simulink model "Sim118Bus_Sg"  (R2020b)
(part 1 of 2)
settings: Solver=FixedStepAuto  StartTime=0  StopTime=5  FixedStep=Ts  RelTol=1e-3
undefined symbols (not defined in the file or in its folder): ApparatusDiscreDamping, ApparatusPara, ApparatusPowerFlow, ApparatusType, Fbase, OtherInputs, Sbase, Ts, Vbase, Wbase, x_e, Ybase, Zbase
libraries: powerlib x486, SimplusGT x172
settings Model: Creator=admin_user  LastModifiedBy=admin_user

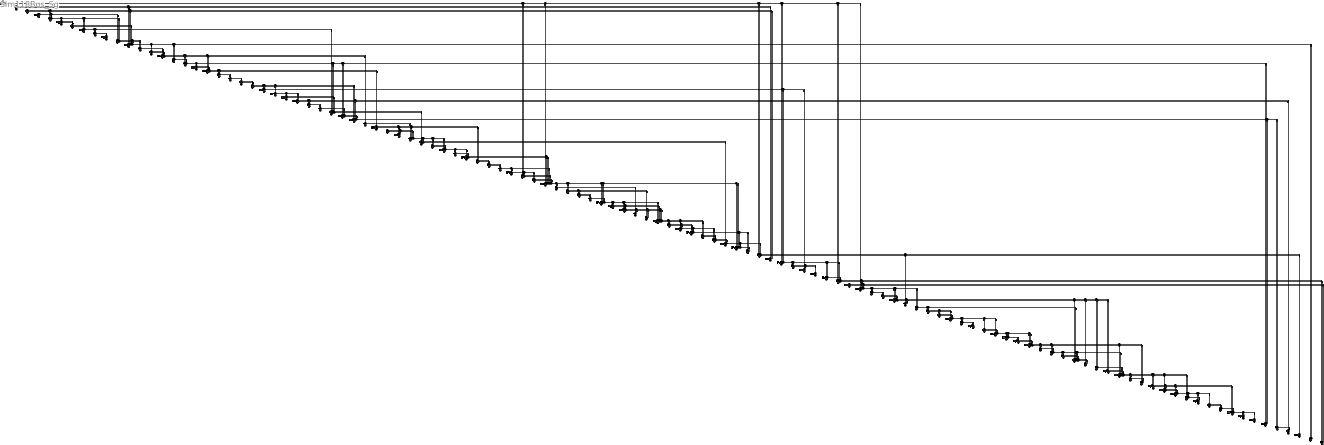
== system Sim118Bus_Sg ==
  B-GND{1,8,11,15,18,22,24,26,29,31..32,35,39,41,43,47,49,54,56,59,61,63,65,69,72,75,77,81,83,85,87,89,92,94,98,101..102,106,108,110,113,115,118,120,122,125,128,130,132,139,141,144,146,148,152,155,160..162,166,169,172,175,177,179,182,184..185,188..189,193,196..198,200,203,206,211,213,215,221..222,225,228,230,234,236..237,239,244,246,248,253,255,259,261,263..264,266,268,273,275..276,280,282,286,288..289,291,293,296..299,301..304} (118 alike) : powerlib/Elements/Ground  LConnTagsString=a
  Branch1-1 : powerlib/Elements/Three-Phase Parallel RLC Branch  LConnTagsString=A|B|C  RConnTagsString=A|B|C  BranchType=C  Resistance=(Inf)*Zbase  Inductance=(Inf)*Zbase/Wbase  Capacitance=(0.25176)*Ybase/Wbase  Measurements=None
      settings: SourceProductBaseCode=PS
  Branch1-47 : powerlib/Elements/Three-Phase Series RLC Branch  LConnTagsString=A|B|C  RConnTagsString=A|B|C  BranchType=RL  Resistance=(0.0844)*Zbase  Inductance=(0.2778)*Zbase/Wbase  Capacitance=1e-6  Measurements=None
  Branch1-49 : powerlib/Elements/Three-Phase Series RLC Branch  LConnTagsString=A|B|C  RConnTagsString=A|B|C  BranchType=RL  Resistance=(0.0985)*Zbase  Inductance=(0.324)*Zbase/Wbase  Capacitance=1e-6  Measurements=None
  Branch1-68 : powerlib/Elements/Three-Phase Series RLC Branch  LConnTagsString=A|B|C  RConnTagsString=A|B|C  BranchType=RL  Resistance=(0.0032346)*Zbase  Inductance=(0.032346)*Zbase/Wbase  Capacitance=1e-6  Measurements=None
  Branch1-70 : powerlib/Elements/Three-Phase Series RLC Branch  LConnTagsString=A|B|C  RConnTagsString=A|B|C  BranchType=RL  Resistance=(0.03)*Zbase  Inductance=(0.127)*Zbase/Wbase  Capacitance=1e-6  Measurements=None
  Branch1-75 : powerlib/Elements/Three-Phase Series RLC Branch  LConnTagsString=A|B|C  RConnTagsString=A|B|C  BranchType=RL  Resistance=(0.0405)*Zbase  Inductance=(0.122)*Zbase/Wbase  Capacitance=1e-6  Measurements=None
  Branch1-77 : powerlib/Elements/Three-Phase Series RLC Branch  LConnTagsString=A|B|C  RConnTagsString=A|B|C  BranchType=RL  Resistance=(0.0309)*Zbase  Inductance=(0.101)*Zbase/Wbase  Capacitance=1e-6  Measurements=None
  Branch10-10 : powerlib/Elements/Three-Phase Parallel RLC Branch  LConnTagsString=A|B|C  RConnTagsString=A|B|C  BranchType=C  Resistance=(Inf)*Zbase  Inductance=(Inf)*Zbase/Wbase  Capacitance=(0.615)*Ybase/Wbase  Measurements=None
      settings: SourceProductBaseCode=PS
  Branch100-100 : powerlib/Elements/Three-Phase Parallel RLC Branch  LConnTagsString=A|B|C  RConnTagsString=A|B|C  BranchType=RLC  Resistance=(2.7954)*Zbase  Inductance=(5.746)*Zbase/Wbase  Capacitance=(0.18965)*Ybase/Wbase  Measurements=None
      settings: SourceProductBaseCode=PS
  Branch100-101 : powerlib/Elements/Three-Phase Series RLC Branch  LConnTagsString=A|B|C  RConnTagsString=A|B|C  BranchType=RL  Resistance=(0.0277)*Zbase  Inductance=(0.1262)*Zbase/Wbase  Capacitance=1e-6  Measurements=None
  Branch100-103 : powerlib/Elements/Three-Phase Series RLC Branch  LConnTagsString=A|B|C  RConnTagsString=A|B|C  BranchType=RL  Resistance=(0.016)*Zbase  Inductance=(0.0525)*Zbase/Wbase  Capacitance=1e-6  Measurements=None
  Branch100-104 : powerlib/Elements/Three-Phase Series RLC Branch  LConnTagsString=A|B|C  RConnTagsString=A|B|C  BranchType=RL  Resistance=(0.0451)*Zbase  Inductance=(0.204)*Zbase/Wbase  Capacitance=1e-6  Measurements=None
  Branch100-106 : powerlib/Elements/Three-Phase Series RLC Branch  LConnTagsString=A|B|C  RConnTagsString=A|B|C  BranchType=RL  Resistance=(0.0605)*Zbase  Inductance=(0.229)*Zbase/Wbase  Capacitance=1e-6  Measurements=None
  Branch101-101 : powerlib/Elements/Three-Phase Parallel RLC Branch  LConnTagsString=A|B|C  RConnTagsString=A|B|C  BranchType=RLC  Resistance=(4.4798)*Zbase  Inductance=(6.5704)*Zbase/Wbase  Capacitance=(0.0311)*Ybase/Wbase  Measurements=None
      settings: SourceProductBaseCode=PS
  Branch101-102 : powerlib/Elements/Three-Phase Series RLC Branch  LConnTagsString=A|B|C  RConnTagsString=A|B|C  BranchType=RL  Resistance=(0.0246)*Zbase  Inductance=(0.112)*Zbase/Wbase  Capacitance=1e-6  Measurements=None
  Branch102-102 : powerlib/Elements/Three-Phase Parallel RLC Branch  LConnTagsString=A|B|C  RConnTagsString=A|B|C  BranchType=RLC  Resistance=(19.6651)*Zbase  Inductance=(32.7751)*Zbase/Wbase  Capacitance=(0.02202)*Ybase/Wbase  Measurements=None
      settings: SourceProductBaseCode=PS
  Branch103-103 : powerlib/Elements/Three-Phase Parallel RLC Branch  LConnTagsString=A|B|C  RConnTagsString=A|B|C  BranchType=RLC  Resistance=(4.2699)*Zbase  Inductance=(6.138)*Zbase/Wbase  Capacitance=(0.0906)*Ybase/Wbase  Measurements=None
      settings: SourceProductBaseCode=PS
  Branch103-104 : powerlib/Elements/Three-Phase Series RLC Branch  LConnTagsString=A|B|C  RConnTagsString=A|B|C  BranchType=RL  Resistance=(0.0466)*Zbase  Inductance=(0.1584)*Zbase/Wbase  Capacitance=1e-6  Measurements=None
  Branch103-105 : powerlib/Elements/Three-Phase Series RLC Branch  LConnTagsString=A|B|C  RConnTagsString=A|B|C  BranchType=RL  Resistance=(0.0535)*Zbase  Inductance=(0.1625)*Zbase/Wbase  Capacitance=1e-6  Measurements=None
  Branch103-110 : powerlib/Elements/Three-Phase Series RLC Branch  LConnTagsString=A|B|C  RConnTagsString=A|B|C  BranchType=RL  Resistance=(0.03906)*Zbase  Inductance=(0.1813)*Zbase/Wbase  Capacitance=1e-6  Measurements=None
  Branch104-104 : powerlib/Elements/Three-Phase Parallel RLC Branch  LConnTagsString=A|B|C  RConnTagsString=A|B|C  BranchType=RLC  Resistance=(2.4812)*Zbase  Inductance=(3.7714)*Zbase/Wbase  Capacitance=(0.05233)*Ybase/Wbase  Measurements=None
      settings: SourceProductBaseCode=PS
  Branch104-105 : powerlib/Elements/Three-Phase Series RLC Branch  LConnTagsString=A|B|C  RConnTagsString=A|B|C  BranchType=RL  Resistance=(0.00994)*Zbase  Inductance=(0.0378)*Zbase/Wbase  Capacitance=1e-6  Measurements=None
  Branch105-105 : powerlib/Elements/Three-Phase Parallel RLC Branch  LConnTagsString=A|B|C  RConnTagsString=A|B|C  BranchType=RLC  Resistance=(3.004)*Zbase  Inductance=(3.5816)*Zbase/Wbase  Capacitance=(0.06532)*Ybase/Wbase  Measurements=None
      settings: SourceProductBaseCode=PS
  Branch105-106 : powerlib/Elements/Three-Phase Series RLC Branch  LConnTagsString=A|B|C  RConnTagsString=A|B|C  BranchType=RL  Resistance=(0.014)*Zbase  Inductance=(0.0547)*Zbase/Wbase  Capacitance=1e-6  Measurements=None
  Branch105-107 : powerlib/Elements/Three-Phase Series RLC Branch  LConnTagsString=A|B|C  RConnTagsString=A|B|C  BranchType=RL  Resistance=(0.053)*Zbase  Inductance=(0.183)*Zbase/Wbase  Capacitance=1e-6  Measurements=None
  Branch105-108 : powerlib/Elements/Three-Phase Series RLC Branch  LConnTagsString=A|B|C  RConnTagsString=A|B|C  BranchType=RL  Resistance=(0.0261)*Zbase  Inductance=(0.0703)*Zbase/Wbase  Capacitance=1e-6  Measurements=None
  Branch106-106 : powerlib/Elements/Three-Phase Parallel RLC Branch  LConnTagsString=A|B|C  RConnTagsString=A|B|C  BranchType=RLC  Resistance=(2.1483)*Zbase  Inductance=(5.7735)*Zbase/Wbase  Capacitance=(0.06177)*Ybase/Wbase  Measurements=None
      settings: SourceProductBaseCode=PS
  Branch106-107 : powerlib/Elements/Three-Phase Series RLC Branch  LConnTagsString=A|B|C  RConnTagsString=A|B|C  BranchType=RL  Resistance=(0.053)*Zbase  Inductance=(0.183)*Zbase/Wbase  Capacitance=1e-6  Measurements=None
  Branch107-107 : powerlib/Elements/Three-Phase Parallel RLC Branch  LConnTagsString=A|B|C  RConnTagsString=A|B|C  BranchType=RLC  Resistance=(3.2368)*Zbase  Inductance=(7.5525)*Zbase/Wbase  Capacitance=(0.0472)*Ybase/Wbase  Measurements=None
      settings: SourceProductBaseCode=PS
  Branch108-108 : powerlib/Elements/Three-Phase Parallel RLC Branch  LConnTagsString=A|B|C  RConnTagsString=A|B|C  BranchType=RLC  Resistance=(46.6783)*Zbase  Inductance=(93.3565)*Zbase/Wbase  Capacitance=(0.01302)*Ybase/Wbase  Measurements=None
      settings: SourceProductBaseCode=PS
  Branch108-109 : powerlib/Elements/Three-Phase Series RLC Branch  LConnTagsString=A|B|C  RConnTagsString=A|B|C  BranchType=RL  Resistance=(0.0105)*Zbase  Inductance=(0.0288)*Zbase/Wbase  Capacitance=1e-6  Measurements=None
  Branch109-109 : powerlib/Elements/Three-Phase Parallel RLC Branch  LConnTagsString=A|B|C  RConnTagsString=A|B|C  BranchType=RLC  Resistance=(11.6892)*Zbase  Inductance=(31.1713)*Zbase/Wbase  Capacitance=(0.0139)*Ybase/Wbase  Measurements=None
      settings: SourceProductBaseCode=PS
  Branch109-110 : powerlib/Elements/Three-Phase Series RLC Branch  LConnTagsString=A|B|C  RConnTagsString=A|B|C  BranchType=RL  Resistance=(0.0278)*Zbase  Inductance=(0.0762)*Zbase/Wbase  Capacitance=1e-6  Measurements=None
  Branch11-11 : powerlib/Elements/Three-Phase Parallel RLC Branch  LConnTagsString=A|B|C  RConnTagsString=A|B|C  BranchType=RLC  Resistance=(1.3865)*Zbase  Inductance=(4.2197)*Zbase/Wbase  Capacitance=(0.02932)*Ybase/Wbase  Measurements=None
      settings: SourceProductBaseCode=PS
  Branch11-12 : powerlib/Elements/Three-Phase Series RLC Branch  LConnTagsString=A|B|C  RConnTagsString=A|B|C  BranchType=RL  Resistance=(0.00595)*Zbase  Inductance=(0.0196)*Zbase/Wbase  Capacitance=1e-6  Measurements=None
  Branch11-13 : powerlib/Elements/Three-Phase Series RLC Branch  LConnTagsString=A|B|C  RConnTagsString=A|B|C  BranchType=RL  Resistance=(0.02225)*Zbase  Inductance=(0.0731)*Zbase/Wbase  Capacitance=1e-6  Measurements=None
  Branch110-110 : powerlib/Elements/Three-Phase Parallel RLC Branch  LConnTagsString=A|B|C  RConnTagsString=A|B|C  BranchType=RLC  Resistance=(2.4275)*Zbase  Inductance=(3.1558)*Zbase/Wbase  Capacitance=(0.07415)*Ybase/Wbase  Measurements=None
      settings: SourceProductBaseCode=PS
  Branch110-111 : powerlib/Elements/Three-Phase Series RLC Branch  LConnTagsString=A|B|C  RConnTagsString=A|B|C  BranchType=RL  Resistance=(0.022)*Zbase  Inductance=(0.0755)*Zbase/Wbase  Capacitance=1e-6  Measurements=None
  Branch110-112 : powerlib/Elements/Three-Phase Series RLC Branch  LConnTagsString=A|B|C  RConnTagsString=A|B|C  BranchType=RL  Resistance=(0.0247)*Zbase  Inductance=(0.064)*Zbase/Wbase  Capacitance=1e-6  Measurements=None
  Branch111-111 : powerlib/Elements/Three-Phase Parallel RLC Branch  LConnTagsString=A|B|C  RConnTagsString=A|B|C  BranchType=C  Resistance=(Inf)*Zbase  Inductance=(Inf)*Zbase/Wbase  Capacitance=(0.01)*Ybase/Wbase  Measurements=None
      settings: SourceProductBaseCode=PS
  Branch112-112 : powerlib/Elements/Three-Phase Parallel RLC Branch  LConnTagsString=A|B|C  RConnTagsString=A|B|C  BranchType=RLC  Resistance=(3.8025)*Zbase  Inductance=(7.3125)*Zbase/Wbase  Capacitance=(0.031)*Ybase/Wbase  Measurements=None
      settings: SourceProductBaseCode=PS
  Branch113-113 : powerlib/Elements/Three-Phase Parallel RLC Branch  LConnTagsString=A|B|C  RConnTagsString=A|B|C  BranchType=C  Resistance=(Inf)*Zbase  Inductance=(Inf)*Zbase/Wbase  Capacitance=(0.02974)*Ybase/Wbase  Measurements=None
      settings: SourceProductBaseCode=PS
  Branch114-114 : powerlib/Elements/Three-Phase Parallel RLC Branch  LConnTagsString=A|B|C  RConnTagsString=A|B|C  BranchType=RLC  Resistance=(11.5362)*Zbase  Inductance=(30.7633)*Zbase/Wbase  Capacitance=(0.00952)*Ybase/Wbase  Measurements=None
      settings: SourceProductBaseCode=PS
  Branch114-115 : powerlib/Elements/Three-Phase Series RLC Branch  LConnTagsString=A|B|C  RConnTagsString=A|B|C  BranchType=RL  Resistance=(0.0023)*Zbase  Inductance=(0.0104)*Zbase/Wbase  Capacitance=1e-6  Measurements=None
  Branch115-115 : powerlib/Elements/Three-Phase Parallel RLC Branch  LConnTagsString=A|B|C  RConnTagsString=A|B|C  BranchType=RLC  Resistance=(4.1938)*Zbase  Inductance=(13.1804)*Zbase/Wbase  Capacitance=(0.01124)*Ybase/Wbase  Measurements=None
      settings: SourceProductBaseCode=PS
  Branch116-116 : powerlib/Elements/Three-Phase Parallel RLC Branch  LConnTagsString=A|B|C  RConnTagsString=A|B|C  BranchType=C  Resistance=(Inf)*Zbase  Inductance=(Inf)*Zbase/Wbase  Capacitance=(0.082)*Ybase/Wbase  Measurements=None
      settings: SourceProductBaseCode=PS
  Branch117-117 : powerlib/Elements/Three-Phase Parallel RLC Branch  LConnTagsString=A|B|C  RConnTagsString=A|B|C  BranchType=RLC  Resistance=(4.7417)*Zbase  Inductance=(11.8542)*Zbase/Wbase  Capacitance=(0.0179)*Ybase/Wbase  Measurements=None
      settings: SourceProductBaseCode=PS
  Branch118-118 : powerlib/Elements/Three-Phase Parallel RLC Branch  LConnTagsString=A|B|C  RConnTagsString=A|B|C  BranchType=RLC  Resistance=(2.7315)*Zbase  Inductance=(6.0093)*Zbase/Wbase  Capacitance=(0.01277)*Ybase/Wbase  Measurements=None
      settings: SourceProductBaseCode=PS
  Branch12-117 : powerlib/Elements/Three-Phase Series RLC Branch  LConnTagsString=A|B|C  RConnTagsString=A|B|C  BranchType=RL  Resistance=(0.0329)*Zbase  Inductance=(0.14)*Zbase/Wbase  Capacitance=1e-6  Measurements=None
  Branch12-12 : powerlib/Elements/Three-Phase Parallel RLC Branch  LConnTagsString=A|B|C  RConnTagsString=A|B|C  BranchType=RLC  Resistance=(2.0853)*Zbase  Inductance=(9.801)*Zbase/Wbase  Capacitance=(0.07272)*Ybase/Wbase  Measurements=None
      settings: SourceProductBaseCode=PS
  Branch12-14 : powerlib/Elements/Three-Phase Series RLC Branch  LConnTagsString=A|B|C  RConnTagsString=A|B|C  BranchType=RL  Resistance=(0.0215)*Zbase  Inductance=(0.0707)*Zbase/Wbase  Capacitance=1e-6  Measurements=None
  Branch12-16 : powerlib/Elements/Three-Phase Series RLC Branch  LConnTagsString=A|B|C  RConnTagsString=A|B|C  BranchType=RL  Resistance=(0.0212)*Zbase  Inductance=(0.0834)*Zbase/Wbase  Capacitance=1e-6  Measurements=None
  Branch13-13 : powerlib/Elements/Three-Phase Parallel RLC Branch  LConnTagsString=A|B|C  RConnTagsString=A|B|C  BranchType=RLC  Resistance=(2.758)*Zbase  Inductance=(5.8608)*Zbase/Wbase  Capacitance=(0.04072)*Ybase/Wbase  Measurements=None
      settings: SourceProductBaseCode=PS
  Branch13-15 : powerlib/Elements/Three-Phase Series RLC Branch  LConnTagsString=A|B|C  RConnTagsString=A|B|C  BranchType=RL  Resistance=(0.0744)*Zbase  Inductance=(0.2444)*Zbase/Wbase  Capacitance=1e-6  Measurements=None
  Branch14-14 : powerlib/Elements/Three-Phase Parallel RLC Branch  LConnTagsString=A|B|C  RConnTagsString=A|B|C  BranchType=RLC  Resistance=(6.9104)*Zbase  Inductance=(96.746)*Zbase/Wbase  Capacitance=(0.03418)*Ybase/Wbase  Measurements=None
      settings: SourceProductBaseCode=PS
  Branch14-15 : powerlib/Elements/Three-Phase Series RLC Branch  LConnTagsString=A|B|C  RConnTagsString=A|B|C  BranchType=RL  Resistance=(0.0595)*Zbase  Inductance=(0.195)*Zbase/Wbase  Capacitance=1e-6  Measurements=None
  Branch15-15 : powerlib/Elements/Three-Phase Parallel RLC Branch  LConnTagsString=A|B|C  RConnTagsString=A|B|C  BranchType=RLC  Resistance=(1.0454)*Zbase  Inductance=(3.1363)*Zbase/Wbase  Capacitance=(0.09966)*Ybase/Wbase  Measurements=None
      settings: SourceProductBaseCode=PS
  Branch15-17 : powerlib/Elements/Three-Phase Series RLC Branch  LConnTagsString=A|B|C  RConnTagsString=A|B|C  BranchType=RL  Resistance=(0.0132)*Zbase  Inductance=(0.0437)*Zbase/Wbase  Capacitance=1e-6  Measurements=None
  Branch15-19 : powerlib/Elements/Three-Phase Series RLC Branch  LConnTagsString=A|B|C  RConnTagsString=A|B|C  BranchType=RL  Resistance=(0.012)*Zbase  Inductance=(0.0394)*Zbase/Wbase  Capacitance=1e-6  Measurements=None
  Branch15-33 : powerlib/Elements/Three-Phase Series RLC Branch  LConnTagsString=A|B|C  RConnTagsString=A|B|C  BranchType=RL  Resistance=(0.038)*Zbase  Inductance=(0.1244)*Zbase/Wbase  Capacitance=1e-6  Measurements=None
  Branch16-16 : powerlib/Elements/Three-Phase Parallel RLC Branch  LConnTagsString=A|B|C  RConnTagsString=A|B|C  BranchType=RLC  Resistance=(3.8697)*Zbase  Inductance=(9.6743)*Zbase/Wbase  Capacitance=(0.034)*Ybase/Wbase  Measurements=None
      settings: SourceProductBaseCode=PS
  Branch16-17 : powerlib/Elements/Three-Phase Series RLC Branch  LConnTagsString=A|B|C  RConnTagsString=A|B|C  BranchType=RL  Resistance=(0.0454)*Zbase  Inductance=(0.1801)*Zbase/Wbase  Capacitance=1e-6  Measurements=None
  Branch17-113 : powerlib/Elements/Three-Phase Series RLC Branch  LConnTagsString=A|B|C  RConnTagsString=A|B|C  BranchType=RL  Resistance=(0.00913)*Zbase  Inductance=(0.0301)*Zbase/Wbase  Capacitance=1e-6  Measurements=None
  Branch17-17 : powerlib/Elements/Three-Phase Parallel RLC Branch  LConnTagsString=A|B|C  RConnTagsString=A|B|C  BranchType=RLC  Resistance=(8.9844)*Zbase  Inductance=(32.9429)*Zbase/Wbase  Capacitance=(0.07578)*Ybase/Wbase  Measurements=None
      settings: SourceProductBaseCode=PS
  Branch17-18 : powerlib/Elements/Three-Phase Series RLC Branch  LConnTagsString=A|B|C  RConnTagsString=A|B|C  BranchType=RL  Resistance=(0.0123)*Zbase  Inductance=(0.0505)*Zbase/Wbase  Capacitance=1e-6  Measurements=None
  Branch17-30 : powerlib/Elements/Three-Phase Series RLC Branch  LConnTagsString=A|B|C  RConnTagsString=A|B|C  BranchType=RL  Resistance=(0.0035758)*Zbase  Inductance=(0.035758)*Zbase/Wbase  Capacitance=1e-6  Measurements=None
  Branch17-31 : powerlib/Elements/Three-Phase Series RLC Branch  LConnTagsString=A|B|C  RConnTagsString=A|B|C  BranchType=RL  Resistance=(0.0474)*Zbase  Inductance=(0.1563)*Zbase/Wbase  Capacitance=1e-6  Measurements=None
  Branch18-18 : powerlib/Elements/Three-Phase Parallel RLC Branch  LConnTagsString=A|B|C  RConnTagsString=A|B|C  BranchType=RLC  Resistance=(1.5779)*Zbase  Inductance=(2.7845)*Zbase/Wbase  Capacitance=(0.0122)*Ybase/Wbase  Measurements=None
      settings: SourceProductBaseCode=PS
  Branch18-19 : powerlib/Elements/Three-Phase Series RLC Branch  LConnTagsString=A|B|C  RConnTagsString=A|B|C  BranchType=RL  Resistance=(0.01119)*Zbase  Inductance=(0.0493)*Zbase/Wbase  Capacitance=1e-6  Measurements=None
  Branch19-19 : powerlib/Elements/Three-Phase Parallel RLC Branch  LConnTagsString=A|B|C  RConnTagsString=A|B|C  BranchType=RLC  Resistance=(2.1038)*Zbase  Inductance=(3.7869)*Zbase/Wbase  Capacitance=(0.05726)*Ybase/Wbase  Measurements=None
      settings: SourceProductBaseCode=PS
  Branch19-20 : powerlib/Elements/Three-Phase Series RLC Branch  LConnTagsString=A|B|C  RConnTagsString=A|B|C  BranchType=RL  Resistance=(0.0252)*Zbase  Inductance=(0.117)*Zbase/Wbase  Capacitance=1e-6  Measurements=None
  Branch19-34 : powerlib/Elements/Three-Phase Series RLC Branch  LConnTagsString=A|B|C  RConnTagsString=A|B|C  BranchType=RL  Resistance=(0.0752)*Zbase  Inductance=(0.247)*Zbase/Wbase  Capacitance=1e-6  Measurements=None
  Branch2-12 : powerlib/Elements/Three-Phase Series RLC Branch  LConnTagsString=A|B|C  RConnTagsString=A|B|C  BranchType=RL  Resistance=(0.0187)*Zbase  Inductance=(0.0616)*Zbase/Wbase  Capacitance=1e-6  Measurements=None
  Branch2-2 : powerlib/Elements/Three-Phase Parallel RLC Branch  LConnTagsString=A|B|C  RConnTagsString=A|B|C  BranchType=RLC  Resistance=(4.718)*Zbase  Inductance=(10.4845)*Zbase/Wbase  Capacitance=(0.02056)*Ybase/Wbase  Measurements=None
      settings: SourceProductBaseCode=PS
  Branch2-69 : powerlib/Elements/Three-Phase Series RLC Branch  LConnTagsString=A|B|C  RConnTagsString=A|B|C  BranchType=RL  Resistance=(0.0303)*Zbase  Inductance=(0.0999)*Zbase/Wbase  Capacitance=1e-6  Measurements=None
  Branch20-20 : powerlib/Elements/Three-Phase Parallel RLC Branch  LConnTagsString=A|B|C  RConnTagsString=A|B|C  BranchType=RLC  Resistance=(5.1775)*Zbase  Inductance=(31.0651)*Zbase/Wbase  Capacitance=(0.0257)*Ybase/Wbase  Measurements=None
      settings: SourceProductBaseCode=PS
  Branch20-21 : powerlib/Elements/Three-Phase Series RLC Branch  LConnTagsString=A|B|C  RConnTagsString=A|B|C  BranchType=RL  Resistance=(0.0183)*Zbase  Inductance=(0.0849)*Zbase/Wbase  Capacitance=1e-6  Measurements=None
  Branch21-21 : powerlib/Elements/Three-Phase Parallel RLC Branch  LConnTagsString=A|B|C  RConnTagsString=A|B|C  BranchType=RLC  Resistance=(6.6415)*Zbase  Inductance=(11.6226)*Zbase/Wbase  Capacitance=(0.0231)*Ybase/Wbase  Measurements=None
      settings: SourceProductBaseCode=PS
  Branch21-22 : powerlib/Elements/Three-Phase Series RLC Branch  LConnTagsString=A|B|C  RConnTagsString=A|B|C  BranchType=RL  Resistance=(0.0209)*Zbase  Inductance=(0.097)*Zbase/Wbase  Capacitance=1e-6  Measurements=None
  Branch22-22 : powerlib/Elements/Three-Phase Parallel RLC Branch  LConnTagsString=A|B|C  RConnTagsString=A|B|C  BranchType=RLC  Resistance=(9.4738)*Zbase  Inductance=(18.9476)*Zbase/Wbase  Capacitance=(0.0325)*Ybase/Wbase  Measurements=None
      settings: SourceProductBaseCode=PS
  Branch22-23 : powerlib/Elements/Three-Phase Series RLC Branch  LConnTagsString=A|B|C  RConnTagsString=A|B|C  BranchType=RL  Resistance=(0.0342)*Zbase  Inductance=(0.159)*Zbase/Wbase  Capacitance=1e-6  Measurements=None
  Branch23-23 : powerlib/Elements/Three-Phase Parallel RLC Branch  LConnTagsString=A|B|C  RConnTagsString=A|B|C  BranchType=RLC  Resistance=(14.2915)*Zbase  Inductance=(33.3469)*Zbase/Wbase  Capacitance=(0.14695)*Ybase/Wbase  Measurements=None
      settings: SourceProductBaseCode=PS
  Branch23-24 : powerlib/Elements/Three-Phase Series RLC Branch  LConnTagsString=A|B|C  RConnTagsString=A|B|C  BranchType=RL  Resistance=(0.0135)*Zbase  Inductance=(0.0492)*Zbase/Wbase  Capacitance=1e-6  Measurements=None
  Branch23-25 : powerlib/Elements/Three-Phase Series RLC Branch  LConnTagsString=A|B|C  RConnTagsString=A|B|C  BranchType=RL  Resistance=(0.0156)*Zbase  Inductance=(0.08)*Zbase/Wbase  Capacitance=1e-6  Measurements=None
  Branch23-32 : powerlib/Elements/Three-Phase Series RLC Branch  LConnTagsString=A|B|C  RConnTagsString=A|B|C  BranchType=RL  Resistance=(0.0317)*Zbase  Inductance=(0.1153)*Zbase/Wbase  Capacitance=1e-6  Measurements=None
  Branch24-24 : powerlib/Elements/Three-Phase Parallel RLC Branch  LConnTagsString=A|B|C  RConnTagsString=A|B|C  BranchType=C  Resistance=(Inf)*Zbase  Inductance=(Inf)*Zbase/Wbase  Capacitance=(0.10029)*Ybase/Wbase  Measurements=None
      settings: SourceProductBaseCode=PS
  Branch24-70 : powerlib/Elements/Three-Phase Series RLC Branch  LConnTagsString=A|B|C  RConnTagsString=A|B|C  BranchType=RL  Resistance=(0.00221)*Zbase  Inductance=(0.4115)*Zbase/Wbase  Capacitance=1e-6  Measurements=None
  Branch24-72 : powerlib/Elements/Three-Phase Series RLC Branch  LConnTagsString=A|B|C  RConnTagsString=A|B|C  BranchType=RL  Resistance=(0.0488)*Zbase  Inductance=(0.196)*Zbase/Wbase  Capacitance=1e-6  Measurements=None
  Branch25-25 : powerlib/Elements/Three-Phase Parallel RLC Branch  LConnTagsString=A|B|C  RConnTagsString=A|B|C  BranchType=C  Resistance=(Inf)*Zbase  Inductance=(Inf)*Zbase/Wbase  Capacitance=(0.1314)*Ybase/Wbase  Measurements=None
      settings: SourceProductBaseCode=PS
  Branch25-26 : powerlib/Elements/Three-Phase Series RLC Branch  LConnTagsString=A|B|C  RConnTagsString=A|B|C  BranchType=RL  Resistance=(0.0035205)*Zbase  Inductance=(0.035205)*Zbase/Wbase  Capacitance=1e-6  Measurements=None
  Branch25-27 : powerlib/Elements/Three-Phase Series RLC Branch  LConnTagsString=A|B|C  RConnTagsString=A|B|C  BranchType=RL  Resistance=(0.0318)*Zbase  Inductance=(0.163)*Zbase/Wbase  Capacitance=1e-6  Measurements=None
  Branch26-26 : powerlib/Elements/Three-Phase Parallel RLC Branch  LConnTagsString=A|B|C  RConnTagsString=A|B|C  BranchType=C  Resistance=(Inf)*Zbase  Inductance=(Inf)*Zbase/Wbase  Capacitance=(0.454)*Ybase/Wbase  Measurements=None
      settings: SourceProductBaseCode=PS
  Branch26-30 : powerlib/Elements/Three-Phase Series RLC Branch  LConnTagsString=A|B|C  RConnTagsString=A|B|C  BranchType=RL  Resistance=(0.00799)*Zbase  Inductance=(0.086)*Zbase/Wbase  Capacitance=1e-6  Measurements=None
  Branch27-115 : powerlib/Elements/Three-Phase Series RLC Branch  LConnTagsString=A|B|C  RConnTagsString=A|B|C  BranchType=RL  Resistance=(0.0164)*Zbase  Inductance=(0.0741)*Zbase/Wbase  Capacitance=1e-6  Measurements=None
  Branch27-27 : powerlib/Elements/Three-Phase Parallel RLC Branch  LConnTagsString=A|B|C  RConnTagsString=A|B|C  BranchType=RLC  Resistance=(1.5113)*Zbase  Inductance=(7.2079)*Zbase/Wbase  Capacitance=(0.11849)*Ybase/Wbase  Measurements=None
      settings: SourceProductBaseCode=PS
  Branch27-28 : powerlib/Elements/Three-Phase Series RLC Branch  LConnTagsString=A|B|C  RConnTagsString=A|B|C  BranchType=RL  Resistance=(0.01913)*Zbase  Inductance=(0.0855)*Zbase/Wbase  Capacitance=1e-6  Measurements=None
  Branch27-32 : powerlib/Elements/Three-Phase Series RLC Branch  LConnTagsString=A|B|C  RConnTagsString=A|B|C  BranchType=RL  Resistance=(0.0229)*Zbase  Inductance=(0.0755)*Zbase/Wbase  Capacitance=1e-6  Measurements=None
  Branch28-28 : powerlib/Elements/Three-Phase Parallel RLC Branch  LConnTagsString=A|B|C  RConnTagsString=A|B|C  BranchType=RLC  Resistance=(5.4389)*Zbase  Inductance=(13.2088)*Zbase/Wbase  Capacitance=(0.0227)*Ybase/Wbase  Measurements=None
      settings: SourceProductBaseCode=PS
  Branch28-29 : powerlib/Elements/Three-Phase Series RLC Branch  LConnTagsString=A|B|C  RConnTagsString=A|B|C  BranchType=RL  Resistance=(0.0237)*Zbase  Inductance=(0.0943)*Zbase/Wbase  Capacitance=1e-6  Measurements=None
  Branch29-29 : powerlib/Elements/Three-Phase Parallel RLC Branch  LConnTagsString=A|B|C  RConnTagsString=A|B|C  BranchType=RLC  Resistance=(3.8658)*Zbase  Inductance=(23.1946)*Zbase/Wbase  Capacitance=(0.01605)*Ybase/Wbase  Measurements=None
      settings: SourceProductBaseCode=PS
  Branch29-31 : powerlib/Elements/Three-Phase Series RLC Branch  LConnTagsString=A|B|C  RConnTagsString=A|B|C  BranchType=RL  Resistance=(0.0108)*Zbase  Inductance=(0.0331)*Zbase/Wbase  Capacitance=1e-6  Measurements=None
  Branch3-12 : powerlib/Elements/Three-Phase Series RLC Branch  LConnTagsString=A|B|C  RConnTagsString=A|B|C  BranchType=RL  Resistance=(0.0484)*Zbase  Inductance=(0.16)*Zbase/Wbase  Capacitance=1e-6  Measurements=None
  Branch3-3 : powerlib/Elements/Three-Phase Parallel RLC Branch  LConnTagsString=A|B|C  RConnTagsString=A|B|C  BranchType=RLC  Resistance=(2.4015)*Zbase  Inductance=(9.3659)*Zbase/Wbase  Capacitance=(0.03991)*Ybase/Wbase  Measurements=None
      settings: SourceProductBaseCode=PS
  Branch3-5 : powerlib/Elements/Three-Phase Series RLC Branch  LConnTagsString=A|B|C  RConnTagsString=A|B|C  BranchType=RL  Resistance=(0.0241)*Zbase  Inductance=(0.108)*Zbase/Wbase  Capacitance=1e-6  Measurements=None
  Branch3-69 : powerlib/Elements/Three-Phase Series RLC Branch  LConnTagsString=A|B|C  RConnTagsString=A|B|C  BranchType=RL  Resistance=(0.0129)*Zbase  Inductance=(0.0424)*Zbase/Wbase  Capacitance=1e-6  Measurements=None
  Branch30-30 : powerlib/Elements/Three-Phase Parallel RLC Branch  LConnTagsString=A|B|C  RConnTagsString=A|B|C  BranchType=C  Resistance=(Inf)*Zbase  Inductance=(Inf)*Zbase/Wbase  Capacitance=(0.922)*Ybase/Wbase  Measurements=None
      settings: SourceProductBaseCode=PS
  Branch30-38 : powerlib/Elements/Three-Phase Series RLC Branch  LConnTagsString=A|B|C  RConnTagsString=A|B|C  BranchType=RL  Resistance=(0.00464)*Zbase  Inductance=(0.054)*Zbase/Wbase  Capacitance=1e-6  Measurements=None
  Branch31-31 : powerlib/Elements/Three-Phase Parallel RLC Branch  LConnTagsString=A|B|C  RConnTagsString=A|B|C  BranchType=RLC  Resistance=(2.1746)*Zbase  Inductance=(3.4633)*Zbase/Wbase  Capacitance=(0.03665)*Ybase/Wbase  Measurements=None
      settings: SourceProductBaseCode=PS
  Branch31-32 : powerlib/Elements/Three-Phase Series RLC Branch  LConnTagsString=A|B|C  RConnTagsString=A|B|C  BranchType=RL  Resistance=(0.0298)*Zbase  Inductance=(0.0985)*Zbase/Wbase  Capacitance=1e-6  Measurements=None
  Branch32-113 : powerlib/Elements/Three-Phase Series RLC Branch  LConnTagsString=A|B|C  RConnTagsString=A|B|C  BranchType=RL  Resistance=(0.0615)*Zbase  Inductance=(0.203)*Zbase/Wbase  Capacitance=1e-6  Measurements=None
  Branch32-114 : powerlib/Elements/Three-Phase Series RLC Branch  LConnTagsString=A|B|C  RConnTagsString=A|B|C  BranchType=RL  Resistance=(0.0135)*Zbase  Inductance=(0.0612)*Zbase/Wbase  Capacitance=1e-6  Measurements=None
  Branch32-32 : powerlib/Elements/Three-Phase Parallel RLC Branch  LConnTagsString=A|B|C  RConnTagsString=A|B|C  BranchType=RLC  Resistance=(1.5751)*Zbase  Inductance=(4.0404)*Zbase/Wbase  Capacitance=(0.11487)*Ybase/Wbase  Measurements=None
      settings: SourceProductBaseCode=PS
  Branch33-33 : powerlib/Elements/Three-Phase Parallel RLC Branch  LConnTagsString=A|B|C  RConnTagsString=A|B|C  BranchType=RLC  Resistance=(4.109)*Zbase  Inductance=(10.5009)*Zbase/Wbase  Capacitance=(0.03427)*Ybase/Wbase  Measurements=None
      settings: SourceProductBaseCode=PS
  Branch33-37 : powerlib/Elements/Three-Phase Series RLC Branch  LConnTagsString=A|B|C  RConnTagsString=A|B|C  BranchType=RL  Resistance=(0.0415)*Zbase  Inductance=(0.142)*Zbase/Wbase  Capacitance=1e-6  Measurements=None
  Branch34-34 : powerlib/Elements/Three-Phase Parallel RLC Branch  LConnTagsString=A|B|C  RConnTagsString=A|B|C  BranchType=RLC  Resistance=(1.6478)*Zbase  Inductance=(3.7392)*Zbase/Wbase  Capacitance=(0.06049)*Ybase/Wbase  Measurements=None
      settings: SourceProductBaseCode=PS
  Branch34-36 : powerlib/Elements/Three-Phase Series RLC Branch  LConnTagsString=A|B|C  RConnTagsString=A|B|C  BranchType=RL  Resistance=(0.00871)*Zbase  Inductance=(0.0268)*Zbase/Wbase  Capacitance=1e-6  Measurements=None
  Branch34-37 : powerlib/Elements/Three-Phase Series RLC Branch  LConnTagsString=A|B|C  RConnTagsString=A|B|C  BranchType=RL  Resistance=(0.00256)*Zbase  Inductance=(0.0094)*Zbase/Wbase  Capacitance=1e-6  Measurements=None
  Branch34-43 : powerlib/Elements/Three-Phase Series RLC Branch  LConnTagsString=A|B|C  RConnTagsString=A|B|C  BranchType=RL  Resistance=(0.0413)*Zbase  Inductance=(0.1681)*Zbase/Wbase  Capacitance=1e-6  Measurements=None
  Branch35-35 : powerlib/Elements/Three-Phase Parallel RLC Branch  LConnTagsString=A|B|C  RConnTagsString=A|B|C  BranchType=RLC  Resistance=(2.9156)*Zbase  Inductance=(10.6905)*Zbase/Wbase  Capacitance=(0.00793)*Ybase/Wbase  Measurements=None
      settings: SourceProductBaseCode=PS
  Branch35-36 : powerlib/Elements/Three-Phase Series RLC Branch  LConnTagsString=A|B|C  RConnTagsString=A|B|C  BranchType=RL  Resistance=(0.00224)*Zbase  Inductance=(0.0102)*Zbase/Wbase  Capacitance=1e-6  Measurements=None
  Branch35-37 : powerlib/Elements/Three-Phase Series RLC Branch  LConnTagsString=A|B|C  RConnTagsString=A|B|C  BranchType=RL  Resistance=(0.011)*Zbase  Inductance=(0.0497)*Zbase/Wbase  Capacitance=1e-6  Measurements=None
  Branch36-36 : powerlib/Elements/Three-Phase Parallel RLC Branch  LConnTagsString=A|B|C  RConnTagsString=A|B|C  BranchType=RLC  Resistance=(3.0981)*Zbase  Inductance=(5.6494)*Zbase/Wbase  Capacitance=(0.00418)*Ybase/Wbase  Measurements=None
      settings: SourceProductBaseCode=PS
  Branch37-37 : powerlib/Elements/Three-Phase Parallel RLC Branch  LConnTagsString=A|B|C  RConnTagsString=A|B|C  BranchType=C  Resistance=(Inf)*Zbase  Inductance=(Inf)*Zbase/Wbase  Capacitance=(0.06431)*Ybase/Wbase  Measurements=None
      settings: SourceProductBaseCode=PS
  Branch37-38 : powerlib/Elements/Three-Phase Series RLC Branch  LConnTagsString=A|B|C  RConnTagsString=A|B|C  BranchType=RL  Resistance=(0.0032783)*Zbase  Inductance=(0.032783)*Zbase/Wbase  Capacitance=1e-6  Measurements=None
  Branch37-39 : powerlib/Elements/Three-Phase Series RLC Branch  LConnTagsString=A|B|C  RConnTagsString=A|B|C  BranchType=RL  Resistance=(0.0321)*Zbase  Inductance=(0.106)*Zbase/Wbase  Capacitance=1e-6  Measurements=None
  Branch37-40 : powerlib/Elements/Three-Phase Series RLC Branch  LConnTagsString=A|B|C  RConnTagsString=A|B|C  BranchType=RL  Resistance=(0.0593)*Zbase  Inductance=(0.168)*Zbase/Wbase  Capacitance=1e-6  Measurements=None
  Branch38-38 : powerlib/Elements/Three-Phase Parallel RLC Branch  LConnTagsString=A|B|C  RConnTagsString=A|B|C  BranchType=C  Resistance=(Inf)*Zbase  Inductance=(Inf)*Zbase/Wbase  Capacitance=(0.734)*Ybase/Wbase  Measurements=None
      settings: SourceProductBaseCode=PS
  Branch38-65 : powerlib/Elements/Three-Phase Series RLC Branch  LConnTagsString=A|B|C  RConnTagsString=A|B|C  BranchType=RL  Resistance=(0.00901)*Zbase  Inductance=(0.0986)*Zbase/Wbase  Capacitance=1e-6  Measurements=None
  Branch39-39 : powerlib/Elements/Three-Phase Parallel RLC Branch  LConnTagsString=A|B|C  RConnTagsString=A|B|C  BranchType=RLC  Resistance=(3.4915)*Zbase  Inductance=(8.5701)*Zbase/Wbase  Capacitance=(0.02126)*Ybase/Wbase  Measurements=None
      settings: SourceProductBaseCode=PS
  Branch39-40 : powerlib/Elements/Three-Phase Series RLC Branch  LConnTagsString=A|B|C  RConnTagsString=A|B|C  BranchType=RL  Resistance=(0.0184)*Zbase  Inductance=(0.0605)*Zbase/Wbase  Capacitance=1e-6  Measurements=None
  Branch4-11 : powerlib/Elements/Three-Phase Series RLC Branch  LConnTagsString=A|B|C  RConnTagsString=A|B|C  BranchType=RL  Resistance=(0.0209)*Zbase  Inductance=(0.0688)*Zbase/Wbase  Capacitance=1e-6  Measurements=None
  Branch4-4 : powerlib/Elements/Three-Phase Parallel RLC Branch  LConnTagsString=A|B|C  RConnTagsString=A|B|C  BranchType=RLC  Resistance=(3.32)*Zbase  Inductance=(8.3)*Zbase/Wbase  Capacitance=(0.00979)*Ybase/Wbase  Measurements=None
      settings: SourceProductBaseCode=PS
  Branch4-5 : powerlib/Elements/Three-Phase Series RLC Branch  LConnTagsString=A|B|C  RConnTagsString=A|B|C  BranchType=RL  Resistance=(0.00176)*Zbase  Inductance=(0.00798)*Zbase/Wbase  Capacitance=1e-6  Measurements=None
  Branch40-40 : powerlib/Elements/Three-Phase Parallel RLC Branch  LConnTagsString=A|B|C  RConnTagsString=A|B|C  BranchType=RLC  Resistance=(4.7045)*Zbase  Inductance=(4.0909)*Zbase/Wbase  Capacitance=(0.05817)*Ybase/Wbase  Measurements=None
      settings: SourceProductBaseCode=PS
  Branch40-41 : powerlib/Elements/Three-Phase Series RLC Branch  LConnTagsString=A|B|C  RConnTagsString=A|B|C  BranchType=RL  Resistance=(0.0145)*Zbase  Inductance=(0.0487)*Zbase/Wbase  Capacitance=1e-6  Measurements=None
  Branch40-42 : powerlib/Elements/Three-Phase Series RLC Branch  LConnTagsString=A|B|C  RConnTagsString=A|B|C  BranchType=RL  Resistance=(0.0555)*Zbase  Inductance=(0.183)*Zbase/Wbase  Capacitance=1e-6  Measurements=None
  Branch41-41 : powerlib/Elements/Three-Phase Parallel RLC Branch  LConnTagsString=A|B|C  RConnTagsString=A|B|C  BranchType=RLC  Resistance=(2.5264)*Zbase  Inductance=(9.3476)*Zbase/Wbase  Capacitance=(0.02331)*Ybase/Wbase  Measurements=None
      settings: SourceProductBaseCode=PS
  Branch41-42 : powerlib/Elements/Three-Phase Series RLC Branch  LConnTagsString=A|B|C  RConnTagsString=A|B|C  BranchType=RL  Resistance=(0.041)*Zbase  Inductance=(0.135)*Zbase/Wbase  Capacitance=1e-6  Measurements=None
  Branch42-42 : powerlib/Elements/Three-Phase Parallel RLC Branch  LConnTagsString=A|B|C  RConnTagsString=A|B|C  BranchType=RLC  Resistance=(2.6222)*Zbase  Inductance=(4.2184)*Zbase/Wbase  Capacitance=(0.1265)*Ybase/Wbase  Measurements=None
      settings: SourceProductBaseCode=PS
  Branch42-49 : powerlib/Elements/Three-Phase Series RLC Branch  LConnTagsString=A|B|C  RConnTagsString=A|B|C  BranchType=RL  Resistance=(0.0715)*Zbase  Inductance=(0.323)*Zbase/Wbase  Capacitance=1e-6  Measurements=None
  Branch42-49_ : powerlib/Elements/Three-Phase Series RLC Branch  LConnTagsString=A|B|C  RConnTagsString=A|B|C  BranchType=RL  Resistance=(0.0715)*Zbase  Inductance=(0.323)*Zbase/Wbase  Capacitance=1e-6  Measurements=None
  Branch43-43 : powerlib/Elements/Three-Phase Parallel RLC Branch  LConnTagsString=A|B|C  RConnTagsString=A|B|C  BranchType=RLC  Resistance=(5.2386)*Zbase  Inductance=(13.4707)*Zbase/Wbase  Capacitance=(0.05147)*Ybase/Wbase  Measurements=None
      settings: SourceProductBaseCode=PS
  Branch43-44 : powerlib/Elements/Three-Phase Series RLC Branch  LConnTagsString=A|B|C  RConnTagsString=A|B|C  BranchType=RL  Resistance=(0.0608)*Zbase  Inductance=(0.2454)*Zbase/Wbase  Capacitance=1e-6  Measurements=None
  Branch44-44 : powerlib/Elements/Three-Phase Parallel RLC Branch  LConnTagsString=A|B|C  RConnTagsString=A|B|C  BranchType=RLC  Resistance=(5.8446)*Zbase  Inductance=(11.6892)*Zbase/Wbase  Capacitance=(0.04154)*Ybase/Wbase  Measurements=None
      settings: SourceProductBaseCode=PS
  Branch44-45 : powerlib/Elements/Three-Phase Series RLC Branch  LConnTagsString=A|B|C  RConnTagsString=A|B|C  BranchType=RL  Resistance=(0.0224)*Zbase  Inductance=(0.0901)*Zbase/Wbase  Capacitance=1e-6  Measurements=None
  Branch45-45 : powerlib/Elements/Three-Phase Parallel RLC Branch  LConnTagsString=A|B|C  RConnTagsString=A|B|C  BranchType=RLC  Resistance=(1.7899)*Zbase  Inductance=(4.3121)*Zbase/Wbase  Capacitance=(0.05)*Ybase/Wbase  Measurements=None
      settings: SourceProductBaseCode=PS
  Branch45-46 : powerlib/Elements/Three-Phase Series RLC Branch  LConnTagsString=A|B|C  RConnTagsString=A|B|C  BranchType=RL  Resistance=(0.04)*Zbase  Inductance=(0.1356)*Zbase/Wbase  Capacitance=1e-6  Measurements=None
  Branch45-49 : powerlib/Elements/Three-Phase Series RLC Branch  LConnTagsString=A|B|C  RConnTagsString=A|B|C  BranchType=RL  Resistance=(0.0684)*Zbase  Inductance=(0.186)*Zbase/Wbase  Capacitance=1e-6  Measurements=None
  Branch46-46 : powerlib/Elements/Three-Phase Parallel RLC Branch  LConnTagsString=A|B|C  RConnTagsString=A|B|C  BranchType=RLC  Resistance=(3.6072)*Zbase  Inductance=(10.1002)*Zbase/Wbase  Capacitance=(0.056)*Ybase/Wbase  Measurements=None
      settings: SourceProductBaseCode=PS
  Branch46-47 : powerlib/Elements/Three-Phase Series RLC Branch  LConnTagsString=A|B|C  RConnTagsString=A|B|C  BranchType=RL  Resistance=(0.038)*Zbase  Inductance=(0.127)*Zbase/Wbase  Capacitance=1e-6  Measurements=None
  Branch46-48 : powerlib/Elements/Three-Phase Series RLC Branch  LConnTagsString=A|B|C  RConnTagsString=A|B|C  BranchType=RL  Resistance=(0.0601)*Zbase  Inductance=(0.189)*Zbase/Wbase  Capacitance=1e-6  Measurements=None
  Branch47-47 : powerlib/Elements/Three-Phase Parallel RLC Branch  LConnTagsString=A|B|C  RConnTagsString=A|B|C  BranchType=RC  Resistance=(3.0419)*Zbase  Inductance=(Inf)*Zbase/Wbase  Capacitance=(0.05928)*Ybase/Wbase  Measurements=None
      settings: SourceProductBaseCode=PS
  Branch47-49 : powerlib/Elements/Three-Phase Series RLC Branch  LConnTagsString=A|B|C  RConnTagsString=A|B|C  BranchType=RL  Resistance=(0.0191)*Zbase  Inductance=(0.0625)*Zbase/Wbase  Capacitance=1e-6  Measurements=None
  Branch48-48 : powerlib/Elements/Three-Phase Parallel RLC Branch  LConnTagsString=A|B|C  RConnTagsString=A|B|C  BranchType=RLC  Resistance=(5.146)*Zbase  Inductance=(9.3565)*Zbase/Wbase  Capacitance=(0.02989)*Ybase/Wbase  Measurements=None
      settings: SourceProductBaseCode=PS
  Branch48-49 : powerlib/Elements/Three-Phase Series RLC Branch  LConnTagsString=A|B|C  RConnTagsString=A|B|C  BranchType=RL  Resistance=(0.0179)*Zbase  Inductance=(0.0505)*Zbase/Wbase  Capacitance=1e-6  Measurements=None
  Branch49-49 : powerlib/Elements/Three-Phase Parallel RLC Branch  LConnTagsString=A|B|C  RConnTagsString=A|B|C  BranchType=RLC  Resistance=(1.2076)*Zbase  Inductance=(3.5021)*Zbase/Wbase  Capacitance=(0.28858)*Ybase/Wbase  Measurements=None
      settings: SourceProductBaseCode=PS
  Branch49-50 : powerlib/Elements/Three-Phase Series RLC Branch  LConnTagsString=A|B|C  RConnTagsString=A|B|C  BranchType=RL  Resistance=(0.0267)*Zbase  Inductance=(0.0752)*Zbase/Wbase  Capacitance=1e-6  Measurements=None
  Branch49-51 : powerlib/Elements/Three-Phase Series RLC Branch  LConnTagsString=A|B|C  RConnTagsString=A|B|C  BranchType=RL  Resistance=(0.0486)*Zbase  Inductance=(0.137)*Zbase/Wbase  Capacitance=1e-6  Measurements=None
  Branch49-54 : powerlib/Elements/Three-Phase Series RLC Branch  LConnTagsString=A|B|C  RConnTagsString=A|B|C  BranchType=RL  Resistance=(0.073)*Zbase  Inductance=(0.289)*Zbase/Wbase  Capacitance=1e-6  Measurements=None
  Branch49-54_ : powerlib/Elements/Three-Phase Series RLC Branch  LConnTagsString=A|B|C  RConnTagsString=A|B|C  BranchType=RL  Resistance=(0.0869)*Zbase  Inductance=(0.291)*Zbase/Wbase  Capacitance=1e-6  Measurements=None
  Branch49-66 : powerlib/Elements/Three-Phase Series RLC Branch  LConnTagsString=A|B|C  RConnTagsString=A|B|C  BranchType=RL  Resistance=(0.018)*Zbase  Inductance=(0.0919)*Zbase/Wbase  Capacitance=1e-6  Measurements=None
  Branch49-66_ : powerlib/Elements/Three-Phase Series RLC Branch  LConnTagsString=A|B|C  RConnTagsString=A|B|C  BranchType=RL  Resistance=(0.018)*Zbase  Inductance=(0.0919)*Zbase/Wbase  Capacitance=1e-6  Measurements=None
  Branch5-11 : powerlib/Elements/Three-Phase Series RLC Branch  LConnTagsString=A|B|C  RConnTagsString=A|B|C  BranchType=RL  Resistance=(0.0203)*Zbase  Inductance=(0.0682)*Zbase/Wbase  Capacitance=1e-6  Measurements=None
  Branch5-5 : powerlib/Elements/Three-Phase Parallel RLC Branch  LConnTagsString=A|B|C  RConnTagsString=A|B|C  BranchType=C  Resistance=(Inf)*Zbase  Inductance=(Inf)*Zbase/Wbase  Capacitance=(0.03107)*Ybase/Wbase  Measurements=None
      settings: SourceProductBaseCode=PS
  Branch5-6 : powerlib/Elements/Three-Phase Series RLC Branch  LConnTagsString=A|B|C  RConnTagsString=A|B|C  BranchType=RL  Resistance=(0.0119)*Zbase  Inductance=(0.054)*Zbase/Wbase  Capacitance=1e-6  Measurements=None
  Branch5-8 : powerlib/Elements/Three-Phase Series RLC Branch  LConnTagsString=A|B|C  RConnTagsString=A|B|C  BranchType=RL  Resistance=(0.0025905)*Zbase  Inductance=(0.025905)*Zbase/Wbase  Capacitance=1e-6  Measurements=None
  Branch50-50 : powerlib/Elements/Three-Phase Parallel RLC Branch  LConnTagsString=A|B|C  RConnTagsString=A|B|C  BranchType=RLC  Resistance=(5.895)*Zbase  Inductance=(25.0538)*Zbase/Wbase  Capacitance=(0.02597)*Ybase/Wbase  Measurements=None
      settings: SourceProductBaseCode=PS
  Branch50-57 : powerlib/Elements/Three-Phase Series RLC Branch  LConnTagsString=A|B|C  RConnTagsString=A|B|C  BranchType=RL  Resistance=(0.0474)*Zbase  Inductance=(0.134)*Zbase/Wbase  Capacitance=1e-6  Measurements=None
  Branch51-51 : powerlib/Elements/Three-Phase Parallel RLC Branch  LConnTagsString=A|B|C  RConnTagsString=A|B|C  BranchType=RLC  Resistance=(5.499)*Zbase  Inductance=(11.6853)*Zbase/Wbase  Capacitance=(0.03302)*Ybase/Wbase  Measurements=None
      settings: SourceProductBaseCode=PS
  Branch51-52 : powerlib/Elements/Three-Phase Series RLC Branch  LConnTagsString=A|B|C  RConnTagsString=A|B|C  BranchType=RL  Resistance=(0.0203)*Zbase  Inductance=(0.0588)*Zbase/Wbase  Capacitance=1e-6  Measurements=None
  Branch51-58 : powerlib/Elements/Three-Phase Series RLC Branch  LConnTagsString=A|B|C  RConnTagsString=A|B|C  BranchType=RL  Resistance=(0.0255)*Zbase  Inductance=(0.0719)*Zbase/Wbase  Capacitance=1e-6  Measurements=None
  Branch52-52 : powerlib/Elements/Three-Phase Parallel RLC Branch  LConnTagsString=A|B|C  RConnTagsString=A|B|C  BranchType=RLC  Resistance=(5.086)*Zbase  Inductance=(18.3094)*Zbase/Wbase  Capacitance=(0.02727)*Ybase/Wbase  Measurements=None
      settings: SourceProductBaseCode=PS
  Branch52-53 : powerlib/Elements/Three-Phase Series RLC Branch  LConnTagsString=A|B|C  RConnTagsString=A|B|C  BranchType=RL  Resistance=(0.0405)*Zbase  Inductance=(0.1635)*Zbase/Wbase  Capacitance=1e-6  Measurements=None
  Branch53-53 : powerlib/Elements/Three-Phase Parallel RLC Branch  LConnTagsString=A|B|C  RConnTagsString=A|B|C  BranchType=RLC  Resistance=(3.8907)*Zbase  Inductance=(8.1352)*Zbase/Wbase  Capacitance=(0.03579)*Ybase/Wbase  Measurements=None
      settings: SourceProductBaseCode=PS
  Branch53-54 : powerlib/Elements/Three-Phase Series RLC Branch  LConnTagsString=A|B|C  RConnTagsString=A|B|C  BranchType=RL  Resistance=(0.0263)*Zbase  Inductance=(0.122)*Zbase/Wbase  Capacitance=1e-6  Measurements=None
  Branch54-54 : powerlib/Elements/Three-Phase Parallel RLC Branch  LConnTagsString=A|B|C  RConnTagsString=A|B|C  BranchType=RLC  Resistance=(0.8071)*Zbase  Inductance=(2.8501)*Zbase/Wbase  Capacitance=(0.13256)*Ybase/Wbase  Measurements=None
      settings: SourceProductBaseCode=PS
  Branch54-55 : powerlib/Elements/Three-Phase Series RLC Branch  LConnTagsString=A|B|C  RConnTagsString=A|B|C  BranchType=RL  Resistance=(0.0169)*Zbase  Inductance=(0.0707)*Zbase/Wbase  Capacitance=1e-6  Measurements=None
  Branch54-56 : powerlib/Elements/Three-Phase Series RLC Branch  LConnTagsString=A|B|C  RConnTagsString=A|B|C  BranchType=RL  Resistance=(0.00275)*Zbase  Inductance=(0.00955)*Zbase/Wbase  Capacitance=1e-6  Measurements=None
  Branch54-59 : powerlib/Elements/Three-Phase Series RLC Branch  LConnTagsString=A|B|C  RConnTagsString=A|B|C  BranchType=RL  Resistance=(0.0503)*Zbase  Inductance=(0.2293)*Zbase/Wbase  Capacitance=1e-6  Measurements=None
  Branch55-55 : powerlib/Elements/Three-Phase Parallel RLC Branch  LConnTagsString=A|B|C  RConnTagsString=A|B|C  BranchType=RLC  Resistance=(1.4386)*Zbase  Inductance=(4.1196)*Zbase/Wbase  Capacitance=(0.0402)*Ybase/Wbase  Measurements=None
      settings: SourceProductBaseCode=PS
  Branch55-56 : powerlib/Elements/Three-Phase Series RLC Branch  LConnTagsString=A|B|C  RConnTagsString=A|B|C  BranchType=RL  Resistance=(0.00488)*Zbase  Inductance=(0.0151)*Zbase/Wbase  Capacitance=1e-6  Measurements=None
  Branch55-59 : powerlib/Elements/Three-Phase Series RLC Branch  LConnTagsString=A|B|C  RConnTagsString=A|B|C  BranchType=RL  Resistance=(0.04739)*Zbase  Inductance=(0.2158)*Zbase/Wbase  Capacitance=1e-6  Measurements=None
  Branch56-56 : powerlib/Elements/Three-Phase Parallel RLC Branch  LConnTagsString=A|B|C  RConnTagsString=A|B|C  BranchType=RLC  Resistance=(1.0835)*Zbase  Inductance=(5.0562)*Zbase/Wbase  Capacitance=(0.08498)*Ybase/Wbase  Measurements=None
      settings: SourceProductBaseCode=PS
  Branch56-57 : powerlib/Elements/Three-Phase Series RLC Branch  LConnTagsString=A|B|C  RConnTagsString=A|B|C  BranchType=RL  Resistance=(0.0343)*Zbase  Inductance=(0.0966)*Zbase/Wbase  Capacitance=1e-6  Measurements=None
  Branch56-58 : powerlib/Elements/Three-Phase Series RLC Branch  LConnTagsString=A|B|C  RConnTagsString=A|B|C  BranchType=RL  Resistance=(0.0343)*Zbase  Inductance=(0.0966)*Zbase/Wbase  Capacitance=1e-6  Measurements=None
  Branch56-59 : powerlib/Elements/Three-Phase Series RLC Branch  LConnTagsString=A|B|C  RConnTagsString=A|B|C  BranchType=RL  Resistance=(0.0825)*Zbase  Inductance=(0.251)*Zbase/Wbase  Capacitance=1e-6  Measurements=None
  Branch56-59_ : powerlib/Elements/Three-Phase Series RLC Branch  LConnTagsString=A|B|C  RConnTagsString=A|B|C  BranchType=RL  Resistance=(0.0803)*Zbase  Inductance=(0.239)*Zbase/Wbase  Capacitance=1e-6  Measurements=None
  Branch57-57 : powerlib/Elements/Three-Phase Parallel RLC Branch  LConnTagsString=A|B|C  RConnTagsString=A|B|C  BranchType=RLC  Resistance=(7.8501)*Zbase  Inductance=(31.4005)*Zbase/Wbase  Capacitance=(0.0287)*Ybase/Wbase  Measurements=None
      settings: SourceProductBaseCode=PS
  Branch58-58 : powerlib/Elements/Three-Phase Parallel RLC Branch  LConnTagsString=A|B|C  RConnTagsString=A|B|C  BranchType=RLC  Resistance=(7.6645)*Zbase  Inductance=(30.6579)*Zbase/Wbase  Capacitance=(0.02104)*Ybase/Wbase  Measurements=None
      settings: SourceProductBaseCode=PS
  Branch59-59 : powerlib/Elements/Three-Phase Parallel RLC Branch  LConnTagsString=A|B|C  RConnTagsString=A|B|C  BranchType=RLC  Resistance=(0.35026)*Zbase  Inductance=(0.85861)*Zbase/Wbase  Capacitance=(0.15158)*Ybase/Wbase  Measurements=None
      settings: SourceProductBaseCode=PS
  Branch59-60 : powerlib/Elements/Three-Phase Series RLC Branch  LConnTagsString=A|B|C  RConnTagsString=A|B|C  BranchType=RL  Resistance=(0.0317)*Zbase  Inductance=(0.145)*Zbase/Wbase  Capacitance=1e-6  Measurements=None
  Branch59-61 : powerlib/Elements/Three-Phase Series RLC Branch  LConnTagsString=A|B|C  RConnTagsString=A|B|C  BranchType=RL  Resistance=(0.0328)*Zbase  Inductance=(0.15)*Zbase/Wbase  Capacitance=1e-6  Measurements=None
  Branch59-63 : powerlib/Elements/Three-Phase Series RLC Branch  LConnTagsString=A|B|C  RConnTagsString=A|B|C  BranchType=RL  Resistance=(0.0035574)*Zbase  Inductance=(0.035574)*Zbase/Wbase  Capacitance=1e-6  Measurements=None
  Branch6-6 : powerlib/Elements/Three-Phase Parallel RLC Branch  LConnTagsString=A|B|C  RConnTagsString=A|B|C  BranchType=RLC  Resistance=(1.8848)*Zbase  Inductance=(4.455)*Zbase/Wbase  Capacitance=(0.00988)*Ybase/Wbase  Measurements=None
      settings: SourceProductBaseCode=PS
  Branch6-7 : powerlib/Elements/Three-Phase Series RLC Branch  LConnTagsString=A|B|C  RConnTagsString=A|B|C  BranchType=RL  Resistance=(0.00459)*Zbase  Inductance=(0.0208)*Zbase/Wbase  Capacitance=1e-6  Measurements=None
  Branch60-60 : powerlib/Elements/Three-Phase Parallel RLC Branch  LConnTagsString=A|B|C  RConnTagsString=A|B|C  BranchType=RLC  Resistance=(1.2646)*Zbase  Inductance=(32.8788)*Zbase/Wbase  Capacitance=(0.03342)*Ybase/Wbase  Measurements=None
      settings: SourceProductBaseCode=PS
  Branch60-61 : powerlib/Elements/Three-Phase Series RLC Branch  LConnTagsString=A|B|C  RConnTagsString=A|B|C  BranchType=RL  Resistance=(0.00264)*Zbase  Inductance=(0.0135)*Zbase/Wbase  Capacitance=1e-6  Measurements=None
  Branch60-62 : powerlib/Elements/Three-Phase Series RLC Branch  LConnTagsString=A|B|C  RConnTagsString=A|B|C  BranchType=RL  Resistance=(0.0123)*Zbase  Inductance=(0.0561)*Zbase/Wbase  Capacitance=1e-6  Measurements=None
  Branch61-61 : powerlib/Elements/Three-Phase Parallel RLC Branch  LConnTagsString=A|B|C  RConnTagsString=A|B|C  BranchType=C  Resistance=(Inf)*Zbase  Inductance=(Inf)*Zbase/Wbase  Capacitance=(0.03158)*Ybase/Wbase  Measurements=None
      settings: SourceProductBaseCode=PS
  Branch61-62 : powerlib/Elements/Three-Phase Series RLC Branch  LConnTagsString=A|B|C  RConnTagsString=A|B|C  BranchType=RL  Resistance=(0.00824)*Zbase  Inductance=(0.0376)*Zbase/Wbase  Capacitance=1e-6  Measurements=None
  Branch61-64 : powerlib/Elements/Three-Phase Series RLC Branch  LConnTagsString=A|B|C  RConnTagsString=A|B|C  BranchType=RL  Resistance=(0.0026002)*Zbase  Inductance=(0.026002)*Zbase/Wbase  Capacitance=1e-6  Measurements=None
  Branch62-62 : powerlib/Elements/Three-Phase Parallel RLC Branch  LConnTagsString=A|B|C  RConnTagsString=A|B|C  BranchType=RLC  Resistance=(1.2935)*Zbase  Inductance=(7.1143)*Zbase/Wbase  Capacitance=(0.05664)*Ybase/Wbase  Measurements=None
      settings: SourceProductBaseCode=PS
  Branch62-66 : powerlib/Elements/Three-Phase Series RLC Branch  LConnTagsString=A|B|C  RConnTagsString=A|B|C  BranchType=RL  Resistance=(0.0482)*Zbase  Inductance=(0.218)*Zbase/Wbase  Capacitance=1e-6  Measurements=None
  Branch62-67 : powerlib/Elements/Three-Phase Series RLC Branch  LConnTagsString=A|B|C  RConnTagsString=A|B|C  BranchType=RL  Resistance=(0.0258)*Zbase  Inductance=(0.117)*Zbase/Wbase  Capacitance=1e-6  Measurements=None
  Branch63-63 : powerlib/Elements/Three-Phase Parallel RLC Branch  LConnTagsString=A|B|C  RConnTagsString=A|B|C  BranchType=C  Resistance=(Inf)*Zbase  Inductance=(Inf)*Zbase/Wbase  Capacitance=(0.108)*Ybase/Wbase  Measurements=None
      settings: SourceProductBaseCode=PS
  Branch63-64 : powerlib/Elements/Three-Phase Series RLC Branch  LConnTagsString=A|B|C  RConnTagsString=A|B|C  BranchType=RL  Resistance=(0.00172)*Zbase  Inductance=(0.02)*Zbase/Wbase  Capacitance=1e-6  Measurements=None
  Branch64-64 : powerlib/Elements/Three-Phase Parallel RLC Branch  LConnTagsString=A|B|C  RConnTagsString=A|B|C  BranchType=C  Resistance=(Inf)*Zbase  Inductance=(Inf)*Zbase/Wbase  Capacitance=(0.298)*Ybase/Wbase  Measurements=None
      settings: SourceProductBaseCode=PS
  Branch64-65 : powerlib/Elements/Three-Phase Series RLC Branch  LConnTagsString=A|B|C  RConnTagsString=A|B|C  BranchType=RL  Resistance=(0.00269)*Zbase  Inductance=(0.0302)*Zbase/Wbase  Capacitance=1e-6  Measurements=None
  Branch65-65 : powerlib/Elements/Three-Phase Parallel RLC Branch  LConnTagsString=A|B|C  RConnTagsString=A|B|C  BranchType=C  Resistance=(Inf)*Zbase  Inductance=(Inf)*Zbase/Wbase  Capacitance=(1.032)*Ybase/Wbase  Measurements=None
      settings: SourceProductBaseCode=PS
  Branch65-66 : powerlib/Elements/Three-Phase Series RLC Branch  LConnTagsString=A|B|C  RConnTagsString=A|B|C  BranchType=RL  Resistance=(0.0037)*Zbase  Inductance=(0.037)*Zbase/Wbase  Capacitance=1e-6  Measurements=None
  Branch65-68 : powerlib/Elements/Three-Phase Series RLC Branch  LConnTagsString=A|B|C  RConnTagsString=A|B|C  BranchType=RL  Resistance=(0.00138)*Zbase  Inductance=(0.016)*Zbase/Wbase  Capacitance=1e-6  Measurements=None
  Branch66-66 : powerlib/Elements/Three-Phase Parallel RLC Branch  LConnTagsString=A|B|C  RConnTagsString=A|B|C  BranchType=RLC  Resistance=(2.8269)*Zbase  Inductance=(6.125)*Zbase/Wbase  Capacitance=(0.06711)*Ybase/Wbase  Measurements=None
      settings: SourceProductBaseCode=PS
  Branch66-67 : powerlib/Elements/Three-Phase Series RLC Branch  LConnTagsString=A|B|C  RConnTagsString=A|B|C  BranchType=RL  Resistance=(0.0224)*Zbase  Inductance=(0.1015)*Zbase/Wbase  Capacitance=1e-6  Measurements=None
  Branch67-67 : powerlib/Elements/Three-Phase Parallel RLC Branch  LConnTagsString=A|B|C  RConnTagsString=A|B|C  BranchType=RLC  Resistance=(3.7133)*Zbase  Inductance=(14.8531)*Zbase/Wbase  Capacitance=(0.02891)*Ybase/Wbase  Measurements=None
      settings: SourceProductBaseCode=PS
  Branch68-116 : powerlib/Elements/Three-Phase Series RLC Branch  LConnTagsString=A|B|C  RConnTagsString=A|B|C  BranchType=RL  Resistance=(0.00034)*Zbase  Inductance=(0.00405)*Zbase/Wbase  Capacitance=1e-6  Measurements=None
  Branch68-68 : powerlib/Elements/Three-Phase Parallel RLC Branch  LConnTagsString=A|B|C  RConnTagsString=A|B|C  BranchType=C  Resistance=(Inf)*Zbase  Inductance=(Inf)*Zbase/Wbase  Capacitance=(0.805)*Ybase/Wbase  Measurements=None
      settings: SourceProductBaseCode=PS
  Branch68-81 : powerlib/Elements/Three-Phase Series RLC Branch  LConnTagsString=A|B|C  RConnTagsString=A|B|C  BranchType=RL  Resistance=(0.00175)*Zbase  Inductance=(0.0202)*Zbase/Wbase  Capacitance=1e-6  Measurements=None
  Branch69-69 : powerlib/Elements/Three-Phase Parallel RLC Branch  LConnTagsString=A|B|C  RConnTagsString=A|B|C  BranchType=RLC  Resistance=(1.7883)*Zbase  Inductance=(3.3779)*Zbase/Wbase  Capacitance=(0.01811)*Ybase/Wbase  Measurements=None
      settings: SourceProductBaseCode=PS
  Branch7-12 : powerlib/Elements/Three-Phase Series RLC Branch  LConnTagsString=A|B|C  RConnTagsString=A|B|C  BranchType=RL  Resistance=(0.00862)*Zbase  Inductance=(0.034)*Zbase/Wbase  Capacitance=1e-6  Measurements=None
  Branch7-7 : powerlib/Elements/Three-Phase Parallel RLC Branch  LConnTagsString=A|B|C  RConnTagsString=A|B|C  BranchType=RLC  Resistance=(5.1514)*Zbase  Inductance=(48.9384)*Zbase/Wbase  Capacitance=(0.00712)*Ybase/Wbase  Measurements=None
      settings: SourceProductBaseCode=PS
  Branch70-70 : powerlib/Elements/Three-Phase Parallel RLC Branch  LConnTagsString=A|B|C  RConnTagsString=A|B|C  BranchType=RLC  Resistance=(1.4671)*Zbase  Inductance=(4.8413)*Zbase/Wbase  Capacitance=(0.15122)*Ybase/Wbase  Measurements=None
      settings: SourceProductBaseCode=PS
  Branch70-71 : powerlib/Elements/Three-Phase Series RLC Branch  LConnTagsString=A|B|C  RConnTagsString=A|B|C  BranchType=RL  Resistance=(0.00882)*Zbase  Inductance=(0.0355)*Zbase/Wbase  Capacitance=1e-6  Measurements=None
  Branch70-74 : powerlib/Elements/Three-Phase Series RLC Branch  LConnTagsString=A|B|C  RConnTagsString=A|B|C  BranchType=RL  Resistance=(0.0401)*Zbase  Inductance=(0.1323)*Zbase/Wbase  Capacitance=1e-6  Measurements=None
  Branch70-75 : powerlib/Elements/Three-Phase Series RLC Branch  LConnTagsString=A|B|C  RConnTagsString=A|B|C  BranchType=RL  Resistance=(0.0428)*Zbase  Inductance=(0.141)*Zbase/Wbase  Capacitance=1e-6  Measurements=None
  Branch71-71 : powerlib/Elements/Three-Phase Parallel RLC Branch  LConnTagsString=A|B|C  RConnTagsString=A|B|C  BranchType=C  Resistance=(Inf)*Zbase  Inductance=(Inf)*Zbase/Wbase  Capacitance=(0.0325)*Ybase/Wbase  Measurements=None
      settings: SourceProductBaseCode=PS
  Branch71-72 : powerlib/Elements/Three-Phase Series RLC Branch  LConnTagsString=A|B|C  RConnTagsString=A|B|C  BranchType=RL  Resistance=(0.0446)*Zbase  Inductance=(0.18)*Zbase/Wbase  Capacitance=1e-6  Measurements=None
  Branch71-73 : powerlib/Elements/Three-Phase Series RLC Branch  LConnTagsString=A|B|C  RConnTagsString=A|B|C  BranchType=RL  Resistance=(0.00866)*Zbase  Inductance=(0.0454)*Zbase/Wbase  Capacitance=1e-6  Measurements=None
  Branch72-72 : powerlib/Elements/Three-Phase Parallel RLC Branch  LConnTagsString=A|B|C  RConnTagsString=A|B|C  BranchType=C  Resistance=(Inf)*Zbase  Inductance=(Inf)*Zbase/Wbase  Capacitance=(0.04662)*Ybase/Wbase  Measurements=None
      settings: SourceProductBaseCode=PS
  Branch73-73 : powerlib/Elements/Three-Phase Parallel RLC Branch  LConnTagsString=A|B|C  RConnTagsString=A|B|C  BranchType=C  Resistance=(Inf)*Zbase  Inductance=(Inf)*Zbase/Wbase  Capacitance=(0.00589)*Ybase/Wbase  Measurements=None
      settings: SourceProductBaseCode=PS
  Branch74-74 : powerlib/Elements/Three-Phase Parallel RLC Branch  LConnTagsString=A|B|C  RConnTagsString=A|B|C  BranchType=RLC  Resistance=(1.3497)*Zbase  Inductance=(3.3991)*Zbase/Wbase  Capacitance=(0.02201)*Ybase/Wbase  Measurements=None
      settings: SourceProductBaseCode=PS
  Branch74-75 : powerlib/Elements/Three-Phase Series RLC Branch  LConnTagsString=A|B|C  RConnTagsString=A|B|C  BranchType=RL  Resistance=(0.0123)*Zbase  Inductance=(0.0406)*Zbase/Wbase  Capacitance=1e-6  Measurements=None
  Branch75-118 : powerlib/Elements/Three-Phase Series RLC Branch  LConnTagsString=A|B|C  RConnTagsString=A|B|C  BranchType=RL  Resistance=(0.0145)*Zbase  Inductance=(0.0481)*Zbase/Wbase  Capacitance=1e-6  Measurements=None
  Branch75-75 : powerlib/Elements/Three-Phase Parallel RLC Branch  LConnTagsString=A|B|C  RConnTagsString=A|B|C  BranchType=RLC  Resistance=(1.9908)*Zbase  Inductance=(8.5061)*Zbase/Wbase  Capacitance=(0.11605)*Ybase/Wbase  Measurements=None
      settings: SourceProductBaseCode=PS
  Branch75-77 : powerlib/Elements/Three-Phase Series RLC Branch  LConnTagsString=A|B|C  RConnTagsString=A|B|C  BranchType=RL  Resistance=(0.0601)*Zbase  Inductance=(0.1999)*Zbase/Wbase  Capacitance=1e-6  Measurements=None
  Branch76-118 : powerlib/Elements/Three-Phase Series RLC Branch  LConnTagsString=A|B|C  RConnTagsString=A|B|C  BranchType=RL  Resistance=(0.0164)*Zbase  Inductance=(0.0544)*Zbase/Wbase  Capacitance=1e-6  Measurements=None
  Branch76-76 : powerlib/Elements/Three-Phase Parallel RLC Branch  LConnTagsString=A|B|C  RConnTagsString=A|B|C  BranchType=RLC  Resistance=(1.3077)*Zbase  Inductance=(2.4701)*Zbase/Wbase  Capacitance=(0.02518)*Ybase/Wbase  Measurements=None
      settings: SourceProductBaseCode=PS
  Branch76-77 : powerlib/Elements/Three-Phase Series RLC Branch  LConnTagsString=A|B|C  RConnTagsString=A|B|C  BranchType=RL  Resistance=(0.0444)*Zbase  Inductance=(0.148)*Zbase/Wbase  Capacitance=1e-6  Measurements=None
  Branch77-77 : powerlib/Elements/Three-Phase Parallel RLC Branch  LConnTagsString=A|B|C  RConnTagsString=A|B|C  BranchType=RLC  Resistance=(1.6591)*Zbase  Inductance=(3.6144)*Zbase/Wbase  Capacitance=(0.17738)*Ybase/Wbase  Measurements=None
      settings: SourceProductBaseCode=PS
  Branch77-78 : powerlib/Elements/Three-Phase Series RLC Branch  LConnTagsString=A|B|C  RConnTagsString=A|B|C  BranchType=RL  Resistance=(0.00376)*Zbase  Inductance=(0.0124)*Zbase/Wbase  Capacitance=1e-6  Measurements=None
  Branch77-80 : powerlib/Elements/Three-Phase Series RLC Branch  LConnTagsString=A|B|C  RConnTagsString=A|B|C  BranchType=RL  Resistance=(0.017)*Zbase  Inductance=(0.0485)*Zbase/Wbase  Capacitance=1e-6  Measurements=None
  Branch77-80_ : powerlib/Elements/Three-Phase Series RLC Branch  LConnTagsString=A|B|C  RConnTagsString=A|B|C  BranchType=RL  Resistance=(0.0294)*Zbase  Inductance=(0.105)*Zbase/Wbase  Capacitance=1e-6  Measurements=None
  Branch77-82 : powerlib/Elements/Three-Phase Series RLC Branch  LConnTagsString=A|B|C  RConnTagsString=A|B|C  BranchType=RL  Resistance=(0.0298)*Zbase  Inductance=(0.0853)*Zbase/Wbase  Capacitance=1e-6  Measurements=None
  Branch78-78 : powerlib/Elements/Three-Phase Parallel RLC Branch  LConnTagsString=A|B|C  RConnTagsString=A|B|C  BranchType=RLC  Resistance=(1.4134)*Zbase  Inductance=(3.8597)*Zbase/Wbase  Capacitance=(0.00956)*Ybase/Wbase  Measurements=None
      settings: SourceProductBaseCode=PS
  Branch78-79 : powerlib/Elements/Three-Phase Series RLC Branch  LConnTagsString=A|B|C  RConnTagsString=A|B|C  BranchType=RL  Resistance=(0.00546)*Zbase  Inductance=(0.0244)*Zbase/Wbase  Capacitance=1e-6  Measurements=None
  Branch79-79 : powerlib/Elements/Three-Phase Parallel RLC Branch  LConnTagsString=A|B|C  RConnTagsString=A|B|C  BranchType=RLC  Resistance=(2.5862)*Zbase  Inductance=(3.1519)*Zbase/Wbase  Capacitance=(0.01259)*Ybase/Wbase  Measurements=None
      settings: SourceProductBaseCode=PS
  Branch79-80 : powerlib/Elements/Three-Phase Series RLC Branch  LConnTagsString=A|B|C  RConnTagsString=A|B|C  BranchType=RL  Resistance=(0.0156)*Zbase  Inductance=(0.0704)*Zbase/Wbase  Capacitance=1e-6  Measurements=None
  Branch8-30 : powerlib/Elements/Three-Phase Series RLC Branch  LConnTagsString=A|B|C  RConnTagsString=A|B|C  BranchType=RL  Resistance=(0.00431)*Zbase  Inductance=(0.0504)*Zbase/Wbase  Capacitance=1e-6  Measurements=None
  Branch8-8 : powerlib/Elements/Three-Phase Parallel RLC Branch  LConnTagsString=A|B|C  RConnTagsString=A|B|C  BranchType=C  Resistance=(Inf)*Zbase  Inductance=(Inf)*Zbase/Wbase  Capacitance=(0.838)*Ybase/Wbase  Measurements=None
      settings: SourceProductBaseCode=PS
  Branch8-9 : powerlib/Elements/Three-Phase Series RLC Branch  LConnTagsString=A|B|C  RConnTagsString=A|B|C  BranchType=RL  Resistance=(0.00244)*Zbase  Inductance=(0.0305)*Zbase/Wbase  Capacitance=1e-6  Measurements=None
  Branch80-80 : powerlib/Elements/Three-Phase Parallel RLC Branch  LConnTagsString=A|B|C  RConnTagsString=A|B|C  BranchType=RLC  Resistance=(0.832)*Zbase  Inductance=(4.16)*Zbase/Wbase  Capacitance=(0.12335)*Ybase/Wbase  Measurements=None
      settings: SourceProductBaseCode=PS
  Branch80-81 : powerlib/Elements/Three-Phase Series RLC Branch  LConnTagsString=A|B|C  RConnTagsString=A|B|C  BranchType=RL  Resistance=(0.0032346)*Zbase  Inductance=(0.032346)*Zbase/Wbase  Capacitance=1e-6  Measurements=None
  Branch80-96 : powerlib/Elements/Three-Phase Series RLC Branch  LConnTagsString=A|B|C  RConnTagsString=A|B|C  BranchType=RL  Resistance=(0.0356)*Zbase  Inductance=(0.182)*Zbase/Wbase  Capacitance=1e-6  Measurements=None
  Branch80-97 : powerlib/Elements/Three-Phase Series RLC Branch  LConnTagsString=A|B|C  RConnTagsString=A|B|C  BranchType=RL  Resistance=(0.0183)*Zbase  Inductance=(0.0934)*Zbase/Wbase  Capacitance=1e-6  Measurements=None
  Branch80-98 : powerlib/Elements/Three-Phase Series RLC Branch  LConnTagsString=A|B|C  RConnTagsString=A|B|C  BranchType=RL  Resistance=(0.0238)*Zbase  Inductance=(0.108)*Zbase/Wbase  Capacitance=1e-6  Measurements=None
  Branch80-99 : powerlib/Elements/Three-Phase Series RLC Branch  LConnTagsString=A|B|C  RConnTagsString=A|B|C  BranchType=RL  Resistance=(0.0454)*Zbase  Inductance=(0.206)*Zbase/Wbase  Capacitance=1e-6  Measurements=None
  Branch81-81 : powerlib/Elements/Three-Phase Parallel RLC Branch  LConnTagsString=A|B|C  RConnTagsString=A|B|C  BranchType=C  Resistance=(Inf)*Zbase  Inductance=(Inf)*Zbase/Wbase  Capacitance=(0.404)*Ybase/Wbase  Measurements=None
      settings: SourceProductBaseCode=PS
  Branch82-82 : powerlib/Elements/Three-Phase Parallel RLC Branch  LConnTagsString=A|B|C  RConnTagsString=A|B|C  BranchType=RLC  Resistance=(1.7779)*Zbase  Inductance=(3.5558)*Zbase/Wbase  Capacitance=(0.08705)*Ybase/Wbase  Measurements=None
      settings: SourceProductBaseCode=PS
  Branch82-83 : powerlib/Elements/Three-Phase Series RLC Branch  LConnTagsString=A|B|C  RConnTagsString=A|B|C  BranchType=RL  Resistance=(0.0112)*Zbase  Inductance=(0.03665)*Zbase/Wbase  Capacitance=1e-6  Measurements=None
  Branch82-96 : powerlib/Elements/Three-Phase Series RLC Branch  LConnTagsString=A|B|C  RConnTagsString=A|B|C  BranchType=RL  Resistance=(0.0162)*Zbase  Inductance=(0.053)*Zbase/Wbase  Capacitance=1e-6  Measurements=None
  Branch83-83 : powerlib/Elements/Three-Phase Parallel RLC Branch  LConnTagsString=A|B|C  RConnTagsString=A|B|C  BranchType=RLC  Resistance=(4.7606)*Zbase  Inductance=(9.5212)*Zbase/Wbase  Capacitance=(0.04928)*Ybase/Wbase  Measurements=None
      settings: SourceProductBaseCode=PS
  Branch83-84 : powerlib/Elements/Three-Phase Series RLC Branch  LConnTagsString=A|B|C  RConnTagsString=A|B|C  BranchType=RL  Resistance=(0.0625)*Zbase  Inductance=(0.132)*Zbase/Wbase  Capacitance=1e-6  Measurements=None
  Branch83-85 : powerlib/Elements/Three-Phase Series RLC Branch  LConnTagsString=A|B|C  RConnTagsString=A|B|C  BranchType=RL  Resistance=(0.043)*Zbase  Inductance=(0.148)*Zbase/Wbase  Capacitance=1e-6  Measurements=None
  Branch84-84 : powerlib/Elements/Three-Phase Parallel RLC Branch  LConnTagsString=A|B|C  RConnTagsString=A|B|C  BranchType=RLC  Resistance=(8.6761)*Zbase  Inductance=(13.6338)*Zbase/Wbase  Capacitance=(0.01907)*Ybase/Wbase  Measurements=None
      settings: SourceProductBaseCode=PS
  Branch84-85 : powerlib/Elements/Three-Phase Series RLC Branch  LConnTagsString=A|B|C  RConnTagsString=A|B|C  BranchType=RL  Resistance=(0.0302)*Zbase  Inductance=(0.0641)*Zbase/Wbase  Capacitance=1e-6  Measurements=None
  Branch85-85 : powerlib/Elements/Three-Phase Parallel RLC Branch  LConnTagsString=A|B|C  RConnTagsString=A|B|C  BranchType=RLC  Resistance=(4.0426)*Zbase  Inductance=(6.4682)*Zbase/Wbase  Capacitance=(0.07467)*Ybase/Wbase  Measurements=None
      settings: SourceProductBaseCode=PS
  Branch85-86 : powerlib/Elements/Three-Phase Series RLC Branch  LConnTagsString=A|B|C  RConnTagsString=A|B|C  BranchType=RL  Resistance=(0.035)*Zbase  Inductance=(0.123)*Zbase/Wbase  Capacitance=1e-6  Measurements=None
  Branch85-88 : powerlib/Elements/Three-Phase Series RLC Branch  LConnTagsString=A|B|C  RConnTagsString=A|B|C  BranchType=RL  Resistance=(0.02)*Zbase  Inductance=(0.102)*Zbase/Wbase  Capacitance=1e-6  Measurements=None
  Branch85-89 : powerlib/Elements/Three-Phase Series RLC Branch  LConnTagsString=A|B|C  RConnTagsString=A|B|C  BranchType=RL  Resistance=(0.0239)*Zbase  Inductance=(0.173)*Zbase/Wbase  Capacitance=1e-6  Measurements=None
  Branch86-86 : powerlib/Elements/Three-Phase Parallel RLC Branch  LConnTagsString=A|B|C  RConnTagsString=A|B|C  BranchType=RLC  Resistance=(4.636)*Zbase  Inductance=(9.7356)*Zbase/Wbase  Capacitance=(0.03605)*Ybase/Wbase  Measurements=None
      settings: SourceProductBaseCode=PS
  Branch86-87 : powerlib/Elements/Three-Phase Series RLC Branch  LConnTagsString=A|B|C  RConnTagsString=A|B|C  BranchType=RL  Resistance=(0.02828)*Zbase  Inductance=(0.2074)*Zbase/Wbase  Capacitance=1e-6  Measurements=None
  Branch87-87 : powerlib/Elements/Three-Phase Parallel RLC Branch  LConnTagsString=A|B|C  RConnTagsString=A|B|C  BranchType=C  Resistance=(Inf)*Zbase  Inductance=(Inf)*Zbase/Wbase  Capacitance=(0.02225)*Ybase/Wbase  Measurements=None
      settings: SourceProductBaseCode=PS
  Branch88-88 : powerlib/Elements/Three-Phase Parallel RLC Branch  LConnTagsString=A|B|C  RConnTagsString=A|B|C  BranchType=RLC  Resistance=(2.0314)*Zbase  Inductance=(9.7508)*Zbase/Wbase  Capacitance=(0.02347)*Ybase/Wbase  Measurements=None
      settings: SourceProductBaseCode=PS
  Branch88-89 : powerlib/Elements/Three-Phase Series RLC Branch  LConnTagsString=A|B|C  RConnTagsString=A|B|C  BranchType=RL  Resistance=(0.0139)*Zbase  Inductance=(0.0712)*Zbase/Wbase  Capacitance=1e-6  Measurements=None
  Branch89-89 : powerlib/Elements/Three-Phase Parallel RLC Branch  LConnTagsString=A|B|C  RConnTagsString=A|B|C  BranchType=C  Resistance=(Inf)*Zbase  Inductance=(Inf)*Zbase/Wbase  Capacitance=(0.16067)*Ybase/Wbase  Measurements=None
      settings: SourceProductBaseCode=PS
  Branch89-90 : powerlib/Elements/Three-Phase Series RLC Branch  LConnTagsString=A|B|C  RConnTagsString=A|B|C  BranchType=RL  Resistance=(0.0518)*Zbase  Inductance=(0.188)*Zbase/Wbase  Capacitance=1e-6  Measurements=None
  Branch89-90_ : powerlib/Elements/Three-Phase Series RLC Branch  LConnTagsString=A|B|C  RConnTagsString=A|B|C  BranchType=RL  Resistance=(0.0238)*Zbase  Inductance=(0.0997)*Zbase/Wbase  Capacitance=1e-6  Measurements=None
  Branch89-92 : powerlib/Elements/Three-Phase Series RLC Branch  LConnTagsString=A|B|C  RConnTagsString=A|B|C  BranchType=RL  Resistance=(0.0099)*Zbase  Inductance=(0.0505)*Zbase/Wbase  Capacitance=1e-6  Measurements=None
  Branch89-92_ : powerlib/Elements/Three-Phase Series RLC Branch  LConnTagsString=A|B|C  RConnTagsString=A|B|C  BranchType=RL  Resistance=(0.0393)*Zbase  Inductance=(0.1581)*Zbase/Wbase  Capacitance=1e-6  Measurements=None
  Branch9-10 : powerlib/Elements/Three-Phase Series RLC Branch  LConnTagsString=A|B|C  RConnTagsString=A|B|C  BranchType=RL  Resistance=(0.00258)*Zbase  Inductance=(0.0322)*Zbase/Wbase  Capacitance=1e-6  Measurements=None
  Branch9-9 : powerlib/Elements/Three-Phase Parallel RLC Branch  LConnTagsString=A|B|C  RConnTagsString=A|B|C  BranchType=C  Resistance=(Inf)*Zbase  Inductance=(Inf)*Zbase/Wbase  Capacitance=(1.196)*Ybase/Wbase  Measurements=None
      settings: SourceProductBaseCode=PS
  Branch90-90 : powerlib/Elements/Three-Phase Parallel RLC Branch  LConnTagsString=A|B|C  RConnTagsString=A|B|C  BranchType=RLC  Resistance=(1.2439)*Zbase  Inductance=(2.3101)*Zbase/Wbase  Capacitance=(0.0901)*Ybase/Wbase  Measurements=None
      settings: SourceProductBaseCode=PS
  Branch90-91 : powerlib/Elements/Three-Phase Series RLC Branch  LConnTagsString=A|B|C  RConnTagsString=A|B|C  BranchType=RL  Resistance=(0.0254)*Zbase  Inductance=(0.0836)*Zbase/Wbase  Capacitance=1e-6  Measurements=None
  Branch91-91 : powerlib/Elements/Three-Phase Parallel RLC Branch  LConnTagsString=A|B|C  RConnTagsString=A|B|C  BranchType=C  Resistance=(Inf)*Zbase  Inductance=(Inf)*Zbase/Wbase  Capacitance=(0.02704)*Ybase/Wbase  Measurements=None
      settings: SourceProductBaseCode=PS
  Branch91-92 : powerlib/Elements/Three-Phase Series RLC Branch  LConnTagsString=A|B|C  RConnTagsString=A|B|C  BranchType=RL  Resistance=(0.0387)*Zbase  Inductance=(0.1272)*Zbase/Wbase  Capacitance=1e-6  Measurements=None
  Branch92-100 : powerlib/Elements/Three-Phase Series RLC Branch  LConnTagsString=A|B|C  RConnTagsString=A|B|C  BranchType=RL  Resistance=(0.0648)*Zbase  Inductance=(0.295)*Zbase/Wbase  Capacitance=1e-6  Measurements=None
  Branch92-102 : powerlib/Elements/Three-Phase Series RLC Branch  LConnTagsString=A|B|C  RConnTagsString=A|B|C  BranchType=RL  Resistance=(0.0123)*Zbase  Inductance=(0.0559)*Zbase/Wbase  Capacitance=1e-6  Measurements=None
  Branch92-92 : powerlib/Elements/Three-Phase Parallel RLC Branch  LConnTagsString=A|B|C  RConnTagsString=A|B|C  BranchType=RLC  Resistance=(1.517)*Zbase  Inductance=(9.8605)*Zbase/Wbase  Capacitance=(0.12656)*Ybase/Wbase  Measurements=None
      settings: SourceProductBaseCode=PS
  Branch92-93 : powerlib/Elements/Three-Phase Series RLC Branch  LConnTagsString=A|B|C  RConnTagsString=A|B|C  BranchType=RL  Resistance=(0.0258)*Zbase  Inductance=(0.0848)*Zbase/Wbase  Capacitance=1e-6  Measurements=None
  Branch92-94 : powerlib/Elements/Three-Phase Series RLC Branch  LConnTagsString=A|B|C  RConnTagsString=A|B|C  BranchType=RL  Resistance=(0.0481)*Zbase  Inductance=(0.158)*Zbase/Wbase  Capacitance=1e-6  Measurements=None
  Branch93-93 : powerlib/Elements/Three-Phase Parallel RLC Branch  LConnTagsString=A|B|C  RConnTagsString=A|B|C  BranchType=RLC  Resistance=(8.1091)*Zbase  Inductance=(13.9014)*Zbase/Wbase  Capacitance=(0.02028)*Ybase/Wbase  Measurements=None
      settings: SourceProductBaseCode=PS
  Branch93-94 : powerlib/Elements/Three-Phase Series RLC Branch  LConnTagsString=A|B|C  RConnTagsString=A|B|C  BranchType=RL  Resistance=(0.0223)*Zbase  Inductance=(0.0732)*Zbase/Wbase  Capacitance=1e-6  Measurements=None
  Branch94-100 : powerlib/Elements/Three-Phase Series RLC Branch  LConnTagsString=A|B|C  RConnTagsString=A|B|C  BranchType=RL  Resistance=(0.0178)*Zbase  Inductance=(0.058)*Zbase/Wbase  Capacitance=1e-6  Measurements=None
  Branch94-94 : powerlib/Elements/Three-Phase Parallel RLC Branch  LConnTagsString=A|B|C  RConnTagsString=A|B|C  BranchType=RLC  Resistance=(3.261)*Zbase  Inductance=(6.1144)*Zbase/Wbase  Capacitance=(0.07693)*Ybase/Wbase  Measurements=None
      settings: SourceProductBaseCode=PS
  Branch94-95 : powerlib/Elements/Three-Phase Series RLC Branch  LConnTagsString=A|B|C  RConnTagsString=A|B|C  BranchType=RL  Resistance=(0.0132)*Zbase  Inductance=(0.0434)*Zbase/Wbase  Capacitance=1e-6  Measurements=None
  Branch94-96 : powerlib/Elements/Three-Phase Series RLC Branch  LConnTagsString=A|B|C  RConnTagsString=A|B|C  BranchType=RL  Resistance=(0.0269)*Zbase  Inductance=(0.0869)*Zbase/Wbase  Capacitance=1e-6  Measurements=None
  Branch95-95 : powerlib/Elements/Three-Phase Parallel RLC Branch  LConnTagsString=A|B|C  RConnTagsString=A|B|C  BranchType=RLC  Resistance=(2.2789)*Zbase  Inductance=(3.0876)*Zbase/Wbase  Capacitance=(0.01292)*Ybase/Wbase  Measurements=None
      settings: SourceProductBaseCode=PS
  Branch95-96 : powerlib/Elements/Three-Phase Series RLC Branch  LConnTagsString=A|B|C  RConnTagsString=A|B|C  BranchType=RL  Resistance=(0.0171)*Zbase  Inductance=(0.0547)*Zbase/Wbase  Capacitance=1e-6  Measurements=None
  Branch96-96 : powerlib/Elements/Three-Phase Parallel RLC Branch  LConnTagsString=A|B|C  RConnTagsString=A|B|C  BranchType=RLC  Resistance=(2.5727)*Zbase  Inductance=(6.5175)*Zbase/Wbase  Capacitance=(0.08277)*Ybase/Wbase  Measurements=None
      settings: SourceProductBaseCode=PS
  Branch96-97 : powerlib/Elements/Three-Phase Series RLC Branch  LConnTagsString=A|B|C  RConnTagsString=A|B|C  BranchType=RL  Resistance=(0.0173)*Zbase  Inductance=(0.0885)*Zbase/Wbase  Capacitance=1e-6  Measurements=None
  Branch97-97 : powerlib/Elements/Three-Phase Parallel RLC Branch  LConnTagsString=A|B|C  RConnTagsString=A|B|C  BranchType=RLC  Resistance=(6.7919)*Zbase  Inductance=(11.3198)*Zbase/Wbase  Capacitance=(0.0247)*Ybase/Wbase  Measurements=None
      settings: SourceProductBaseCode=PS
  Branch98-100 : powerlib/Elements/Three-Phase Series RLC Branch  LConnTagsString=A|B|C  RConnTagsString=A|B|C  BranchType=RL  Resistance=(0.0397)*Zbase  Inductance=(0.179)*Zbase/Wbase  Capacitance=1e-6  Measurements=None
  Branch98-98 : powerlib/Elements/Three-Phase Parallel RLC Branch  LConnTagsString=A|B|C  RConnTagsString=A|B|C  BranchType=RLC  Resistance=(3.0811)*Zbase  Inductance=(13.0947)*Zbase/Wbase  Capacitance=(0.0381)*Ybase/Wbase  Measurements=None
      settings: SourceProductBaseCode=PS
  Branch99-100 : powerlib/Elements/Three-Phase Series RLC Branch  LConnTagsString=A|B|C  RConnTagsString=A|B|C  BranchType=RL  Resistance=(0.018)*Zbase  Inductance=(0.0813)*Zbase/Wbase  Capacitance=1e-6  Measurements=None
  Branch99-99 : powerlib/Elements/Three-Phase Parallel RLC Branch  LConnTagsString=A|B|C  RConnTagsString=A|B|C  BranchType=C  Resistance=(Inf)*Zbase  Inductance=(Inf)*Zbase/Wbase  Capacitance=(0.0381)*Ybase/Wbase  Measurements=None
      settings: SourceProductBaseCode=PS
  Bus{1..118} (118 alike) : SimplusGT/Three-Phase Bus  Vbase=1  Sbase=1
      settings: SourceProductName=Simplus Grid Tool
  D-GND{1,4,6,8,10,12,15,18..19,24..27,31..32,34,36,40,42,46,49,54..56,59,61..62,65..66,69..70,72..74,76..77,80,85,87,89..92,99..100,103..105,107,110..113,116} (54 alike) : powerlib/Elements/Ground  LConnTagsString=a
  D-Scope{1,4,6,8,10,12,15,18..19,24..27,31..32,34,36,40,42,46,49,54..56,59,61..62,65..66,69..70,72..74,76..77,80,85,87,89..92,99..100,103..105,107,110..113,116} (54 alike) : Scope  NumInputPorts=7
  DS-Bus{1,4,6,8,10,12,15,18..19,24..27,31..32,34,36,40,42,46,49,54..56,59,61..62,65..66,69..70,72..74,76..77,80,85,87,89..92,99..100,103..105,107,110..113,116} (54 alike) : BusSelector  OutputSignals=v_dq,i_dq,v_abc,i_abc,w,theta,pq
  SM1 : SimplusGT/Synchronous Machine (dq-Frame System Object)  Ts=Ts  Sbase=Sbase  Vbase=Vbase  Wbase=Wbase  ApparatusType=ApparatusType{1}  ApparatusPara=ApparatusPara{1}  PowerFlow=ApparatusPowerFlow{1}  x0=x_e{1}  OtherInputs=OtherInputs{1}  DiscreMethod=Hybrid Trapezoidal  EnableInsideModification=off  DiscreDampingFlag=on  DiscreDampingValue=ApparatusDiscreDamping{1}  LinearizationTimes=1  DirectFeedthrough=off
      settings: SourceProductName=Simplus Grid Tool
  SM10 : SimplusGT/Synchronous Machine (dq-Frame System Object)  Ts=Ts  Sbase=Sbase  Vbase=Vbase  Wbase=Wbase  ApparatusType=ApparatusType{10}  ApparatusPara=ApparatusPara{10}  PowerFlow=ApparatusPowerFlow{10}  x0=x_e{10}  OtherInputs=OtherInputs{10}  DiscreMethod=Hybrid Trapezoidal  EnableInsideModification=off  DiscreDampingFlag=on  DiscreDampingValue=ApparatusDiscreDamping{10}  LinearizationTimes=1  DirectFeedthrough=off
      settings: SourceProductName=Simplus Grid Tool
  SM100 : SimplusGT/Synchronous Machine (dq-Frame System Object)  Ts=Ts  Sbase=Sbase  Vbase=Vbase  Wbase=Wbase  ApparatusType=ApparatusType{100}  ApparatusPara=ApparatusPara{100}  PowerFlow=ApparatusPowerFlow{100}  x0=x_e{100}  OtherInputs=OtherInputs{100}  DiscreMethod=Hybrid Trapezoidal  EnableInsideModification=off  DiscreDampingFlag=on  DiscreDampingValue=ApparatusDiscreDamping{100}  LinearizationTimes=1  DirectFeedthrough=off
      settings: SourceProductName=Simplus Grid Tool
  SM103 : SimplusGT/Synchronous Machine (dq-Frame System Object)  Ts=Ts  Sbase=Sbase  Vbase=Vbase  Wbase=Wbase  ApparatusType=ApparatusType{103}  ApparatusPara=ApparatusPara{103}  PowerFlow=ApparatusPowerFlow{103}  x0=x_e{103}  OtherInputs=OtherInputs{103}  DiscreMethod=Hybrid Trapezoidal  EnableInsideModification=off  DiscreDampingFlag=on  DiscreDampingValue=ApparatusDiscreDamping{103}  LinearizationTimes=1  DirectFeedthrough=off
      settings: SourceProductName=Simplus Grid Tool
  SM104 : SimplusGT/Synchronous Machine (dq-Frame System Object)  Ts=Ts  Sbase=Sbase  Vbase=Vbase  Wbase=Wbase  ApparatusType=ApparatusType{104}  ApparatusPara=ApparatusPara{104}  PowerFlow=ApparatusPowerFlow{104}  x0=x_e{104}  OtherInputs=OtherInputs{104}  DiscreMethod=Hybrid Trapezoidal  EnableInsideModification=off  DiscreDampingFlag=on  DiscreDampingValue=ApparatusDiscreDamping{104}  LinearizationTimes=1  DirectFeedthrough=off
      settings: SourceProductName=Simplus Grid Tool
  SM105 : SimplusGT/Synchronous Machine (dq-Frame System Object)  Ts=Ts  Sbase=Sbase  Vbase=Vbase  Wbase=Wbase  ApparatusType=ApparatusType{105}  ApparatusPara=ApparatusPara{105}  PowerFlow=ApparatusPowerFlow{105}  x0=x_e{105}  OtherInputs=OtherInputs{105}  DiscreMethod=Hybrid Trapezoidal  EnableInsideModification=off  DiscreDampingFlag=on  DiscreDampingValue=ApparatusDiscreDamping{105}  LinearizationTimes=1  DirectFeedthrough=off
      settings: SourceProductName=Simplus Grid Tool
  SM107 : SimplusGT/Synchronous Machine (dq-Frame System Object)  Ts=Ts  Sbase=Sbase  Vbase=Vbase  Wbase=Wbase  ApparatusType=ApparatusType{107}  ApparatusPara=ApparatusPara{107}  PowerFlow=ApparatusPowerFlow{107}  x0=x_e{107}  OtherInputs=OtherInputs{107}  DiscreMethod=Hybrid Trapezoidal  EnableInsideModification=off  DiscreDampingFlag=on  DiscreDampingValue=ApparatusDiscreDamping{107}  LinearizationTimes=1  DirectFeedthrough=off
      settings: SourceProductName=Simplus Grid Tool
  SM110 : SimplusGT/Synchronous Machine (dq-Frame System Object)  Ts=Ts  Sbase=Sbase  Vbase=Vbase  Wbase=Wbase  ApparatusType=ApparatusType{110}  ApparatusPara=ApparatusPara{110}  PowerFlow=ApparatusPowerFlow{110}  x0=x_e{110}  OtherInputs=OtherInputs{110}  DiscreMethod=Hybrid Trapezoidal  EnableInsideModification=off  DiscreDampingFlag=on  DiscreDampingValue=ApparatusDiscreDamping{110}  LinearizationTimes=1  DirectFeedthrough=off
      settings: SourceProductName=Simplus Grid Tool
  SM111 : SimplusGT/Synchronous Machine (dq-Frame System Object)  Ts=Ts  Sbase=Sbase  Vbase=Vbase  Wbase=Wbase  ApparatusType=ApparatusType{111}  ApparatusPara=ApparatusPara{111}  PowerFlow=ApparatusPowerFlow{111}  x0=x_e{111}  OtherInputs=OtherInputs{111}  DiscreMethod=Hybrid Trapezoidal  EnableInsideModification=off  DiscreDampingFlag=on  DiscreDampingValue=ApparatusDiscreDamping{111}  LinearizationTimes=1  DirectFeedthrough=off
      settings: SourceProductName=Simplus Grid Tool
  SM112 : SimplusGT/Synchronous Machine (dq-Frame System Object)  Ts=Ts  Sbase=Sbase  Vbase=Vbase  Wbase=Wbase  ApparatusType=ApparatusType{112}  ApparatusPara=ApparatusPara{112}  PowerFlow=ApparatusPowerFlow{112}  x0=x_e{112}  OtherInputs=OtherInputs{112}  DiscreMethod=Hybrid Trapezoidal  EnableInsideModification=off  DiscreDampingFlag=on  DiscreDampingValue=ApparatusDiscreDamping{112}  LinearizationTimes=1  DirectFeedthrough=off
      settings: SourceProductName=Simplus Grid Tool
  SM113 : SimplusGT/Synchronous Machine (dq-Frame System Object)  Ts=Ts  Sbase=Sbase  Vbase=Vbase  Wbase=Wbase  ApparatusType=ApparatusType{113}  ApparatusPara=ApparatusPara{113}  PowerFlow=ApparatusPowerFlow{113}  x0=x_e{113}  OtherInputs=OtherInputs{113}  DiscreMethod=Hybrid Trapezoidal  EnableInsideModification=off  DiscreDampingFlag=on  DiscreDampingValue=ApparatusDiscreDamping{113}  LinearizationTimes=1  DirectFeedthrough=off
      settings: SourceProductName=Simplus Grid Tool
  SM116 : SimplusGT/Synchronous Machine (dq-Frame System Object)  Ts=Ts  Sbase=Sbase  Vbase=Vbase  Wbase=Wbase  ApparatusType=ApparatusType{116}  ApparatusPara=ApparatusPara{116}  PowerFlow=ApparatusPowerFlow{116}  x0=x_e{116}  OtherInputs=OtherInputs{116}  DiscreMethod=Hybrid Trapezoidal  EnableInsideModification=off  DiscreDampingFlag=on  DiscreDampingValue=ApparatusDiscreDamping{116}  LinearizationTimes=1  DirectFeedthrough=off
      settings: SourceProductName=Simplus Grid Tool
  SM12 : SimplusGT/Synchronous Machine (dq-Frame System Object)  Ts=Ts  Sbase=Sbase  Vbase=Vbase  Wbase=Wbase  ApparatusType=ApparatusType{12}  ApparatusPara=ApparatusPara{12}  PowerFlow=ApparatusPowerFlow{12}  x0=x_e{12}  OtherInputs=OtherInputs{12}  DiscreMethod=Hybrid Trapezoidal  EnableInsideModification=off  DiscreDampingFlag=on  DiscreDampingValue=ApparatusDiscreDamping{12}  LinearizationTimes=1  DirectFeedthrough=off
      settings: SourceProductName=Simplus Grid Tool
  SM15 : SimplusGT/Synchronous Machine (dq-Frame System Object)  Ts=Ts  Sbase=Sbase  Vbase=Vbase  Wbase=Wbase  ApparatusType=ApparatusType{15}  ApparatusPara=ApparatusPara{15}  PowerFlow=ApparatusPowerFlow{15}  x0=x_e{15}  OtherInputs=OtherInputs{15}  DiscreMethod=Hybrid Trapezoidal  EnableInsideModification=off  DiscreDampingFlag=on  DiscreDampingValue=ApparatusDiscreDamping{15}  LinearizationTimes=1  DirectFeedthrough=off
      settings: SourceProductName=Simplus Grid Tool
  SM18 : SimplusGT/Synchronous Machine (dq-Frame System Object)  Ts=Ts  Sbase=Sbase  Vbase=Vbase  Wbase=Wbase  ApparatusType=ApparatusType{18}  ApparatusPara=ApparatusPara{18}  PowerFlow=ApparatusPowerFlow{18}  x0=x_e{18}  OtherInputs=OtherInputs{18}  DiscreMethod=Hybrid Trapezoidal  EnableInsideModification=off  DiscreDampingFlag=on  DiscreDampingValue=ApparatusDiscreDamping{18}  LinearizationTimes=1  DirectFeedthrough=off
      settings: SourceProductName=Simplus Grid Tool
  SM19 : SimplusGT/Synchronous Machine (dq-Frame System Object)  Ts=Ts  Sbase=Sbase  Vbase=Vbase  Wbase=Wbase  ApparatusType=ApparatusType{19}  ApparatusPara=ApparatusPara{19}  PowerFlow=ApparatusPowerFlow{19}  x0=x_e{19}  OtherInputs=OtherInputs{19}  DiscreMethod=Hybrid Trapezoidal  EnableInsideModification=off  DiscreDampingFlag=on  DiscreDampingValue=ApparatusDiscreDamping{19}  LinearizationTimes=1  DirectFeedthrough=off
      settings: SourceProductName=Simplus Grid Tool
  SM24 : SimplusGT/Synchronous Machine (dq-Frame System Object)  Ts=Ts  Sbase=Sbase  Vbase=Vbase  Wbase=Wbase  ApparatusType=ApparatusType{24}  ApparatusPara=ApparatusPara{24}  PowerFlow=ApparatusPowerFlow{24}  x0=x_e{24}  OtherInputs=OtherInputs{24}  DiscreMethod=Hybrid Trapezoidal  EnableInsideModification=off  DiscreDampingFlag=on  DiscreDampingValue=ApparatusDiscreDamping{24}  LinearizationTimes=1  DirectFeedthrough=off
      settings: SourceProductName=Simplus Grid Tool
  SM25 : SimplusGT/Synchronous Machine (dq-Frame System Object)  Ts=Ts  Sbase=Sbase  Vbase=Vbase  Wbase=Wbase  ApparatusType=ApparatusType{25}  ApparatusPara=ApparatusPara{25}  PowerFlow=ApparatusPowerFlow{25}  x0=x_e{25}  OtherInputs=OtherInputs{25}  DiscreMethod=Hybrid Trapezoidal  EnableInsideModification=off  DiscreDampingFlag=on  DiscreDampingValue=ApparatusDiscreDamping{25}  LinearizationTimes=1  DirectFeedthrough=off
      settings: SourceProductName=Simplus Grid Tool
  SM26 : SimplusGT/Synchronous Machine (dq-Frame System Object)  Ts=Ts  Sbase=Sbase  Vbase=Vbase  Wbase=Wbase  ApparatusType=ApparatusType{26}  ApparatusPara=ApparatusPara{26}  PowerFlow=ApparatusPowerFlow{26}  x0=x_e{26}  OtherInputs=OtherInputs{26}  DiscreMethod=Hybrid Trapezoidal  EnableInsideModification=off  DiscreDampingFlag=on  DiscreDampingValue=ApparatusDiscreDamping{26}  LinearizationTimes=1  DirectFeedthrough=off
      settings: SourceProductName=Simplus Grid Tool
  SM27 : SimplusGT/Synchronous Machine (dq-Frame System Object)  Ts=Ts  Sbase=Sbase  Vbase=Vbase  Wbase=Wbase  ApparatusType=ApparatusType{27}  ApparatusPara=ApparatusPara{27}  PowerFlow=ApparatusPowerFlow{27}  x0=x_e{27}  OtherInputs=OtherInputs{27}  DiscreMethod=Hybrid Trapezoidal  EnableInsideModification=off  DiscreDampingFlag=on  DiscreDampingValue=ApparatusDiscreDamping{27}  LinearizationTimes=1  DirectFeedthrough=off
      settings: SourceProductName=Simplus Grid Tool
  SM31 : SimplusGT/Synchronous Machine (dq-Frame System Object)  Ts=Ts  Sbase=Sbase  Vbase=Vbase  Wbase=Wbase  ApparatusType=ApparatusType{31}  ApparatusPara=ApparatusPara{31}  PowerFlow=ApparatusPowerFlow{31}  x0=x_e{31}  OtherInputs=OtherInputs{31}  DiscreMethod=Hybrid Trapezoidal  EnableInsideModification=off  DiscreDampingFlag=on  DiscreDampingValue=ApparatusDiscreDamping{31}  LinearizationTimes=1  DirectFeedthrough=off
      settings: SourceProductName=Simplus Grid Tool
  SM32 : SimplusGT/Synchronous Machine (dq-Frame System Object)  Ts=Ts  Sbase=Sbase  Vbase=Vbase  Wbase=Wbase  ApparatusType=ApparatusType{32}  ApparatusPara=ApparatusPara{32}  PowerFlow=ApparatusPowerFlow{32}  x0=x_e{32}  OtherInputs=OtherInputs{32}  DiscreMethod=Hybrid Trapezoidal  EnableInsideModification=off  DiscreDampingFlag=on  DiscreDampingValue=ApparatusDiscreDamping{32}  LinearizationTimes=1  DirectFeedthrough=off
      settings: SourceProductName=Simplus Grid Tool
  SM34 : SimplusGT/Synchronous Machine (dq-Frame System Object)  Ts=Ts  Sbase=Sbase  Vbase=Vbase  Wbase=Wbase  ApparatusType=ApparatusType{34}  ApparatusPara=ApparatusPara{34}  PowerFlow=ApparatusPowerFlow{34}  x0=x_e{34}  OtherInputs=OtherInputs{34}  DiscreMethod=Hybrid Trapezoidal  EnableInsideModification=off  DiscreDampingFlag=on  DiscreDampingValue=ApparatusDiscreDamping{34}  LinearizationTimes=1  DirectFeedthrough=off
      settings: SourceProductName=Simplus Grid Tool
  SM36 : SimplusGT/Synchronous Machine (dq-Frame System Object)  Ts=Ts  Sbase=Sbase  Vbase=Vbase  Wbase=Wbase  ApparatusType=ApparatusType{36}  ApparatusPara=ApparatusPara{36}  PowerFlow=ApparatusPowerFlow{36}  x0=x_e{36}  OtherInputs=OtherInputs{36}  DiscreMethod=Hybrid Trapezoidal  EnableInsideModification=off  DiscreDampingFlag=on  DiscreDampingValue=ApparatusDiscreDamping{36}  LinearizationTimes=1  DirectFeedthrough=off
      settings: SourceProductName=Simplus Grid Tool
  SM4 : SimplusGT/Synchronous Machine (dq-Frame System Object)  Ts=Ts  Sbase=Sbase  Vbase=Vbase  Wbase=Wbase  ApparatusType=ApparatusType{4}  ApparatusPara=ApparatusPara{4}  PowerFlow=ApparatusPowerFlow{4}  x0=x_e{4}  OtherInputs=OtherInputs{4}  DiscreMethod=Hybrid Trapezoidal  EnableInsideModification=off  DiscreDampingFlag=on  DiscreDampingValue=ApparatusDiscreDamping{4}  LinearizationTimes=1  DirectFeedthrough=off
      settings: SourceProductName=Simplus Grid Tool
  SM40 : SimplusGT/Synchronous Machine (dq-Frame System Object)  Ts=Ts  Sbase=Sbase  Vbase=Vbase  Wbase=Wbase  ApparatusType=ApparatusType{40}  ApparatusPara=ApparatusPara{40}  PowerFlow=ApparatusPowerFlow{40}  x0=x_e{40}  OtherInputs=OtherInputs{40}  DiscreMethod=Hybrid Trapezoidal  EnableInsideModification=off  DiscreDampingFlag=on  DiscreDampingValue=ApparatusDiscreDamping{40}  LinearizationTimes=1  DirectFeedthrough=off
      settings: SourceProductName=Simplus Grid Tool
  SM42 : SimplusGT/Synchronous Machine (dq-Frame System Object)  Ts=Ts  Sbase=Sbase  Vbase=Vbase  Wbase=Wbase  ApparatusType=ApparatusType{42}  ApparatusPara=ApparatusPara{42}  PowerFlow=ApparatusPowerFlow{42}  x0=x_e{42}  OtherInputs=OtherInputs{42}  DiscreMethod=Hybrid Trapezoidal  EnableInsideModification=off  DiscreDampingFlag=on  DiscreDampingValue=ApparatusDiscreDamping{42}  LinearizationTimes=1  DirectFeedthrough=off
      settings: SourceProductName=Simplus Grid Tool
  SM46 : SimplusGT/Synchronous Machine (dq-Frame System Object)  Ts=Ts  Sbase=Sbase  Vbase=Vbase  Wbase=Wbase  ApparatusType=ApparatusType{46}  ApparatusPara=ApparatusPara{46}  PowerFlow=ApparatusPowerFlow{46}  x0=x_e{46}  OtherInputs=OtherInputs{46}  DiscreMethod=Hybrid Trapezoidal  EnableInsideModification=off  DiscreDampingFlag=on  DiscreDampingValue=ApparatusDiscreDamping{46}  LinearizationTimes=1  DirectFeedthrough=off
      settings: SourceProductName=Simplus Grid Tool
  SM49 : SimplusGT/Synchronous Machine (dq-Frame System Object)  Ts=Ts  Sbase=Sbase  Vbase=Vbase  Wbase=Wbase  ApparatusType=ApparatusType{49}  ApparatusPara=ApparatusPara{49}  PowerFlow=ApparatusPowerFlow{49}  x0=x_e{49}  OtherInputs=OtherInputs{49}  DiscreMethod=Hybrid Trapezoidal  EnableInsideModification=off  DiscreDampingFlag=on  DiscreDampingValue=ApparatusDiscreDamping{49}  LinearizationTimes=1  DirectFeedthrough=off
      settings: SourceProductName=Simplus Grid Tool
  SM54 : SimplusGT/Synchronous Machine (dq-Frame System Object)  Ts=Ts  Sbase=Sbase  Vbase=Vbase  Wbase=Wbase  ApparatusType=ApparatusType{54}  ApparatusPara=ApparatusPara{54}  PowerFlow=ApparatusPowerFlow{54}  x0=x_e{54}  OtherInputs=OtherInputs{54}  DiscreMethod=Hybrid Trapezoidal  EnableInsideModification=off  DiscreDampingFlag=on  DiscreDampingValue=ApparatusDiscreDamping{54}  LinearizationTimes=1  DirectFeedthrough=off
      settings: SourceProductName=Simplus Grid Tool
  SM55 : SimplusGT/Synchronous Machine (dq-Frame System Object)  Ts=Ts  Sbase=Sbase  Vbase=Vbase  Wbase=Wbase  ApparatusType=ApparatusType{55}  ApparatusPara=ApparatusPara{55}  PowerFlow=ApparatusPowerFlow{55}  x0=x_e{55}  OtherInputs=OtherInputs{55}  DiscreMethod=Hybrid Trapezoidal  EnableInsideModification=off  DiscreDampingFlag=on  DiscreDampingValue=ApparatusDiscreDamping{55}  LinearizationTimes=1  DirectFeedthrough=off
      settings: SourceProductName=Simplus Grid Tool
  SM56 : SimplusGT/Synchronous Machine (dq-Frame System Object)  Ts=Ts  Sbase=Sbase  Vbase=Vbase  Wbase=Wbase  ApparatusType=ApparatusType{56}  ApparatusPara=ApparatusPara{56}  PowerFlow=ApparatusPowerFlow{56}  x0=x_e{56}  OtherInputs=OtherInputs{56}  DiscreMethod=Hybrid Trapezoidal  EnableInsideModification=off  DiscreDampingFlag=on  DiscreDampingValue=ApparatusDiscreDamping{56}  LinearizationTimes=1  DirectFeedthrough=off
      settings: SourceProductName=Simplus Grid Tool
  SM59 : SimplusGT/Synchronous Machine (dq-Frame System Object)  Ts=Ts  Sbase=Sbase  Vbase=Vbase  Wbase=Wbase  ApparatusType=ApparatusType{59}  ApparatusPara=ApparatusPara{59}  PowerFlow=ApparatusPowerFlow{59}  x0=x_e{59}  OtherInputs=OtherInputs{59}  DiscreMethod=Hybrid Trapezoidal  EnableInsideModification=off  DiscreDampingFlag=on  DiscreDampingValue=ApparatusDiscreDamping{59}  LinearizationTimes=1  DirectFeedthrough=off
      settings: SourceProductName=Simplus Grid Tool
  SM6 : SimplusGT/Synchronous Machine (dq-Frame System Object)  Ts=Ts  Sbase=Sbase  Vbase=Vbase  Wbase=Wbase  ApparatusType=ApparatusType{6}  ApparatusPara=ApparatusPara{6}  PowerFlow=ApparatusPowerFlow{6}  x0=x_e{6}  OtherInputs=OtherInputs{6}  DiscreMethod=Hybrid Trapezoidal  EnableInsideModification=off  DiscreDampingFlag=on  DiscreDampingValue=ApparatusDiscreDamping{6}  LinearizationTimes=1  DirectFeedthrough=off
      settings: SourceProductName=Simplus Grid Tool
  SM61 : SimplusGT/Synchronous Machine (dq-Frame System Object)  Ts=Ts  Sbase=Sbase  Vbase=Vbase  Wbase=Wbase  ApparatusType=ApparatusType{61}  ApparatusPara=ApparatusPara{61}  PowerFlow=ApparatusPowerFlow{61}  x0=x_e{61}  OtherInputs=OtherInputs{61}  DiscreMethod=Hybrid Trapezoidal  EnableInsideModification=off  DiscreDampingFlag=on  DiscreDampingValue=ApparatusDiscreDamping{61}  LinearizationTimes=1  DirectFeedthrough=off
      settings: SourceProductName=Simplus Grid Tool
  SM62 : SimplusGT/Synchronous Machine (dq-Frame System Object)  Ts=Ts  Sbase=Sbase  Vbase=Vbase  Wbase=Wbase  ApparatusType=ApparatusType{62}  ApparatusPara=ApparatusPara{62}  PowerFlow=ApparatusPowerFlow{62}  x0=x_e{62}  OtherInputs=OtherInputs{62}  DiscreMethod=Hybrid Trapezoidal  EnableInsideModification=off  DiscreDampingFlag=on  DiscreDampingValue=ApparatusDiscreDamping{62}  LinearizationTimes=1  DirectFeedthrough=off
      settings: SourceProductName=Simplus Grid Tool
  SM65 : SimplusGT/Synchronous Machine (dq-Frame System Object)  Ts=Ts  Sbase=Sbase  Vbase=Vbase  Wbase=Wbase  ApparatusType=ApparatusType{65}  ApparatusPara=ApparatusPara{65}  PowerFlow=ApparatusPowerFlow{65}  x0=x_e{65}  OtherInputs=OtherInputs{65}  DiscreMethod=Hybrid Trapezoidal  EnableInsideModification=off  DiscreDampingFlag=on  DiscreDampingValue=ApparatusDiscreDamping{65}  LinearizationTimes=1  DirectFeedthrough=off
      settings: SourceProductName=Simplus Grid Tool
  SM66 : SimplusGT/Synchronous Machine (dq-Frame System Object)  Ts=Ts  Sbase=Sbase  Vbase=Vbase  Wbase=Wbase  ApparatusType=ApparatusType{66}  ApparatusPara=ApparatusPara{66}  PowerFlow=ApparatusPowerFlow{66}  x0=x_e{66}  OtherInputs=OtherInputs{66}  DiscreMethod=Hybrid Trapezoidal  EnableInsideModification=off  DiscreDampingFlag=on  DiscreDampingValue=ApparatusDiscreDamping{66}  LinearizationTimes=1  DirectFeedthrough=off
      settings: SourceProductName=Simplus Grid Tool
  SM69 : SimplusGT/Synchronous Machine (dq-Frame System Object)  Ts=Ts  Sbase=Sbase  Vbase=Vbase  Wbase=Wbase  ApparatusType=ApparatusType{69}  ApparatusPara=ApparatusPara{69}  PowerFlow=ApparatusPowerFlow{69}  x0=x_e{69}  OtherInputs=OtherInputs{69}  DiscreMethod=Hybrid Trapezoidal  EnableInsideModification=off  DiscreDampingFlag=on  DiscreDampingValue=ApparatusDiscreDamping{69}  LinearizationTimes=1  DirectFeedthrough=off
      settings: SourceProductName=Simplus Grid Tool
  SM70 : SimplusGT/Synchronous Machine (dq-Frame System Object)  Ts=Ts  Sbase=Sbase  Vbase=Vbase  Wbase=Wbase  ApparatusType=ApparatusType{70}  ApparatusPara=ApparatusPara{70}  PowerFlow=ApparatusPowerFlow{70}  x0=x_e{70}  OtherInputs=OtherInputs{70}  DiscreMethod=Hybrid Trapezoidal  EnableInsideModification=off  DiscreDampingFlag=on  DiscreDampingValue=ApparatusDiscreDamping{70}  LinearizationTimes=1  DirectFeedthrough=off
      settings: SourceProductName=Simplus Grid Tool
  SM72 : SimplusGT/Synchronous Machine (dq-Frame System Object)  Ts=Ts  Sbase=Sbase  Vbase=Vbase  Wbase=Wbase  ApparatusType=ApparatusType{72}  ApparatusPara=ApparatusPara{72}  PowerFlow=ApparatusPowerFlow{72}  x0=x_e{72}  OtherInputs=OtherInputs{72}  DiscreMethod=Hybrid Trapezoidal  EnableInsideModification=off  DiscreDampingFlag=on  DiscreDampingValue=ApparatusDiscreDamping{72}  LinearizationTimes=1  DirectFeedthrough=off
      settings: SourceProductName=Simplus Grid Tool
  SM73 : SimplusGT/Synchronous Machine (dq-Frame System Object)  Ts=Ts  Sbase=Sbase  Vbase=Vbase  Wbase=Wbase  ApparatusType=ApparatusType{73}  ApparatusPara=ApparatusPara{73}  PowerFlow=ApparatusPowerFlow{73}  x0=x_e{73}  OtherInputs=OtherInputs{73}  DiscreMethod=Hybrid Trapezoidal  EnableInsideModification=off  DiscreDampingFlag=on  DiscreDampingValue=ApparatusDiscreDamping{73}  LinearizationTimes=1  DirectFeedthrough=off
      settings: SourceProductName=Simplus Grid Tool
  SM74 : SimplusGT/Synchronous Machine (dq-Frame System Object)  Ts=Ts  Sbase=Sbase  Vbase=Vbase  Wbase=Wbase  ApparatusType=ApparatusType{74}  ApparatusPara=ApparatusPara{74}  PowerFlow=ApparatusPowerFlow{74}  x0=x_e{74}  OtherInputs=OtherInputs{74}  DiscreMethod=Hybrid Trapezoidal  EnableInsideModification=off  DiscreDampingFlag=on  DiscreDampingValue=ApparatusDiscreDamping{74}  LinearizationTimes=1  DirectFeedthrough=off
      settings: SourceProductName=Simplus Grid Tool
  SM76 : SimplusGT/Synchronous Machine (dq-Frame System Object)  Ts=Ts  Sbase=Sbase  Vbase=Vbase  Wbase=Wbase  ApparatusType=ApparatusType{76}  ApparatusPara=ApparatusPara{76}  PowerFlow=ApparatusPowerFlow{76}  x0=x_e{76}  OtherInputs=OtherInputs{76}  DiscreMethod=Hybrid Trapezoidal  EnableInsideModification=off  DiscreDampingFlag=on  DiscreDampingValue=ApparatusDiscreDamping{76}  LinearizationTimes=1  DirectFeedthrough=off
      settings: SourceProductName=Simplus Grid Tool
  SM77 : SimplusGT/Synchronous Machine (dq-Frame System Object)  Ts=Ts  Sbase=Sbase  Vbase=Vbase  Wbase=Wbase  ApparatusType=ApparatusType{77}  ApparatusPara=ApparatusPara{77}  PowerFlow=ApparatusPowerFlow{77}  x0=x_e{77}  OtherInputs=OtherInputs{77}  DiscreMethod=Hybrid Trapezoidal  EnableInsideModification=off  DiscreDampingFlag=on  DiscreDampingValue=ApparatusDiscreDamping{77}  LinearizationTimes=1  DirectFeedthrough=off
      settings: SourceProductName=Simplus Grid Tool
  SM8 : SimplusGT/Synchronous Machine (dq-Frame System Object)  Ts=Ts  Sbase=Sbase  Vbase=Vbase  Wbase=Wbase  ApparatusType=ApparatusType{8}  ApparatusPara=ApparatusPara{8}  PowerFlow=ApparatusPowerFlow{8}  x0=x_e{8}  OtherInputs=OtherInputs{8}  DiscreMethod=Hybrid Trapezoidal  EnableInsideModification=off  DiscreDampingFlag=on  DiscreDampingValue=ApparatusDiscreDamping{8}  LinearizationTimes=1  DirectFeedthrough=off
      settings: SourceProductName=Simplus Grid Tool
  SM80 : SimplusGT/Synchronous Machine (dq-Frame System Object)  Ts=Ts  Sbase=Sbase  Vbase=Vbase  Wbase=Wbase  ApparatusType=ApparatusType{80}  ApparatusPara=ApparatusPara{80}  PowerFlow=ApparatusPowerFlow{80}  x0=x_e{80}  OtherInputs=OtherInputs{80}  DiscreMethod=Hybrid Trapezoidal  EnableInsideModification=off  DiscreDampingFlag=on  DiscreDampingValue=ApparatusDiscreDamping{80}  LinearizationTimes=1  DirectFeedthrough=off
      settings: SourceProductName=Simplus Grid Tool
  SM85 : SimplusGT/Synchronous Machine (dq-Frame System Object)  Ts=Ts  Sbase=Sbase  Vbase=Vbase  Wbase=Wbase  ApparatusType=ApparatusType{85}  ApparatusPara=ApparatusPara{85}  PowerFlow=ApparatusPowerFlow{85}  x0=x_e{85}  OtherInputs=OtherInputs{85}  DiscreMethod=Hybrid Trapezoidal  EnableInsideModification=off  DiscreDampingFlag=on  DiscreDampingValue=ApparatusDiscreDamping{85}  LinearizationTimes=1  DirectFeedthrough=off
      settings: SourceProductName=Simplus Grid Tool
  SM87 : SimplusGT/Synchronous Machine (dq-Frame System Object)  Ts=Ts  Sbase=Sbase  Vbase=Vbase  Wbase=Wbase  ApparatusType=ApparatusType{87}  ApparatusPara=ApparatusPara{87}  PowerFlow=ApparatusPowerFlow{87}  x0=x_e{87}  OtherInputs=OtherInputs{87}  DiscreMethod=Hybrid Trapezoidal  EnableInsideModification=off  DiscreDampingFlag=on  DiscreDampingValue=ApparatusDiscreDamping{87}  LinearizationTimes=1  DirectFeedthrough=off
      settings: SourceProductName=Simplus Grid Tool
  SM89 : SimplusGT/Synchronous Machine (dq-Frame System Object)  Ts=Ts  Sbase=Sbase  Vbase=Vbase  Wbase=Wbase  ApparatusType=ApparatusType{89}  ApparatusPara=ApparatusPara{89}  PowerFlow=ApparatusPowerFlow{89}  x0=x_e{89}  OtherInputs=OtherInputs{89}  DiscreMethod=Hybrid Trapezoidal  EnableInsideModification=off  DiscreDampingFlag=on  DiscreDampingValue=ApparatusDiscreDamping{89}  LinearizationTimes=1  DirectFeedthrough=off
      settings: SourceProductName=Simplus Grid Tool
  SM90 : SimplusGT/Synchronous Machine (dq-Frame System Object)  Ts=Ts  Sbase=Sbase  Vbase=Vbase  Wbase=Wbase  ApparatusType=ApparatusType{90}  ApparatusPara=ApparatusPara{90}  PowerFlow=ApparatusPowerFlow{90}  x0=x_e{90}  OtherInputs=OtherInputs{90}  DiscreMethod=Hybrid Trapezoidal  EnableInsideModification=off  DiscreDampingFlag=on  DiscreDampingValue=ApparatusDiscreDamping{90}  LinearizationTimes=1  DirectFeedthrough=off
      settings: SourceProductName=Simplus Grid Tool
  SM91 : SimplusGT/Synchronous Machine (dq-Frame System Object)  Ts=Ts  Sbase=Sbase  Vbase=Vbase  Wbase=Wbase  ApparatusType=ApparatusType{91}  ApparatusPara=ApparatusPara{91}  PowerFlow=ApparatusPowerFlow{91}  x0=x_e{91}  OtherInputs=OtherInputs{91}  DiscreMethod=Hybrid Trapezoidal  EnableInsideModification=off  DiscreDampingFlag=on  DiscreDampingValue=ApparatusDiscreDamping{91}  LinearizationTimes=1  DirectFeedthrough=off
      settings: SourceProductName=Simplus Grid Tool
  SM92 : SimplusGT/Synchronous Machine (dq-Frame System Object)  Ts=Ts  Sbase=Sbase  Vbase=Vbase  Wbase=Wbase  ApparatusType=ApparatusType{92}  ApparatusPara=ApparatusPara{92}  PowerFlow=ApparatusPowerFlow{92}  x0=x_e{92}  OtherInputs=OtherInputs{92}  DiscreMethod=Hybrid Trapezoidal  EnableInsideModification=off  DiscreDampingFlag=on  DiscreDampingValue=ApparatusDiscreDamping{92}  LinearizationTimes=1  DirectFeedthrough=off
      settings: SourceProductName=Simplus Grid Tool
  SM99 : SimplusGT/Synchronous Machine (dq-Frame System Object)  Ts=Ts  Sbase=Sbase  Vbase=Vbase  Wbase=Wbase  ApparatusType=ApparatusType{99}  ApparatusPara=ApparatusPara{99}  PowerFlow=ApparatusPowerFlow{99}  x0=x_e{99}  OtherInputs=OtherInputs{99}  DiscreMethod=Hybrid Trapezoidal  EnableInsideModification=off  DiscreDampingFlag=on  DiscreDampingValue=ApparatusDiscreDamping{99}  LinearizationTimes=1  DirectFeedthrough=off
      settings: SourceProductName=Simplus Grid Tool
  Transformer1-68 : powerlib/Elements/Three-Phase Transformer (Two Windings)  Winding1Connection=Yg  Winding2Connection=Yg  CoreType=Three single-phase transformers  SetSaturation=off  Hysteresis=off  DataFile='hysteresis'  SetInitialFlux=off  Measurements=None  UNITS=pu  NominalPower=[Sbase, Fbase]  Winding1=[1.0695*Vbase, 0, 0]  Winding2=[Vbase, 0, 0]  Rm=1e4  Lm=1e4  L0=0.5  Saturation=[ 0,0 ; 0.0024,1.2 ; 1.0,1.52 ]  InitialFluxes=[ 0.8 , -0.8 , 0.7 ]  BreakLoop=off  DiscreteSolver=Trapezoidal iterative  DataType=off  TransfoNumber=1
  Transformer17-30 : powerlib/Elements/Three-Phase Transformer (Two Windings)  Winding1Connection=Yg  Winding2Connection=Yg  CoreType=Three single-phase transformers  SetSaturation=off  Hysteresis=off  DataFile='hysteresis'  SetInitialFlux=off  Measurements=None  UNITS=pu  NominalPower=[Sbase, Fbase]  Winding1=[1.0417*Vbase, 0, 0]  Winding2=[Vbase, 0, 0]  Rm=1e4  Lm=1e4  L0=0.5  Saturation=[ 0,0 ; 0.0024,1.2 ; 1.0,1.52 ]  InitialFluxes=[ 0.8 , -0.8 , 0.7 ]  BreakLoop=off  DiscreteSolver=Trapezoidal iterative  DataType=off  TransfoNumber=1
  Transformer25-26 : powerlib/Elements/Three-Phase Transformer (Two Windings)  Winding1Connection=Yg  Winding2Connection=Yg  CoreType=Three single-phase transformers  SetSaturation=off  Hysteresis=off  DataFile='hysteresis'  SetInitialFlux=off  Measurements=None  UNITS=pu  NominalPower=[Sbase, Fbase]  Winding1=[1.0417*Vbase, 0, 0]  Winding2=[Vbase, 0, 0]  Rm=1e4  Lm=1e4  L0=0.5  Saturation=[ 0,0 ; 0.0024,1.2 ; 1.0,1.52 ]  InitialFluxes=[ 0.8 , -0.8 , 0.7 ]  BreakLoop=off  DiscreteSolver=Trapezoidal iterative  DataType=off  TransfoNumber=1
  Transformer37-38 : powerlib/Elements/Three-Phase Transformer (Two Windings)  Winding1Connection=Yg  Winding2Connection=Yg  CoreType=Three single-phase transformers  SetSaturation=off  Hysteresis=off  DataFile='hysteresis'  SetInitialFlux=off  Measurements=None  UNITS=pu  NominalPower=[Sbase, Fbase]  Winding1=[1.0695*Vbase, 0, 0]  Winding2=[Vbase, 0, 0]  Rm=1e4  Lm=1e4  L0=0.5  Saturation=[ 0,0 ; 0.0024,1.2 ; 1.0,1.52 ]  InitialFluxes=[ 0.8 , -0.8 , 0.7 ]  BreakLoop=off  DiscreteSolver=Trapezoidal iterative  DataType=off  TransfoNumber=1
  Transformer5-8 : powerlib/Elements/Three-Phase Transformer (Two Windings)  Winding1Connection=Yg  Winding2Connection=Yg  CoreType=Three single-phase transformers  SetSaturation=off  Hysteresis=off  DataFile='hysteresis'  SetInitialFlux=off  Measurements=None  UNITS=pu  NominalPower=[Sbase, Fbase]  Winding1=[1.0152*Vbase, 0, 0]  Winding2=[Vbase, 0, 0]  Rm=1e4  Lm=1e4  L0=0.5  Saturation=[ 0,0 ; 0.0024,1.2 ; 1.0,1.52 ]  InitialFluxes=[ 0.8 , -0.8 , 0.7 ]  BreakLoop=off  DiscreteSolver=Trapezoidal iterative  DataType=off  TransfoNumber=1
  Transformer59-63 : powerlib/Elements/Three-Phase Transformer (Two Windings)  Winding1Connection=Yg  Winding2Connection=Yg  CoreType=Three single-phase transformers  SetSaturation=off  Hysteresis=off  DataFile='hysteresis'  SetInitialFlux=off  Measurements=None  UNITS=pu  NominalPower=[Sbase, Fbase]  Winding1=[1.0417*Vbase, 0, 0]  Winding2=[Vbase, 0, 0]  Rm=1e4  Lm=1e4  L0=0.5  Saturation=[ 0,0 ; 0.0024,1.2 ; 1.0,1.52 ]  InitialFluxes=[ 0.8 , -0.8 , 0.7 ]  BreakLoop=off  DiscreteSolver=Trapezoidal iterative  DataType=off  TransfoNumber=1
  Transformer61-64 : powerlib/Elements/Three-Phase Transformer (Two Windings)  Winding1Connection=Yg  Winding2Connection=Yg  CoreType=Three single-phase transformers  SetSaturation=off  Hysteresis=off  DataFile='hysteresis'  SetInitialFlux=off  Measurements=None  UNITS=pu  NominalPower=[Sbase, Fbase]  Winding1=[1.0152*Vbase, 0, 0]  Winding2=[Vbase, 0, 0]  Rm=1e4  Lm=1e4  L0=0.5  Saturation=[ 0,0 ; 0.0024,1.2 ; 1.0,1.52 ]  InitialFluxes=[ 0.8 , -0.8 , 0.7 ]  BreakLoop=off  DiscreteSolver=Trapezoidal iterative  DataType=off  TransfoNumber=1
  Transformer65-66 : powerlib/Elements/Three-Phase Transformer (Two Windings)  Winding1Connection=Yg  Winding2Connection=Yg  CoreType=Three single-phase transformers  SetSaturation=off  Hysteresis=off  DataFile='hysteresis'  SetInitialFlux=off  Measurements=None  UNITS=pu  NominalPower=[Sbase, Fbase]  Winding1=[0.935*Vbase, 0, 0]  Winding2=[Vbase, 0, 0]  Rm=1e4  Lm=1e4  L0=0.5  Saturation=[ 0,0 ; 0.0024,1.2 ; 1.0,1.52 ]  InitialFluxes=[ 0.8 , -0.8 , 0.7 ]  BreakLoop=off  DiscreteSolver=Trapezoidal iterative  DataType=off  TransfoNumber=1
  Transformer80-81 : powerlib/Elements/Three-Phase Transformer (Two Windings)  Winding1Connection=Yg  Winding2Connection=Yg  CoreType=Three single-phase transformers  SetSaturation=off  Hysteresis=off  DataFile='hysteresis'  SetInitialFlux=off  Measurements=None  UNITS=pu  NominalPower=[Sbase, Fbase]  Winding1=[1.0695*Vbase, 0, 0]  Winding2=[Vbase, 0, 0]  Rm=1e4  Lm=1e4  L0=0.5  Saturation=[ 0,0 ; 0.0024,1.2 ; 1.0,1.52 ]  InitialFluxes=[ 0.8 , -0.8 , 0.7 ]  BreakLoop=off  DiscreteSolver=Trapezoidal iterative  DataType=off  TransfoNumber=1
  powergui : powerlib/powergui  Priority=1  SimulationMode=Discrete  SampleTime=Ts  frequency=60  Iterations=50  frequencyindice=60  Pbase=100e6  ErrMax=1e-4  UnitsV=kV  UnitsW=MW  buscounter=0  FunctionMessages=off  echomessages=off  EnableUseOfTLC=off  CurrentSourceSwitches=off  DisableSnubberDevices=off  DisableRonSwitches=off  DisableVfSwitches=off  DisplayEquations=off  AutomaticDiscreteSolvers=off  SolverType=Tustin/Backward Euler (TBE)  Interpol=off  ExternalGateDelay=off  methode=off  Ts=100  x0status=blocks  SPID=on  SwTol=0  HookPort=off  NonlinearTolerance=1e-4  nMaxIteration=100  ContinueOnMaxIteration=off  RestoreLinks=warning  ResistiveCurrentMeasurement=off  Frange=[0:2:500]  Ylog=off  Xlog=on  ShowGrid=off  save=off  variable=ZData  structure=0  ZoomFFT=off  StartTime=0.0  cycles=1  DisplayStyle=1  fundamental=60  FreqAxis=off  MaxFrequency=1000  frequencyindicesteady=1  RmsSteady=1  display=off
  wires:
  SM1/1 -> DS-Bus1/1
  DS-Bus1/1 -> D-Scope1/1  "<v_dq>"
  DS-Bus1/2 -> D-Scope1/2  "<i_dq>"
  DS-Bus1/3 -> D-Scope1/3  "<v_abc>"
  DS-Bus1/4 -> D-Scope1/4  "<i_abc>"
  DS-Bus1/5 -> D-Scope1/5  "<w>"
  DS-Bus1/6 -> D-Scope1/6  "<theta>"
  DS-Bus1/7 -> D-Scope1/7  "<pq>"
  SM4/1 -> DS-Bus4/1
  DS-Bus4/1 -> D-Scope4/1  "<v_dq>"
  DS-Bus4/2 -> D-Scope4/2  "<i_dq>"
  DS-Bus4/3 -> D-Scope4/3  "<v_abc>"
  DS-Bus4/4 -> D-Scope4/4  "<i_abc>"
  DS-Bus4/5 -> D-Scope4/5  "<w>"
  DS-Bus4/6 -> D-Scope4/6  "<theta>"
  DS-Bus4/7 -> D-Scope4/7  "<pq>"
  SM6/1 -> DS-Bus6/1
  DS-Bus6/1 -> D-Scope6/1  "<v_dq>"
  DS-Bus6/2 -> D-Scope6/2  "<i_dq>"
  DS-Bus6/3 -> D-Scope6/3  "<v_abc>"
  DS-Bus6/4 -> D-Scope6/4  "<i_abc>"
  DS-Bus6/5 -> D-Scope6/5  "<w>"
  DS-Bus6/6 -> D-Scope6/6  "<theta>"
  DS-Bus6/7 -> D-Scope6/7  "<pq>"
  SM8/1 -> DS-Bus8/1
  DS-Bus8/1 -> D-Scope8/1  "<v_dq>"
  DS-Bus8/2 -> D-Scope8/2  "<i_dq>"
  DS-Bus8/3 -> D-Scope8/3  "<v_abc>"
  DS-Bus8/4 -> D-Scope8/4  "<i_abc>"
  DS-Bus8/5 -> D-Scope8/5  "<w>"
  DS-Bus8/6 -> D-Scope8/6  "<theta>"
  DS-Bus8/7 -> D-Scope8/7  "<pq>"
  SM10/1 -> DS-Bus10/1
  DS-Bus10/1 -> D-Scope10/1  "<v_dq>"
  DS-Bus10/2 -> D-Scope10/2  "<i_dq>"
  DS-Bus10/3 -> D-Scope10/3  "<v_abc>"
  DS-Bus10/4 -> D-Scope10/4  "<i_abc>"
  DS-Bus10/5 -> D-Scope10/5  "<w>"
  DS-Bus10/6 -> D-Scope10/6  "<theta>"
  DS-Bus10/7 -> D-Scope10/7  "<pq>"
  SM12/1 -> DS-Bus12/1
  DS-Bus12/1 -> D-Scope12/1  "<v_dq>"
  DS-Bus12/2 -> D-Scope12/2  "<i_dq>"
  DS-Bus12/3 -> D-Scope12/3  "<v_abc>"
  DS-Bus12/4 -> D-Scope12/4  "<i_abc>"
  DS-Bus12/5 -> D-Scope12/5  "<w>"
  DS-Bus12/6 -> D-Scope12/6  "<theta>"
  DS-Bus12/7 -> D-Scope12/7  "<pq>"
  SM15/1 -> DS-Bus15/1
  DS-Bus15/1 -> D-Scope15/1  "<v_dq>"
  DS-Bus15/2 -> D-Scope15/2  "<i_dq>"
  DS-Bus15/3 -> D-Scope15/3  "<v_abc>"
  DS-Bus15/4 -> D-Scope15/4  "<i_abc>"
  DS-Bus15/5 -> D-Scope15/5  "<w>"
  DS-Bus15/6 -> D-Scope15/6  "<theta>"
  DS-Bus15/7 -> D-Scope15/7  "<pq>"
  SM18/1 -> DS-Bus18/1
  DS-Bus18/1 -> D-Scope18/1  "<v_dq>"
  DS-Bus18/2 -> D-Scope18/2  "<i_dq>"
  DS-Bus18/3 -> D-Scope18/3  "<v_abc>"
  DS-Bus18/4 -> D-Scope18/4  "<i_abc>"
  DS-Bus18/5 -> D-Scope18/5  "<w>"
  DS-Bus18/6 -> D-Scope18/6  "<theta>"
  DS-Bus18/7 -> D-Scope18/7  "<pq>"
  SM19/1 -> DS-Bus19/1
  DS-Bus19/1 -> D-Scope19/1  "<v_dq>"
  DS-Bus19/2 -> D-Scope19/2  "<i_dq>"
  DS-Bus19/3 -> D-Scope19/3  "<v_abc>"
  DS-Bus19/4 -> D-Scope19/4  "<i_abc>"
  DS-Bus19/5 -> D-Scope19/5  "<w>"
  DS-Bus19/6 -> D-Scope19/6  "<theta>"
  DS-Bus19/7 -> D-Scope19/7  "<pq>"
  SM24/1 -> DS-Bus24/1
  DS-Bus24/1 -> D-Scope24/1  "<v_dq>"
  DS-Bus24/2 -> D-Scope24/2  "<i_dq>"
  DS-Bus24/3 -> D-Scope24/3  "<v_abc>"
  DS-Bus24/4 -> D-Scope24/4  "<i_abc>"
  DS-Bus24/5 -> D-Scope24/5  "<w>"
  DS-Bus24/6 -> D-Scope24/6  "<theta>"
  DS-Bus24/7 -> D-Scope24/7  "<pq>"
  SM25/1 -> DS-Bus25/1
  DS-Bus25/1 -> D-Scope25/1  "<v_dq>"
  DS-Bus25/2 -> D-Scope25/2  "<i_dq>"
  DS-Bus25/3 -> D-Scope25/3  "<v_abc>"
  DS-Bus25/4 -> D-Scope25/4  "<i_abc>"
  DS-Bus25/5 -> D-Scope25/5  "<w>"
  DS-Bus25/6 -> D-Scope25/6  "<theta>"
  DS-Bus25/7 -> D-Scope25/7  "<pq>"
  SM26/1 -> DS-Bus26/1
  DS-Bus26/1 -> D-Scope26/1  "<v_dq>"
  DS-Bus26/2 -> D-Scope26/2  "<i_dq>"
  DS-Bus26/3 -> D-Scope26/3  "<v_abc>"
  DS-Bus26/4 -> D-Scope26/4  "<i_abc>"
  DS-Bus26/5 -> D-Scope26/5  "<w>"
  DS-Bus26/6 -> D-Scope26/6  "<theta>"
  DS-Bus26/7 -> D-Scope26/7  "<pq>"
  SM27/1 -> DS-Bus27/1
  DS-Bus27/1 -> D-Scope27/1  "<v_dq>"
  DS-Bus27/2 -> D-Scope27/2  "<i_dq>"
  DS-Bus27/3 -> D-Scope27/3  "<v_abc>"
  DS-Bus27/4 -> D-Scope27/4  "<i_abc>"
  DS-Bus27/5 -> D-Scope27/5  "<w>"
  DS-Bus27/6 -> D-Scope27/6  "<theta>"
  DS-Bus27/7 -> D-Scope27/7  "<pq>"
  SM31/1 -> DS-Bus31/1
  DS-Bus31/1 -> D-Scope31/1  "<v_dq>"
  DS-Bus31/2 -> D-Scope31/2  "<i_dq>"
  DS-Bus31/3 -> D-Scope31/3  "<v_abc>"
  DS-Bus31/4 -> D-Scope31/4  "<i_abc>"
  DS-Bus31/5 -> D-Scope31/5  "<w>"
  DS-Bus31/6 -> D-Scope31/6  "<theta>"
  DS-Bus31/7 -> D-Scope31/7  "<pq>"
  SM32/1 -> DS-Bus32/1
  DS-Bus32/1 -> D-Scope32/1  "<v_dq>"
  DS-Bus32/2 -> D-Scope32/2  "<i_dq>"
  DS-Bus32/3 -> D-Scope32/3  "<v_abc>"
  DS-Bus32/4 -> D-Scope32/4  "<i_abc>"
  DS-Bus32/5 -> D-Scope32/5  "<w>"
  DS-Bus32/6 -> D-Scope32/6  "<theta>"
  DS-Bus32/7 -> D-Scope32/7  "<pq>"
  SM34/1 -> DS-Bus34/1
  DS-Bus34/1 -> D-Scope34/1  "<v_dq>"
  DS-Bus34/2 -> D-Scope34/2  "<i_dq>"
  DS-Bus34/3 -> D-Scope34/3  "<v_abc>"
  DS-Bus34/4 -> D-Scope34/4  "<i_abc>"
  DS-Bus34/5 -> D-Scope34/5  "<w>"
  DS-Bus34/6 -> D-Scope34/6  "<theta>"
  DS-Bus34/7 -> D-Scope34/7  "<pq>"
  SM36/1 -> DS-Bus36/1
  DS-Bus36/1 -> D-Scope36/1  "<v_dq>"
  DS-Bus36/2 -> D-Scope36/2  "<i_dq>"
  DS-Bus36/3 -> D-Scope36/3  "<v_abc>"
  DS-Bus36/4 -> D-Scope36/4  "<i_abc>"
  DS-Bus36/5 -> D-Scope36/5  "<w>"
  DS-Bus36/6 -> D-Scope36/6  "<theta>"
  DS-Bus36/7 -> D-Scope36/7  "<pq>"
  SM40/1 -> DS-Bus40/1
  DS-Bus40/1 -> D-Scope40/1  "<v_dq>"
  DS-Bus40/2 -> D-Scope40/2  "<i_dq>"
  DS-Bus40/3 -> D-Scope40/3  "<v_abc>"
  DS-Bus40/4 -> D-Scope40/4  "<i_abc>"
  DS-Bus40/5 -> D-Scope40/5  "<w>"
  DS-Bus40/6 -> D-Scope40/6  "<theta>"
  DS-Bus40/7 -> D-Scope40/7  "<pq>"
  SM42/1 -> DS-Bus42/1
  DS-Bus42/1 -> D-Scope42/1  "<v_dq>"
  DS-Bus42/2 -> D-Scope42/2  "<i_dq>"
  DS-Bus42/3 -> D-Scope42/3  "<v_abc>"
  DS-Bus42/4 -> D-Scope42/4  "<i_abc>"
  DS-Bus42/5 -> D-Scope42/5  "<w>"
  DS-Bus42/6 -> D-Scope42/6  "<theta>"
  DS-Bus42/7 -> D-Scope42/7  "<pq>"
  SM46/1 -> DS-Bus46/1
  DS-Bus46/1 -> D-Scope46/1  "<v_dq>"
  DS-Bus46/2 -> D-Scope46/2  "<i_dq>"
  DS-Bus46/3 -> D-Scope46/3  "<v_abc>"
  DS-Bus46/4 -> D-Scope46/4  "<i_abc>"
  DS-Bus46/5 -> D-Scope46/5  "<w>"
  DS-Bus46/6 -> D-Scope46/6  "<theta>"
  DS-Bus46/7 -> D-Scope46/7  "<pq>"
  SM49/1 -> DS-Bus49/1
  DS-Bus49/1 -> D-Scope49/1  "<v_dq>"
  DS-Bus49/2 -> D-Scope49/2  "<i_dq>"
  DS-Bus49/3 -> D-Scope49/3  "<v_abc>"
  DS-Bus49/4 -> D-Scope49/4  "<i_abc>"
  DS-Bus49/5 -> D-Scope49/5  "<w>"
  DS-Bus49/6 -> D-Scope49/6  "<theta>"
  DS-Bus49/7 -> D-Scope49/7  "<pq>"
  SM54/1 -> DS-Bus54/1
  DS-Bus54/1 -> D-Scope54/1  "<v_dq>"
  DS-Bus54/2 -> D-Scope54/2  "<i_dq>"
  DS-Bus54/3 -> D-Scope54/3  "<v_abc>"
  DS-Bus54/4 -> D-Scope54/4  "<i_abc>"
  DS-Bus54/5 -> D-Scope54/5  "<w>"
  DS-Bus54/6 -> D-Scope54/6  "<theta>"
  DS-Bus54/7 -> D-Scope54/7  "<pq>"
  SM55/1 -> DS-Bus55/1
  DS-Bus55/1 -> D-Scope55/1  "<v_dq>"
  DS-Bus55/2 -> D-Scope55/2  "<i_dq>"
  DS-Bus55/3 -> D-Scope55/3  "<v_abc>"
  DS-Bus55/4 -> D-Scope55/4  "<i_abc>"
  DS-Bus55/5 -> D-Scope55/5  "<w>"
  DS-Bus55/6 -> D-Scope55/6  "<theta>"
  DS-Bus55/7 -> D-Scope55/7  "<pq>"
  SM56/1 -> DS-Bus56/1
  DS-Bus56/1 -> D-Scope56/1  "<v_dq>"
  DS-Bus56/2 -> D-Scope56/2  "<i_dq>"
  DS-Bus56/3 -> D-Scope56/3  "<v_abc>"
  DS-Bus56/4 -> D-Scope56/4  "<i_abc>"
  DS-Bus56/5 -> D-Scope56/5  "<w>"
  DS-Bus56/6 -> D-Scope56/6  "<theta>"
  DS-Bus56/7 -> D-Scope56/7  "<pq>"
  SM59/1 -> DS-Bus59/1
  DS-Bus59/1 -> D-Scope59/1  "<v_dq>"
  DS-Bus59/2 -> D-Scope59/2  "<i_dq>"
  DS-Bus59/3 -> D-Scope59/3  "<v_abc>"
  DS-Bus59/4 -> D-Scope59/4  "<i_abc>"
  DS-Bus59/5 -> D-Scope59/5  "<w>"
  DS-Bus59/6 -> D-Scope59/6  "<theta>"
  DS-Bus59/7 -> D-Scope59/7  "<pq>"
  SM61/1 -> DS-Bus61/1
  DS-Bus61/1 -> D-Scope61/1  "<v_dq>"
  DS-Bus61/2 -> D-Scope61/2  "<i_dq>"
  DS-Bus61/3 -> D-Scope61/3  "<v_abc>"
  DS-Bus61/4 -> D-Scope61/4  "<i_abc>"
  DS-Bus61/5 -> D-Scope61/5  "<w>"
  DS-Bus61/6 -> D-Scope61/6  "<theta>"
  DS-Bus61/7 -> D-Scope61/7  "<pq>"
  SM62/1 -> DS-Bus62/1
  DS-Bus62/1 -> D-Scope62/1  "<v_dq>"
  DS-Bus62/2 -> D-Scope62/2  "<i_dq>"
  DS-Bus62/3 -> D-Scope62/3  "<v_abc>"
  DS-Bus62/4 -> D-Scope62/4  "<i_abc>"
  DS-Bus62/5 -> D-Scope62/5  "<w>"
  DS-Bus62/6 -> D-Scope62/6  "<theta>"
  DS-Bus62/7 -> D-Scope62/7  "<pq>"
  SM65/1 -> DS-Bus65/1
  DS-Bus65/1 -> D-Scope65/1  "<v_dq>"
  DS-Bus65/2 -> D-Scope65/2  "<i_dq>"
  DS-Bus65/3 -> D-Scope65/3  "<v_abc>"
  DS-Bus65/4 -> D-Scope65/4  "<i_abc>"
  DS-Bus65/5 -> D-Scope65/5  "<w>"
  DS-Bus65/6 -> D-Scope65/6  "<theta>"
  DS-Bus65/7 -> D-Scope65/7  "<pq>"
  SM66/1 -> DS-Bus66/1
  DS-Bus66/1 -> D-Scope66/1  "<v_dq>"
  DS-Bus66/2 -> D-Scope66/2  "<i_dq>"
  DS-Bus66/3 -> D-Scope66/3  "<v_abc>"
  DS-Bus66/4 -> D-Scope66/4  "<i_abc>"
  DS-Bus66/5 -> D-Scope66/5  "<w>"
  DS-Bus66/6 -> D-Scope66/6  "<theta>"
  DS-Bus66/7 -> D-Scope66/7  "<pq>"
  SM69/1 -> DS-Bus69/1
  DS-Bus69/1 -> D-Scope69/1  "<v_dq>"
  DS-Bus69/2 -> D-Scope69/2  "<i_dq>"
  DS-Bus69/3 -> D-Scope69/3  "<v_abc>"
  DS-Bus69/4 -> D-Scope69/4  "<i_abc>"
  DS-Bus69/5 -> D-Scope69/5  "<w>"
  DS-Bus69/6 -> D-Scope69/6  "<theta>"
  DS-Bus69/7 -> D-Scope69/7  "<pq>"
  SM70/1 -> DS-Bus70/1
  DS-Bus70/1 -> D-Scope70/1  "<v_dq>"
  DS-Bus70/2 -> D-Scope70/2  "<i_dq>"
  DS-Bus70/3 -> D-Scope70/3  "<v_abc>"
  DS-Bus70/4 -> D-Scope70/4  "<i_abc>"
  DS-Bus70/5 -> D-Scope70/5  "<w>"
  DS-Bus70/6 -> D-Scope70/6  "<theta>"
  DS-Bus70/7 -> D-Scope70/7  "<pq>"
  SM72/1 -> DS-Bus72/1
  DS-Bus72/1 -> D-Scope72/1  "<v_dq>"
  DS-Bus72/2 -> D-Scope72/2  "<i_dq>"
  DS-Bus72/3 -> D-Scope72/3  "<v_abc>"
  DS-Bus72/4 -> D-Scope72/4  "<i_abc>"
  DS-Bus72/5 -> D-Scope72/5  "<w>"
  DS-Bus72/6 -> D-Scope72/6  "<theta>"
  DS-Bus72/7 -> D-Scope72/7  "<pq>"
  SM73/1 -> DS-Bus73/1
  DS-Bus73/1 -> D-Scope73/1  "<v_dq>"
  DS-Bus73/2 -> D-Scope73/2  "<i_dq>"
  DS-Bus73/3 -> D-Scope73/3  "<v_abc>"
  DS-Bus73/4 -> D-Scope73/4  "<i_abc>"
  DS-Bus73/5 -> D-Scope73/5  "<w>"
  DS-Bus73/6 -> D-Scope73/6  "<theta>"
  DS-Bus73/7 -> D-Scope73/7  "<pq>"
  SM74/1 -> DS-Bus74/1
  DS-Bus74/1 -> D-Scope74/1  "<v_dq>"
  DS-Bus74/2 -> D-Scope74/2  "<i_dq>"
  DS-Bus74/3 -> D-Scope74/3  "<v_abc>"
  DS-Bus74/4 -> D-Scope74/4  "<i_abc>"
  DS-Bus74/5 -> D-Scope74/5  "<w>"
  DS-Bus74/6 -> D-Scope74/6  "<theta>"
  DS-Bus74/7 -> D-Scope74/7  "<pq>"
  SM76/1 -> DS-Bus76/1
  DS-Bus76/1 -> D-Scope76/1  "<v_dq>"
  DS-Bus76/2 -> D-Scope76/2  "<i_dq>"
  DS-Bus76/3 -> D-Scope76/3  "<v_abc>"
  DS-Bus76/4 -> D-Scope76/4  "<i_abc>"
  DS-Bus76/5 -> D-Scope76/5  "<w>"
  DS-Bus76/6 -> D-Scope76/6  "<theta>"
  DS-Bus76/7 -> D-Scope76/7  "<pq>"
  SM77/1 -> DS-Bus77/1
  DS-Bus77/1 -> D-Scope77/1  "<v_dq>"
  DS-Bus77/2 -> D-Scope77/2  "<i_dq>"
  DS-Bus77/3 -> D-Scope77/3  "<v_abc>"
  DS-Bus77/4 -> D-Scope77/4  "<i_abc>"
  DS-Bus77/5 -> D-Scope77/5  "<w>"
  DS-Bus77/6 -> D-Scope77/6  "<theta>"
  DS-Bus77/7 -> D-Scope77/7  "<pq>"
  SM80/1 -> DS-Bus80/1
  DS-Bus80/1 -> D-Scope80/1  "<v_dq>"
  DS-Bus80/2 -> D-Scope80/2  "<i_dq>"
  DS-Bus80/3 -> D-Scope80/3  "<v_abc>"
  DS-Bus80/4 -> D-Scope80/4  "<i_abc>"
  DS-Bus80/5 -> D-Scope80/5  "<w>"
  DS-Bus80/6 -> D-Scope80/6  "<theta>"
  DS-Bus80/7 -> D-Scope80/7  "<pq>"
  SM85/1 -> DS-Bus85/1
  DS-Bus85/1 -> D-Scope85/1  "<v_dq>"
  DS-Bus85/2 -> D-Scope85/2  "<i_dq>"
  DS-Bus85/3 -> D-Scope85/3  "<v_abc>"
  DS-Bus85/4 -> D-Scope85/4  "<i_abc>"
  DS-Bus85/5 -> D-Scope85/5  "<w>"
  DS-Bus85/6 -> D-Scope85/6  "<theta>"
  DS-Bus85/7 -> D-Scope85/7  "<pq>"
  SM87/1 -> DS-Bus87/1
  DS-Bus87/1 -> D-Scope87/1  "<v_dq>"
  DS-Bus87/2 -> D-Scope87/2  "<i_dq>"
  DS-Bus87/3 -> D-Scope87/3  "<v_abc>"
  DS-Bus87/4 -> D-Scope87/4  "<i_abc>"
  DS-Bus87/5 -> D-Scope87/5  "<w>"
  DS-Bus87/6 -> D-Scope87/6  "<theta>"
  DS-Bus87/7 -> D-Scope87/7  "<pq>"
  SM89/1 -> DS-Bus89/1
  DS-Bus89/1 -> D-Scope89/1  "<v_dq>"
  DS-Bus89/2 -> D-Scope89/2  "<i_dq>"
  DS-Bus89/3 -> D-Scope89/3  "<v_abc>"
  DS-Bus89/4 -> D-Scope89/4  "<i_abc>"
  DS-Bus89/5 -> D-Scope89/5  "<w>"
  DS-Bus89/6 -> D-Scope89/6  "<theta>"
  DS-Bus89/7 -> D-Scope89/7  "<pq>"
  SM90/1 -> DS-Bus90/1
  DS-Bus90/1 -> D-Scope90/1  "<v_dq>"
  DS-Bus90/2 -> D-Scope90/2  "<i_dq>"
  DS-Bus90/3 -> D-Scope90/3  "<v_abc>"
  DS-Bus90/4 -> D-Scope90/4  "<i_abc>"
  DS-Bus90/5 -> D-Scope90/5  "<w>"
  DS-Bus90/6 -> D-Scope90/6  "<theta>"
  DS-Bus90/7 -> D-Scope90/7  "<pq>"
  SM91/1 -> DS-Bus91/1
  DS-Bus91/1 -> D-Scope91/1  "<v_dq>"
  DS-Bus91/2 -> D-Scope91/2  "<i_dq>"
  DS-Bus91/3 -> D-Scope91/3  "<v_abc>"
  DS-Bus91/4 -> D-Scope91/4  "<i_abc>"
  DS-Bus91/5 -> D-Scope91/5  "<w>"
  DS-Bus91/6 -> D-Scope91/6  "<theta>"
  DS-Bus91/7 -> D-Scope91/7  "<pq>"
  SM92/1 -> DS-Bus92/1
  DS-Bus92/1 -> D-Scope92/1  "<v_dq>"
  DS-Bus92/2 -> D-Scope92/2  "<i_dq>"
  DS-Bus92/3 -> D-Scope92/3  "<v_abc>"
  DS-Bus92/4 -> D-Scope92/4  "<i_abc>"
  DS-Bus92/5 -> D-Scope92/5  "<w>"
  DS-Bus92/6 -> D-Scope92/6  "<theta>"
  DS-Bus92/7 -> D-Scope92/7  "<pq>"
  SM99/1 -> DS-Bus99/1
  DS-Bus99/1 -> D-Scope99/1  "<v_dq>"
  DS-Bus99/2 -> D-Scope99/2  "<i_dq>"
  DS-Bus99/3 -> D-Scope99/3  "<v_abc>"
  DS-Bus99/4 -> D-Scope99/4  "<i_abc>"
  DS-Bus99/5 -> D-Scope99/5  "<w>"
  DS-Bus99/6 -> D-Scope99/6  "<theta>"
  DS-Bus99/7 -> D-Scope99/7  "<pq>"
  SM100/1 -> DS-Bus100/1
  DS-Bus100/1 -> D-Scope100/1  "<v_dq>"
  DS-Bus100/2 -> D-Scope100/2  "<i_dq>"
  DS-Bus100/3 -> D-Scope100/3  "<v_abc>"
  DS-Bus100/4 -> D-Scope100/4  "<i_abc>"
  DS-Bus100/5 -> D-Scope100/5  "<w>"
  DS-Bus100/6 -> D-Scope100/6  "<theta>"
  DS-Bus100/7 -> D-Scope100/7  "<pq>"
  SM103/1 -> DS-Bus103/1
  DS-Bus103/1 -> D-Scope103/1  "<v_dq>"
  DS-Bus103/2 -> D-Scope103/2  "<i_dq>"
  DS-Bus103/3 -> D-Scope103/3  "<v_abc>"
  DS-Bus103/4 -> D-Scope103/4  "<i_abc>"
  DS-Bus103/5 -> D-Scope103/5  "<w>"
  DS-Bus103/6 -> D-Scope103/6  "<theta>"
  DS-Bus103/7 -> D-Scope103/7  "<pq>"
  SM104/1 -> DS-Bus104/1
  DS-Bus104/1 -> D-Scope104/1  "<v_dq>"
  DS-Bus104/2 -> D-Scope104/2  "<i_dq>"
  DS-Bus104/3 -> D-Scope104/3  "<v_abc>"
  DS-Bus104/4 -> D-Scope104/4  "<i_abc>"
  DS-Bus104/5 -> D-Scope104/5  "<w>"
  DS-Bus104/6 -> D-Scope104/6  "<theta>"
  DS-Bus104/7 -> D-Scope104/7  "<pq>"
  SM105/1 -> DS-Bus105/1
  DS-Bus105/1 -> D-Scope105/1  "<v_dq>"
  DS-Bus105/2 -> D-Scope105/2  "<i_dq>"
  DS-Bus105/3 -> D-Scope105/3  "<v_abc>"
  DS-Bus105/4 -> D-Scope105/4  "<i_abc>"
  DS-Bus105/5 -> D-Scope105/5  "<w>"
  DS-Bus105/6 -> D-Scope105/6  "<theta>"
  DS-Bus105/7 -> D-Scope105/7  "<pq>"
  SM107/1 -> DS-Bus107/1
  DS-Bus107/1 -> D-Scope107/1  "<v_dq>"
  DS-Bus107/2 -> D-Scope107/2  "<i_dq>"
  DS-Bus107/3 -> D-Scope107/3  "<v_abc>"
  DS-Bus107/4 -> D-Scope107/4  "<i_abc>"
  DS-Bus107/5 -> D-Scope107/5  "<w>"
  DS-Bus107/6 -> D-Scope107/6  "<theta>"
  DS-Bus107/7 -> D-Scope107/7  "<pq>"
  SM110/1 -> DS-Bus110/1
  DS-Bus110/1 -> D-Scope110/1  "<v_dq>"
  DS-Bus110/2 -> D-Scope110/2  "<i_dq>"
  DS-Bus110/3 -> D-Scope110/3  "<v_abc>"
  DS-Bus110/4 -> D-Scope110/4  "<i_abc>"
  DS-Bus110/5 -> D-Scope110/5  "<w>"
  DS-Bus110/6 -> D-Scope110/6  "<theta>"
  DS-Bus110/7 -> D-Scope110/7  "<pq>"
  SM111/1 -> DS-Bus111/1
  DS-Bus111/1 -> D-Scope111/1  "<v_dq>"
  DS-Bus111/2 -> D-Scope111/2  "<i_dq>"
  DS-Bus111/3 -> D-Scope111/3  "<v_abc>"
  DS-Bus111/4 -> D-Scope111/4  "<i_abc>"
  DS-Bus111/5 -> D-Scope111/5  "<w>"
  DS-Bus111/6 -> D-Scope111/6  "<theta>"
  DS-Bus111/7 -> D-Scope111/7  "<pq>"
  SM112/1 -> DS-Bus112/1
  DS-Bus112/1 -> D-Scope112/1  "<v_dq>"
  DS-Bus112/2 -> D-Scope112/2  "<i_dq>"
  DS-Bus112/3 -> D-Scope112/3  "<v_abc>"
  DS-Bus112/4 -> D-Scope112/4  "<i_abc>"
  DS-Bus112/5 -> D-Scope112/5  "<w>"
  DS-Bus112/6 -> D-Scope112/6  "<theta>"
  DS-Bus112/7 -> D-Scope112/7  "<pq>"
  SM113/1 -> DS-Bus113/1
  DS-Bus113/1 -> D-Scope113/1  "<v_dq>"
  DS-Bus113/2 -> D-Scope113/2  "<i_dq>"
  DS-Bus113/3 -> D-Scope113/3  "<v_abc>"
  DS-Bus113/4 -> D-Scope113/4  "<i_abc>"
  DS-Bus113/5 -> D-Scope113/5  "<w>"
  DS-Bus113/6 -> D-Scope113/6  "<theta>"
  DS-Bus113/7 -> D-Scope113/7  "<pq>"
  SM116/1 -> DS-Bus116/1
  DS-Bus116/1 -> D-Scope116/1  "<v_dq>"
  DS-Bus116/2 -> D-Scope116/2  "<i_dq>"
  DS-Bus116/3 -> D-Scope116/3  "<v_abc>"
  DS-Bus116/4 -> D-Scope116/4  "<i_abc>"
  DS-Bus116/5 -> D-Scope116/5  "<w>"
  DS-Bus116/6 -> D-Scope116/6  "<theta>"
  DS-Bus116/7 -> D-Scope116/7  "<pq>"
  connections:
  SM1/LConn4 -- D-GND1/LConn1
  SM4/LConn4 -- D-GND4/LConn1
  SM6/LConn4 -- D-GND6/LConn1
  SM8/LConn4 -- D-GND8/LConn1
  SM10/LConn4 -- D-GND10/LConn1
  SM12/LConn4 -- D-GND12/LConn1
  SM15/LConn4 -- D-GND15/LConn1
  SM18/LConn4 -- D-GND18/LConn1
  SM19/LConn4 -- D-GND19/LConn1
  SM24/LConn4 -- D-GND24/LConn1
  SM25/LConn4 -- D-GND25/LConn1
  SM26/LConn4 -- D-GND26/LConn1
  SM27/LConn4 -- D-GND27/LConn1
  SM31/LConn4 -- D-GND31/LConn1
  SM32/LConn4 -- D-GND32/LConn1
  SM34/LConn4 -- D-GND34/LConn1
  SM36/LConn4 -- D-GND36/LConn1
  SM40/LConn4 -- D-GND40/LConn1
  SM42/LConn4 -- D-GND42/LConn1
  SM46/LConn4 -- D-GND46/LConn1
  SM49/LConn4 -- D-GND49/LConn1
  SM54/LConn4 -- D-GND54/LConn1
  SM55/LConn4 -- D-GND55/LConn1
  SM56/LConn4 -- D-GND56/LConn1
  SM59/LConn4 -- D-GND59/LConn1
  SM61/LConn4 -- D-GND61/LConn1
  SM62/LConn4 -- D-GND62/LConn1
  SM65/LConn4 -- D-GND65/LConn1
  SM66/LConn4 -- D-GND66/LConn1
  SM69/LConn4 -- D-GND69/LConn1
  SM70/LConn4 -- D-GND70/LConn1
  SM72/LConn4 -- D-GND72/LConn1
  SM73/LConn4 -- D-GND73/LConn1
  SM74/LConn4 -- D-GND74/LConn1
  SM76/LConn4 -- D-GND76/LConn1
  SM77/LConn4 -- D-GND77/LConn1
  SM80/LConn4 -- D-GND80/LConn1
  SM85/LConn4 -- D-GND85/LConn1
  SM87/LConn4 -- D-GND87/LConn1
  SM89/LConn4 -- D-GND89/LConn1
  SM90/LConn4 -- D-GND90/LConn1
  SM91/LConn4 -- D-GND91/LConn1
  SM92/LConn4 -- D-GND92/LConn1
  SM99/LConn4 -- D-GND99/LConn1
  SM100/LConn4 -- D-GND100/LConn1
  SM103/LConn4 -- D-GND103/LConn1
  SM104/LConn4 -- D-GND104/LConn1
  SM105/LConn4 -- D-GND105/LConn1
  SM107/LConn4 -- D-GND107/LConn1
  SM110/LConn4 -- D-GND110/LConn1
  SM111/LConn4 -- D-GND111/LConn1
  SM112/LConn4 -- D-GND112/LConn1
  SM113/LConn4 -- D-GND113/LConn1
  SM116/LConn4 -- D-GND116/LConn1
  Branch1-1/RConn1 -- Branch1-1/RConn2 -- Branch1-1/RConn3 -- B-GND1/LConn1
  Branch2-2/RConn1 -- Branch2-2/RConn2 -- Branch2-2/RConn3 -- B-GND8/LConn1
  Branch3-3/RConn1 -- Branch3-3/RConn2 -- Branch3-3/RConn3 -- B-GND11/LConn1
  Branch4-4/RConn1 -- Branch4-4/RConn2 -- Branch4-4/RConn3 -- B-GND15/LConn1
  Branch5-5/RConn1 -- Branch5-5/RConn2 -- Branch5-5/RConn3 -- B-GND18/LConn1
  Branch6-6/RConn1 -- Branch6-6/RConn2 -- Branch6-6/RConn3 -- B-GND22/LConn1
  Branch7-7/RConn1 -- Branch7-7/RConn2 -- Branch7-7/RConn3 -- B-GND24/LConn1
  Branch8-8/RConn1 -- Branch8-8/RConn2 -- Branch8-8/RConn3 -- B-GND26/LConn1
  Branch9-9/RConn1 -- Branch9-9/RConn2 -- Branch9-9/RConn3 -- B-GND29/LConn1
  Branch10-10/RConn1 -- Branch10-10/RConn2 -- Branch10-10/RConn3 -- B-GND31/LConn1
  Branch11-11/RConn1 -- Branch11-11/RConn2 -- Branch11-11/RConn3 -- B-GND32/LConn1
  Branch12-12/RConn1 -- Branch12-12/RConn2 -- Branch12-12/RConn3 -- B-GND35/LConn1
  Branch13-13/RConn1 -- Branch13-13/RConn2 -- Branch13-13/RConn3 -- B-GND39/LConn1
  Branch14-14/RConn1 -- Branch14-14/RConn2 -- Branch14-14/RConn3 -- B-GND41/LConn1
  Branch15-15/RConn1 -- Branch15-15/RConn2 -- Branch15-15/RConn3 -- B-GND43/LConn1
  Branch16-16/RConn1 -- Branch16-16/RConn2 -- Branch16-16/RConn3 -- B-GND47/LConn1
  Branch17-17/RConn1 -- Branch17-17/RConn2 -- Branch17-17/RConn3 -- B-GND49/LConn1
  Branch18-18/RConn1 -- Branch18-18/RConn2 -- Branch18-18/RConn3 -- B-GND54/LConn1
  Branch19-19/RConn1 -- Branch19-19/RConn2 -- Branch19-19/RConn3 -- B-GND56/LConn1
  Branch20-20/RConn1 -- Branch20-20/RConn2 -- Branch20-20/RConn3 -- B-GND59/LConn1
  Branch21-21/RConn1 -- Branch21-21/RConn2 -- Branch21-21/RConn3 -- B-GND61/LConn1
  Branch22-22/RConn1 -- Branch22-22/RConn2 -- Branch22-22/RConn3 -- B-GND63/LConn1
  Branch23-23/RConn1 -- Branch23-23/RConn2 -- Branch23-23/RConn3 -- B-GND65/LConn1
  Branch24-24/RConn1 -- Branch24-24/RConn2 -- Branch24-24/RConn3 -- B-GND69/LConn1
  Branch25-25/RConn1 -- Branch25-25/RConn2 -- Branch25-25/RConn3 -- B-GND72/LConn1
  Branch26-26/RConn1 -- Branch26-26/RConn2 -- Branch26-26/RConn3 -- B-GND75/LConn1
  Branch27-27/RConn1 -- Branch27-27/RConn2 -- Branch27-27/RConn3 -- B-GND77/LConn1
  Branch28-28/RConn1 -- Branch28-28/RConn2 -- Branch28-28/RConn3 -- B-GND81/LConn1
  Branch29-29/RConn1 -- Branch29-29/RConn2 -- Branch29-29/RConn3 -- B-GND83/LConn1
  Branch30-30/RConn1 -- Branch30-30/RConn2 -- Branch30-30/RConn3 -- B-GND85/LConn1
  Branch31-31/RConn1 -- Branch31-31/RConn2 -- Branch31-31/RConn3 -- B-GND87/LConn1
  Branch32-32/RConn1 -- Branch32-32/RConn2 -- Branch32-32/RConn3 -- B-GND89/LConn1
  Branch33-33/RConn1 -- Branch33-33/RConn2 -- Branch33-33/RConn3 -- B-GND92/LConn1
  Branch34-34/RConn1 -- Branch34-34/RConn2 -- Branch34-34/RConn3 -- B-GND94/LConn1
  Branch35-35/RConn1 -- Branch35-35/RConn2 -- Branch35-35/RConn3 -- B-GND98/LConn1
  Branch36-36/RConn1 -- Branch36-36/RConn2 -- Branch36-36/RConn3 -- B-GND101/LConn1
  Branch37-37/RConn1 -- Branch37-37/RConn2 -- Branch37-37/RConn3 -- B-GND102/LConn1
  Branch38-38/RConn1 -- Branch38-38/RConn2 -- Branch38-38/RConn3 -- B-GND106/LConn1
  Branch39-39/RConn1 -- Branch39-39/RConn2 -- Branch39-39/RConn3 -- B-GND108/LConn1
  Branch40-40/RConn1 -- Branch40-40/RConn2 -- Branch40-40/RConn3 -- B-GND110/LConn1
  Branch41-41/RConn1 -- Branch41-41/RConn2 -- Branch41-41/RConn3 -- B-GND113/LConn1
  Branch42-42/RConn1 -- Branch42-42/RConn2 -- Branch42-42/RConn3 -- B-GND115/LConn1
  Branch43-43/RConn1 -- Branch43-43/RConn2 -- Branch43-43/RConn3 -- B-GND118/LConn1
  Branch44-44/RConn1 -- Branch44-44/RConn2 -- Branch44-44/RConn3 -- B-GND120/LConn1
  Branch45-45/RConn1 -- Branch45-45/RConn2 -- Branch45-45/RConn3 -- B-GND122/LConn1
  Branch46-46/RConn1 -- Branch46-46/RConn2 -- Branch46-46/RConn3 -- B-GND125/LConn1
  Branch47-47/RConn1 -- Branch47-47/RConn2 -- Branch47-47/RConn3 -- B-GND128/LConn1
  Branch48-48/RConn1 -- Branch48-48/RConn2 -- Branch48-48/RConn3 -- B-GND130/LConn1
  Branch49-49/RConn1 -- Branch49-49/RConn2 -- Branch49-49/RConn3 -- B-GND132/LConn1
  Branch50-50/RConn1 -- Branch50-50/RConn2 -- Branch50-50/RConn3 -- B-GND139/LConn1
  Branch51-51/RConn1 -- Branch51-51/RConn2 -- Branch51-51/RConn3 -- B-GND141/LConn1
  Branch52-52/RConn1 -- Branch52-52/RConn2 -- Branch52-52/RConn3 -- B-GND144/LConn1
  Branch53-53/RConn1 -- Branch53-53/RConn2 -- Branch53-53/RConn3 -- B-GND146/LConn1
  Branch54-54/RConn1 -- Branch54-54/RConn2 -- Branch54-54/RConn3 -- B-GND148/LConn1
  Branch55-55/RConn1 -- Branch55-55/RConn2 -- Branch55-55/RConn3 -- B-GND152/LConn1
  Branch56-56/RConn1 -- Branch56-56/RConn2 -- Branch56-56/RConn3 -- B-GND155/LConn1
  Branch57-57/RConn1 -- Branch57-57/RConn2 -- Branch57-57/RConn3 -- B-GND160/LConn1
  Branch58-58/RConn1 -- Branch58-58/RConn2 -- Branch58-58/RConn3 -- B-GND161/LConn1
  Branch59-59/RConn1 -- Branch59-59/RConn2 -- Branch59-59/RConn3 -- B-GND162/LConn1
  Branch60-60/RConn1 -- Branch60-60/RConn2 -- Branch60-60/RConn3 -- B-GND166/LConn1
  Branch61-61/RConn1 -- Branch61-61/RConn2 -- Branch61-61/RConn3 -- B-GND169/LConn1
  Branch62-62/RConn1 -- Branch62-62/RConn2 -- Branch62-62/RConn3 -- B-GND172/LConn1
  Branch63-63/RConn1 -- Branch63-63/RConn2 -- Branch63-63/RConn3 -- B-GND175/LConn1
  Branch64-64/RConn1 -- Branch64-64/RConn2 -- Branch64-64/RConn3 -- B-GND177/LConn1
  Branch65-65/RConn1 -- Branch65-65/RConn2 -- Branch65-65/RConn3 -- B-GND179/LConn1
  Branch66-66/RConn1 -- Branch66-66/RConn2 -- Branch66-66/RConn3 -- B-GND182/LConn1
  Branch67-67/RConn1 -- Branch67-67/RConn2 -- Branch67-67/RConn3 -- B-GND184/LConn1
  Branch68-68/RConn1 -- Branch68-68/RConn2 -- Branch68-68/RConn3 -- B-GND185/LConn1
  Branch69-69/RConn1 -- Branch69-69/RConn2 -- Branch69-69/RConn3 -- B-GND188/LConn1
  Branch70-70/RConn1 -- Branch70-70/RConn2 -- Branch70-70/RConn3 -- B-GND189/LConn1
  Branch71-71/RConn1 -- Branch71-71/RConn2 -- Branch71-71/RConn3 -- B-GND193/LConn1
  Branch72-72/RConn1 -- Branch72-72/RConn2 -- Branch72-72/RConn3 -- B-GND196/LConn1
  Branch73-73/RConn1 -- Branch73-73/RConn2 -- Branch73-73/RConn3 -- B-GND197/LConn1
  Branch74-74/RConn1 -- Branch74-74/RConn2 -- Branch74-74/RConn3 -- B-GND198/LConn1
  Branch75-75/RConn1 -- Branch75-75/RConn2 -- Branch75-75/RConn3 -- B-GND200/LConn1
  Branch76-76/RConn1 -- Branch76-76/RConn2 -- Branch76-76/RConn3 -- B-GND203/LConn1
  Branch77-77/RConn1 -- Branch77-77/RConn2 -- Branch77-77/RConn3 -- B-GND206/LConn1
  Branch78-78/RConn1 -- Branch78-78/RConn2 -- Branch78-78/RConn3 -- B-GND211/LConn1
  Branch79-79/RConn1 -- Branch79-79/RConn2 -- Branch79-79/RConn3 -- B-GND213/LConn1
  Branch80-80/RConn1 -- Branch80-80/RConn2 -- Branch80-80/RConn3 -- B-GND215/LConn1
  Branch81-81/RConn1 -- Branch81-81/RConn2 -- Branch81-81/RConn3 -- B-GND221/LConn1
  Branch82-82/RConn1 -- Branch82-82/RConn2 -- Branch82-82/RConn3 -- B-GND222/LConn1
  Branch83-83/RConn1 -- Branch83-83/RConn2 -- Branch83-83/RConn3 -- B-GND225/LConn1
  Branch84-84/RConn1 -- Branch84-84/RConn2 -- Branch84-84/RConn3 -- B-GND228/LConn1
  Branch85-85/RConn1 -- Branch85-85/RConn2 -- Branch85-85/RConn3 -- B-GND230/LConn1
  Branch86-86/RConn1 -- Branch86-86/RConn2 -- Branch86-86/RConn3 -- B-GND234/LConn1
  Branch87-87/RConn1 -- Branch87-87/RConn2 -- Branch87-87/RConn3 -- B-GND236/LConn1
  Branch88-88/RConn1 -- Branch88-88/RConn2 -- Branch88-88/RConn3 -- B-GND237/LConn1
  Branch89-89/RConn1 -- Branch89-89/RConn2 -- Branch89-89/RConn3 -- B-GND239/LConn1
  Branch90-90/RConn1 -- Branch90-90/RConn2 -- Branch90-90/RConn3 -- B-GND244/LConn1
  Branch91-91/RConn1 -- Branch91-91/RConn2 -- Branch91-91/RConn3 -- B-GND246/LConn1
  Branch92-92/RConn1 -- Branch92-92/RConn2 -- Branch92-92/RConn3 -- B-GND248/LConn1
  Branch93-93/RConn1 -- Branch93-93/RConn2 -- Branch93-93/RConn3 -- B-GND253/LConn1
  Branch94-94/RConn1 -- Branch94-94/RConn2 -- Branch94-94/RConn3 -- B-GND255/LConn1
  Branch95-95/RConn1 -- Branch95-95/RConn2 -- Branch95-95/RConn3 -- B-GND259/LConn1
  Branch96-96/RConn1 -- Branch96-96/RConn2 -- Branch96-96/RConn3 -- B-GND261/LConn1
  Branch97-97/RConn1 -- Branch97-97/RConn2 -- Branch97-97/RConn3 -- B-GND263/LConn1
  Branch98-98/RConn1 -- Branch98-98/RConn2 -- Branch98-98/RConn3 -- B-GND264/LConn1
  Branch99-99/RConn1 -- Branch99-99/RConn2 -- Branch99-99/RConn3 -- B-GND266/LConn1
  Branch100-100/RConn1 -- Branch100-100/RConn2 -- Branch100-100/RConn3 -- B-GND268/LConn1
  Branch101-101/RConn1 -- Branch101-101/RConn2 -- Branch101-101/RConn3 -- B-GND273/LConn1
  Branch102-102/RConn1 -- Branch102-102/RConn2 -- Branch102-102/RConn3 -- B-GND275/LConn1
  Branch103-103/RConn1 -- Branch103-103/RConn2 -- Branch103-103/RConn3 -- B-GND276/LConn1
  Branch104-104/RConn1 -- Branch104-104/RConn2 -- Branch104-104/RConn3 -- B-GND280/LConn1
  Branch105-105/RConn1 -- Branch105-105/RConn2 -- Branch105-105/RConn3 -- B-GND282/LConn1
  Branch106-106/RConn1 -- Branch106-106/RConn2 -- Branch106-106/RConn3 -- B-GND286/LConn1
  Branch107-107/RConn1 -- Branch107-107/RConn2 -- Branch107-107/RConn3 -- B-GND288/LConn1
  Branch108-108/RConn1 -- Branch108-108/RConn2 -- Branch108-108/RConn3 -- B-GND289/LConn1
  Branch109-109/RConn1 -- Branch109-109/RConn2 -- Branch109-109/RConn3 -- B-GND291/LConn1
  Branch110-110/RConn1 -- Branch110-110/RConn2 -- Branch110-110/RConn3 -- B-GND293/LConn1
  Branch111-111/RConn1 -- Branch111-111/RConn2 -- Branch111-111/RConn3 -- B-GND296/LConn1
  Branch112-112/RConn1 -- Branch112-112/RConn2 -- Branch112-112/RConn3 -- B-GND297/LConn1
  Branch113-113/RConn1 -- Branch113-113/RConn2 -- Branch113-113/RConn3 -- B-GND298/LConn1
  Branch114-114/RConn1 -- Branch114-114/RConn2 -- Branch114-114/RConn3 -- B-GND299/LConn1
  Branch115-115/RConn1 -- Branch115-115/RConn2 -- Branch115-115/RConn3 -- B-GND301/LConn1
  Branch116-116/RConn1 -- Branch116-116/RConn2 -- Branch116-116/RConn3 -- B-GND302/LConn1
  Branch117-117/RConn1 -- Branch117-117/RConn2 -- Branch117-117/RConn3 -- B-GND303/LConn1
  Branch118-118/RConn1 -- Branch118-118/RConn2 -- Branch118-118/RConn3 -- B-GND304/LConn1
  Branch1-47/RConn1 -- Bus47/RConn1 -- Branch47-47/LConn1 -- Branch47-49/LConn1 -- Branch46-47/RConn1
  Branch1-47/RConn2 -- Bus47/RConn2 -- Branch47-47/LConn2 -- Branch47-49/LConn2 -- Branch46-47/RConn2
  Branch1-47/RConn3 -- Bus47/RConn3 -- Branch47-47/LConn3 -- Branch47-49/LConn3 -- Branch46-47/RConn3
  Branch1-47/LConn1 -- Bus1/RConn1 -- Branch1-1/LConn1 -- Branch1-77/LConn1 -- Branch1-75/LConn1 -- Branch1-70/LConn1 -- Transformer1-68/LConn1 -- Branch1-49/LConn1
  Branch1-47/LConn2 -- Bus1/RConn2 -- Branch1-1/LConn2 -- Branch1-77/LConn2 -- Branch1-75/LConn2 -- Branch1-70/LConn2 -- Transformer1-68/LConn2 -- Branch1-49/LConn2
  Branch1-47/LConn3 -- Bus1/RConn3 -- Branch1-1/LConn3 -- Branch1-77/LConn3 -- Branch1-75/LConn3 -- Branch1-70/LConn3 -- Transformer1-68/LConn3 -- Branch1-49/LConn3
  Branch1-49/RConn1 -- Bus49/RConn1 -- Branch49-49/LConn1 -- Branch49-66_/LConn1 -- Branch49-66/LConn1 -- Branch49-54_/LConn1 -- Branch49-54/LConn1 -- Branch49-51/LConn1 -- Branch49-50/LConn1 -- Branch48-49/RConn1 -- Branch47-49/RConn1 -- Branch45-49/RConn1 -- Branch42-49_/RConn1 -- Branch42-49/RConn1
  Branch1-49/RConn2 -- Bus49/RConn2 -- Branch49-49/LConn2 -- Branch49-66_/LConn2 -- Branch49-66/LConn2 -- Branch49-54_/LConn2 -- Branch49-54/LConn2 -- Branch49-51/LConn2 -- Branch49-50/LConn2 -- Branch48-49/RConn2 -- Branch47-49/RConn2 -- Branch45-49/RConn2 -- Branch42-49_/RConn2 -- Branch42-49/RConn2
  Branch1-49/RConn3 -- Bus49/RConn3 -- Branch49-49/LConn3 -- Branch49-66_/LConn3 -- Branch49-66/LConn3 -- Branch49-54_/LConn3 -- Branch49-54/LConn3 -- Branch49-51/LConn3 -- Branch49-50/LConn3 -- Branch48-49/RConn3 -- Branch47-49/RConn3 -- Branch45-49/RConn3 -- Branch42-49_/RConn3 -- Branch42-49/RConn3
  Branch1-68/RConn1 -- Bus68/RConn1 -- Branch68-68/LConn1 -- Branch68-116/LConn1 -- Branch68-81/LConn1 -- Branch65-68/RConn1
  Branch1-68/RConn2 -- Bus68/RConn2 -- Branch68-68/LConn2 -- Branch68-116/LConn2 -- Branch68-81/LConn2 -- Branch65-68/RConn2
  Branch1-68/RConn3 -- Bus68/RConn3 -- Branch68-68/LConn3 -- Branch68-116/LConn3 -- Branch68-81/LConn3 -- Branch65-68/RConn3
  Transformer1-68/RConn1 -- Branch1-68/LConn1
  Transformer1-68/RConn2 -- Branch1-68/LConn2
  Transformer1-68/RConn3 -- Branch1-68/LConn3
  Branch1-70/RConn1 -- Bus70/RConn1 -- Branch70-70/LConn1 -- Branch70-75/LConn1 -- Branch70-74/LConn1 -- Branch70-71/LConn1 -- Branch24-70/RConn1
  Branch1-70/RConn2 -- Bus70/RConn2 -- Branch70-70/LConn2 -- Branch70-75/LConn2 -- Branch70-74/LConn2 -- Branch70-71/LConn2 -- Branch24-70/RConn2
  Branch1-70/RConn3 -- Bus70/RConn3 -- Branch70-70/LConn3 -- Branch70-75/LConn3 -- Branch70-74/LConn3 -- Branch70-71/LConn3 -- Branch24-70/RConn3
  Branch1-75/RConn1 -- Bus75/RConn1 -- Branch75-75/LConn1 -- Branch75-118/LConn1 -- Branch75-77/LConn1 -- Branch74-75/RConn1 -- Branch70-75/RConn1
  Branch1-75/RConn2 -- Bus75/RConn2 -- Branch75-75/LConn2 -- Branch75-118/LConn2 -- Branch75-77/LConn2 -- Branch74-75/RConn2 -- Branch70-75/RConn2
  Branch1-75/RConn3 -- Bus75/RConn3 -- Branch75-75/LConn3 -- Branch75-118/LConn3 -- Branch75-77/LConn3 -- Branch74-75/RConn3 -- Branch70-75/RConn3
  Branch1-77/RConn1 -- Bus77/RConn1 -- Branch77-77/LConn1 -- Branch77-82/LConn1 -- Branch77-80_/LConn1 -- Branch77-80/LConn1 -- Branch77-78/LConn1 -- Branch76-77/RConn1 -- Branch75-77/RConn1
  Branch1-77/RConn2 -- Bus77/RConn2 -- Branch77-77/LConn2 -- Branch77-82/LConn2 -- Branch77-80_/LConn2 -- Branch77-80/LConn2 -- Branch77-78/LConn2 -- Branch76-77/RConn2 -- Branch75-77/RConn2
  Branch1-77/RConn3 -- Bus77/RConn3 -- Branch77-77/LConn3 -- Branch77-82/LConn3 -- Branch77-80_/LConn3 -- Branch77-80/LConn3 -- Branch77-78/LConn3 -- Branch76-77/RConn3 -- Branch75-77/RConn3
  Branch2-12/RConn1 -- Bus12/RConn1 -- Branch12-12/LConn1 -- Branch12-117/LConn1 -- Branch12-16/LConn1 -- Branch12-14/LConn1 -- Branch11-12/RConn1 -- Branch7-12/RConn1 -- Branch3-12/RConn1
  Branch2-12/RConn2 -- Bus12/RConn2 -- Branch12-12/LConn2 -- Branch12-117/LConn2 -- Branch12-16/LConn2 -- Branch12-14/LConn2 -- Branch11-12/RConn2 -- Branch7-12/RConn2 -- Branch3-12/RConn2
  Branch2-12/RConn3 -- Bus12/RConn3 -- Branch12-12/LConn3 -- Branch12-117/LConn3 -- Branch12-16/LConn3 -- Branch12-14/LConn3 -- Branch11-12/RConn3 -- Branch7-12/RConn3 -- Branch3-12/RConn3
  Branch2-12/LConn1 -- Bus2/RConn1 -- Branch2-2/LConn1 -- Branch2-69/LConn1
  Branch2-12/LConn2 -- Bus2/RConn2 -- Branch2-2/LConn2 -- Branch2-69/LConn2
  Branch2-12/LConn3 -- Bus2/RConn3 -- Branch2-2/LConn3 -- Branch2-69/LConn3
